simulink model "SimulinkAnalysisofCheetahTail"  (R2022a)
(part 8 of 21)

t4317 = ct{1188};
t4318 = ct{1189};
t4319 = ct{1190};
t4320 = ct{1191};
t4321 = ct{1192};
t4322 = ct{1193};
t4323 = ct{1194};
t4324 = ct{1195};
t4326 = ct{1196};
t4327 = ct{1197};
t4329 = ct{1198};
t433 = ct{1199};
t4330 = ct{1200};
t4331 = ct{1201};
t4332 = ct{1202};
t4333 = ct{1203};
t4334 = ct{1204};
t4337 = ct{1205};
t4339 = ct{1206};
t4340 = ct{1207};
t4341 = ct{1208};
t4342 = ct{1209};
t4343 = ct{1210};
t4344 = ct{1211};
t4345 = ct{1212};
t4346 = ct{1213};
t4348 = ct{1214};
t4349 = ct{1215};
t4350 = ct{1216};
t4352 = ct{1217};
t4354 = ct{1218};
t4355 = ct{1219};
t4356 = ct{1220};
t4357 = ct{1221};
t4358 = ct{1222};
t4359 = ct{1223};
t436 = ct{1224};
t4360 = ct{1225};
t4361 = ct{1226};
t4365 = ct{1227};
t4367 = ct{1228};
t4368 = ct{1229};
t4369 = ct{1230};
t4370 = ct{1231};
t4371 = ct{1232};
t4372 = ct{1233};
t4373 = ct{1234};
t4374 = ct{1235};
t4375 = ct{1236};
t4376 = ct{1237};
t4378 = ct{1238};
t4379 = ct{1239};
t4382 = ct{1240};
t4384 = ct{1241};
t4391 = ct{1242};
t4392 = ct{1243};
t4393 = ct{1244};
t4394 = ct{1245};
t4395 = ct{1246};
t4397 = ct{1247};
t4398 = ct{1248};
t4399 = ct{1249};
t44 = ct{1250};
t4400 = ct{1251};
t4401 = ct{1252};
t4402 = ct{1253};
t4403 = ct{1254};
t4404 = ct{1255};
t4406 = ct{1256};
t4407 = ct{1257};
t4408 = ct{1258};
t4409 = ct{1259};
t4412 = ct{1260};
t4414 = ct{1261};
t4415 = ct{1262};
t4416 = ct{1263};
t4418 = ct{1264};
t4420 = ct{1265};
t4421 = ct{1266};
t4422 = ct{1267};
t4424 = ct{1268};
t4425 = ct{1269};
t4427 = ct{1270};
t4428 = ct{1271};
t4429 = ct{1272};
t4431 = ct{1273};
t4432 = ct{1274};
t4434 = ct{1275};
t4435 = ct{1276};
t4437 = ct{1277};
t4438 = ct{1278};
t4439 = ct{1279};
t4440 = ct{1280};
t4442 = ct{1281};
t4443 = ct{1282};
t4444 = ct{1283};
t4447 = ct{1284};
t4448 = ct{1285};
t4449 = ct{1286};
t445 = ct{1287};
t4450 = ct{1288};
t4451 = ct{1289};
t4452 = ct{1290};
t4453 = ct{1291};
t4454 = ct{1292};
t4455 = ct{1293};
t4456 = ct{1294};
t4457 = ct{1295};
t4458 = ct{1296};
t4459 = ct{1297};
t4460 = ct{1298};
t4461 = ct{1299};
t4462 = ct{1300};
t4463 = ct{1301};
t4465 = ct{1302};
t4467 = ct{1303};
t4469 = ct{1304};
t4470 = ct{1305};
t4471 = ct{1306};
t4472 = ct{1307};
t4473 = ct{1308};
t4475 = ct{1309};
t4476 = ct{1310};
t4477 = ct{1311};
t4479 = ct{1312};
t4480 = ct{1313};
t4481 = ct{1314};
t4482 = ct{1315};
t4483 = ct{1316};
t4484 = ct{1317};
t4485 = ct{1318};
t4486 = ct{1319};
t4487 = ct{1320};
t4488 = ct{1321};
t4489 = ct{1322};
t4490 = ct{1323};
t4492 = ct{1324};
t4493 = ct{1325};
t4495 = ct{1326};
t4496 = ct{1327};
t4497 = ct{1328};
t4498 = ct{1329};
t4500 = ct{1330};
t4501 = ct{1331};
t4502 = ct{1332};
t4503 = ct{1333};
t4505 = ct{1334};
t4506 = ct{1335};
t4507 = ct{1336};
t451 = ct{1337};
t4510 = ct{1338};
t4511 = ct{1339};
t4512 = ct{1340};
t4514 = ct{1341};
t4515 = ct{1342};
t4517 = ct{1343};
t4518 = ct{1344};
t4519 = ct{1345};
t4521 = ct{1346};
t4522 = ct{1347};
t4523 = ct{1348};
t4525 = ct{1349};
t4526 = ct{1350};
t4528 = ct{1351};
t4529 = ct{1352};
t4531 = ct{1353};
t4532 = ct{1354};
t4533 = ct{1355};
t4535 = ct{1356};
t4536 = ct{1357};
t4537 = ct{1358};
t4538 = ct{1359};
t4540 = ct{1360};
t4541 = ct{1361};
t4542 = ct{1362};
t4543 = ct{1363};
t4544 = ct{1364};
t4545 = ct{1365};
t4546 = ct{1366};
t4547 = ct{1367};
t4549 = ct{1368};
t4550 = ct{1369};
t4551 = ct{1370};
t4552 = ct{1371};
t4553 = ct{1372};
t4554 = ct{1373};
t4555 = ct{1374};
t4556 = ct{1375};
t4557 = ct{1376};
t4558 = ct{1377};
t4559 = ct{1378};
t4560 = ct{1379};
t4561 = ct{1380};
t4562 = ct{1381};
t4565 = ct{1382};
t4566 = ct{1383};
t4567 = ct{1384};
t4568 = ct{1385};
t4570 = ct{1386};
t4571 = ct{1387};
t4573 = ct{1388};
t4574 = ct{1389};
t4575 = ct{1390};
t4576 = ct{1391};
t4577 = ct{1392};
t4578 = ct{1393};
t4579 = ct{1394};
t4580 = ct{1395};
t4581 = ct{1396};
t4582 = ct{1397};
t4583 = ct{1398};
t4584 = ct{1399};
t4585 = ct{1400};
t4586 = ct{1401};
t4588 = ct{1402};
t459 = ct{1403};
t4590 = ct{1404};
t4591 = ct{1405};
t4592 = ct{1406};
t4596 = ct{1407};
t4597 = ct{1408};
t4598 = ct{1409};
t4600 = ct{1410};
t4601 = ct{1411};
t4602 = ct{1412};
t4603 = ct{1413};
t4604 = ct{1414};
t4605 = ct{1415};
t4606 = ct{1416};
t4607 = ct{1417};
t4608 = ct{1418};
t4609 = ct{1419};
t4610 = ct{1420};
t4613 = ct{1421};
t4614 = ct{1422};
t4615 = ct{1423};
t4616 = ct{1424};
t4617 = ct{1425};
t4618 = ct{1426};
t4619 = ct{1427};
t4620 = ct{1428};
t4621 = ct{1429};
t4622 = ct{1430};
t4623 = ct{1431};
t4624 = ct{1432};
t4625 = ct{1433};
t4626 = ct{1434};
t4629 = ct{1435};
t4630 = ct{1436};
t4631 = ct{1437};
t4634 = ct{1438};
t4635 = ct{1439};
t4636 = ct{1440};
t4637 = ct{1441};
t4638 = ct{1442};
t4639 = ct{1443};
t4640 = ct{1444};
t4644 = ct{1445};
t4645 = ct{1446};
t4646 = ct{1447};
t4647 = ct{1448};
t4648 = ct{1449};
t4649 = ct{1450};
t465 = ct{1451};
t4650 = ct{1452};
t4651 = ct{1453};
t4652 = ct{1454};
t4655 = ct{1455};
t4656 = ct{1456};
t4657 = ct{1457};
t4658 = ct{1458};
t4659 = ct{1459};
t4660 = ct{1460};
t4661 = ct{1461};
t4662 = ct{1462};
t4663 = ct{1463};
t4664 = ct{1464};
t4665 = ct{1465};
t4666 = ct{1466};
t4667 = ct{1467};
t4668 = ct{1468};
t4669 = ct{1469};
t4672 = ct{1470};
t4673 = ct{1471};
t4674 = ct{1472};
t4675 = ct{1473};
t4678 = ct{1474};
t4679 = ct{1475};
t4680 = ct{1476};
t4681 = ct{1477};
t4682 = ct{1478};
t4684 = ct{1479};
t4685 = ct{1480};
t4686 = ct{1481};
t4689 = ct{1482};
t4690 = ct{1483};
t4691 = ct{1484};
t4693 = ct{1485};
t4694 = ct{1486};
t4695 = ct{1487};
t4696 = ct{1488};
t4697 = ct{1489};
t4698 = ct{1490};
t4700 = ct{1491};
t4701 = ct{1492};
t4702 = ct{1493};
t4704 = ct{1494};
t4705 = ct{1495};
t4706 = ct{1496};
t4707 = ct{1497};
t4708 = ct{1498};
t4709 = ct{1499};
t4710 = ct{1500};
t4711 = ct{1501};
t4712 = ct{1502};
t4713 = ct{1503};
t4722 = ct{1504};
t4723 = ct{1505};
t4724 = ct{1506};
t4727 = ct{1507};
t4729 = ct{1508};
t4732 = ct{1509};
t4733 = ct{1510};
t4735 = ct{1511};
t4736 = ct{1512};
t4737 = ct{1513};
t4738 = ct{1514};
t4742 = ct{1515};
t4750 = ct{1516};
t4751 = ct{1517};
t4752 = ct{1518};
t4753 = ct{1519};
t4755 = ct{1520};
t4756 = ct{1521};
t4758 = ct{1522};
t4759 = ct{1523};
t4761 = ct{1524};
t4764 = ct{1525};
t4765 = ct{1526};
t4769 = ct{1527};
t4770 = ct{1528};
t4771 = ct{1529};
t4772 = ct{1530};
t4773 = ct{1531};
t4775 = ct{1532};
t4776 = ct{1533};
t4780 = ct{1534};
t4783 = ct{1535};
t4784 = ct{1536};
t4785 = ct{1537};
t4786 = ct{1538};
t4787 = ct{1539};
t4788 = ct{1540};
t4789 = ct{1541};
t4790 = ct{1542};
t4791 = ct{1543};
t4793 = ct{1544};
t4796 = ct{1545};
t4797 = ct{1546};
t4799 = ct{1547};
t48 = ct{1548};
t4800 = ct{1549};
t4801 = ct{1550};
t4802 = ct{1551};
t4803 = ct{1552};
t4804 = ct{1553};
t4805 = ct{1554};
t4806 = ct{1555};
t4807 = ct{1556};
t4809 = ct{1557};
t4811 = ct{1558};
t4813 = ct{1559};
t4814 = ct{1560};
t4815 = ct{1561};
t4816 = ct{1562};
t4819 = ct{1563};
t4820 = ct{1564};
t4821 = ct{1565};
t4823 = ct{1566};
t4826 = ct{1567};
t4827 = ct{1568};
t4830 = ct{1569};
t4832 = ct{1570};
t4834 = ct{1571};
t4835 = ct{1572};
t4836 = ct{1573};
t4838 = ct{1574};
t4840 = ct{1575};
t4841 = ct{1576};
t4843 = ct{1577};
t4845 = ct{1578};
t4846 = ct{1579};
t4847 = ct{1580};
t4848 = ct{1581};
t4849 = ct{1582};
t485 = ct{1583};
t4850 = ct{1584};
t4851 = ct{1585};
t4852 = ct{1586};
t4853 = ct{1587};
t4857 = ct{1588};
t4858 = ct{1589};
t4861 = ct{1590};
t4862 = ct{1591};
t4863 = ct{1592};
t4864 = ct{1593};
t4865 = ct{1594};
t4867 = ct{1595};
t4868 = ct{1596};
t4870 = ct{1597};
t4873 = ct{1598};
t4874 = ct{1599};
t4877 = ct{1600};
t488 = ct{1601};
t4880 = ct{1602};
t4881 = ct{1603};
t4882 = ct{1604};
t4883 = ct{1605};
t4887 = ct{1606};
t4888 = ct{1607};
t4889 = ct{1608};
t4890 = ct{1609};
t4892 = ct{1610};
t4893 = ct{1611};
t4895 = ct{1612};
t4897 = ct{1613};
t4899 = ct{1614};
t49 = ct{1615};
t4900 = ct{1616};
t4901 = ct{1617};
t4904 = ct{1618};
t4906 = ct{1619};
t4907 = ct{1620};
t4908 = ct{1621};
t4909 = ct{1622};
t4911 = ct{1623};
t4912 = ct{1624};
t4913 = ct{1625};
t4914 = ct{1626};
t4916 = ct{1627};
t4917 = ct{1628};
t4922 = ct{1629};
t4923 = ct{1630};
t4924 = ct{1631};
t4925 = ct{1632};
t4926 = ct{1633};
t4927 = ct{1634};
t4928 = ct{1635};
t4929 = ct{1636};
t4931 = ct{1637};
t4932 = ct{1638};
t4933 = ct{1639};
t4934 = ct{1640};
t4936 = ct{1641};
t4937 = ct{1642};
t4938 = ct{1643};
t4939 = ct{1644};
t4940 = ct{1645};
t4941 = ct{1646};
t4942 = ct{1647};
t4943 = ct{1648};
t4944 = ct{1649};
t4945 = ct{1650};
t4946 = ct{1651};
t4947 = ct{1652};
t4949 = ct{1653};
t4950 = ct{1654};
t4951 = ct{1655};
t4952 = ct{1656};
t4953 = ct{1657};
t4954 = ct{1658};
t4955 = ct{1659};
t496 = ct{1660};
t4960 = ct{1661};
t4961 = ct{1662};
t4963 = ct{1663};
t4964 = ct{1664};
t4966 = ct{1665};
t4967 = ct{1666};
t4968 = ct{1667};
t4969 = ct{1668};
t4972 = ct{1669};
t4973 = ct{1670};
t4975 = ct{1671};
t4976 = ct{1672};
t4977 = ct{1673};
t4978 = ct{1674};
t4980 = ct{1675};
t4981 = ct{1676};
t4982 = ct{1677};
t4983 = ct{1678};
t4984 = ct{1679};
t4985 = ct{1680};
t4986 = ct{1681};
t4988 = ct{1682};
t4989 = ct{1683};
t4990 = ct{1684};
t4993 = ct{1685};
t4995 = ct{1686};
t4997 = ct{1687};
t4998 = ct{1688};
t5 = ct{1689};
t50 = ct{1690};
t5000 = ct{1691};
t5001 = ct{1692};
t5002 = ct{1693};
t5004 = ct{1694};
t5005 = ct{1695};
t5006 = ct{1696};
t5007 = ct{1697};
t5008 = ct{1698};
t5009 = ct{1699};
t501 = ct{1700};
t5010 = ct{1701};
t5012 = ct{1702};
t5013 = ct{1703};
t5014 = ct{1704};
t5016 = ct{1705};
t5017 = ct{1706};
t5018 = ct{1707};
t502 = ct{1708};
t5021 = ct{1709};
t5022 = ct{1710};
t5023 = ct{1711};
t5024 = ct{1712};
t5025 = ct{1713};
t5027 = ct{1714};
t5028 = ct{1715};
t5030 = ct{1716};
t5031 = ct{1717};
t5032 = ct{1718};
t5033 = ct{1719};
t5034 = ct{1720};
t5035 = ct{1721};
t5036 = ct{1722};
t5038 = ct{1723};
t5039 = ct{1724};
t504 = ct{1725};
t5040 = ct{1726};
t5041 = ct{1727};
t5042 = ct{1728};
t5045 = ct{1729};
t5046 = ct{1730};
t5047 = ct{1731};
t5048 = ct{1732};
t5049 = ct{1733};
t5050 = ct{1734};
t5051 = ct{1735};
t5052 = ct{1736};
t5053 = ct{1737};
t5054 = ct{1738};
t5055 = ct{1739};
t5057 = ct{1740};
t5058 = ct{1741};
t5059 = ct{1742};
t5061 = ct{1743};
t5062 = ct{1744};
t5063 = ct{1745};
t5064 = ct{1746};
t5066 = ct{1747};
t5067 = ct{1748};
t5068 = ct{1749};
t5069 = ct{1750};
t5071 = ct{1751};
t5072 = ct{1752};
t5074 = ct{1753};
t5075 = ct{1754};
t5076 = ct{1755};
t5077 = ct{1756};
t5078 = ct{1757};
t5079 = ct{1758};
t5080 = ct{1759};
t5082 = ct{1760};
t5083 = ct{1761};
t5084 = ct{1762};
t5085 = ct{1763};
t5087 = ct{1764};
t5088 = ct{1765};
t5089 = ct{1766};
t5090 = ct{1767};
t5092 = ct{1768};
t5093 = ct{1769};
t5094 = ct{1770};
t5095 = ct{1771};
t5098 = ct{1772};
t5099 = ct{1773};
t51 = ct{1774};
t5100 = ct{1775};
t5101 = ct{1776};
t5102 = ct{1777};
t5103 = ct{1778};
t5104 = ct{1779};
t5106 = ct{1780};
t5107 = ct{1781};
t5109 = ct{1782};
t5110 = ct{1783};
t5111 = ct{1784};
t5112 = ct{1785};
t5114 = ct{1786};
t5115 = ct{1787};
t5117 = ct{1788};
t5118 = ct{1789};
t5120 = ct{1790};
t5121 = ct{1791};
t5123 = ct{1792};
t5124 = ct{1793};
t5126 = ct{1794};
t5128 = ct{1795};
t5131 = ct{1796};
t5132 = ct{1797};
t5134 = ct{1798};
t5135 = ct{1799};
t5136 = ct{1800};
t5137 = ct{1801};
t5138 = ct{1802};
t5139 = ct{1803};
t5140 = ct{1804};
t5142 = ct{1805};
t5143 = ct{1806};
t5144 = ct{1807};
t5145 = ct{1808};
t5146 = ct{1809};
t5148 = ct{1810};
t5149 = ct{1811};
t5150 = ct{1812};
t5152 = ct{1813};
t5153 = ct{1814};
t5154 = ct{1815};
t5155 = ct{1816};
t5156 = ct{1817};
t5157 = ct{1818};
t5158 = ct{1819};
t5161 = ct{1820};
t5162 = ct{1821};
t5163 = ct{1822};
t5165 = ct{1823};
t5166 = ct{1824};
t5167 = ct{1825};
t5168 = ct{1826};
t5169 = ct{1827};
t5171 = ct{1828};
t5172 = ct{1829};
t5173 = ct{1830};
t5174 = ct{1831};
t5175 = ct{1832};
t5177 = ct{1833};
t5178 = ct{1834};
t5179 = ct{1835};
t5180 = ct{1836};
t5182 = ct{1837};
t5183 = ct{1838};
t5184 = ct{1839};
t5185 = ct{1840};
t5186 = ct{1841};
t5187 = ct{1842};
t5188 = ct{1843};
t519 = ct{1844};
t5190 = ct{1845};
t5191 = ct{1846};
t5193 = ct{1847};
t5194 = ct{1848};
t5196 = ct{1849};
t5197 = ct{1850};
t5198 = ct{1851};
t5199 = ct{1852};
t5202 = ct{1853};
t5203 = ct{1854};
t5204 = ct{1855};
t5205 = ct{1856};
t5206 = ct{1857};
t5207 = ct{1858};
t5208 = ct{1859};
t5211 = ct{1860};
t5212 = ct{1861};
t5214 = ct{1862};
t5216 = ct{1863};
t5217 = ct{1864};
t5218 = ct{1865};
t5220 = ct{1866};
t5221 = ct{1867};
t5223 = ct{1868};
t5224 = ct{1869};
t5225 = ct{1870};
t5226 = ct{1871};
t5227 = ct{1872};
t5228 = ct{1873};
t5229 = ct{1874};
t523 = ct{1875};
t5231 = ct{1876};
t5232 = ct{1877};
t5233 = ct{1878};
t5234 = ct{1879};
t5235 = ct{1880};
t5238 = ct{1881};
t5239 = ct{1882};
t524 = ct{1883};
t5240 = ct{1884};
t5241 = ct{1885};
t5243 = ct{1886};
t5244 = ct{1887};
t5245 = ct{1888};
t5247 = ct{1889};
t5248 = ct{1890};
t5249 = ct{1891};
t5250 = ct{1892};
t5251 = ct{1893};
t5252 = ct{1894};
t5253 = ct{1895};
t5254 = ct{1896};
t5256 = ct{1897};
t5259 = ct{1898};
t5260 = ct{1899};
t5262 = ct{1900};
t5263 = ct{1901};
t5264 = ct{1902};
t5265 = ct{1903};
t5266 = ct{1904};
t5268 = ct{1905};
t5269 = ct{1906};
t527 = ct{1907};
t5270 = ct{1908};
t5272 = ct{1909};
t5274 = ct{1910};
t5275 = ct{1911};
t5276 = ct{1912};
t5277 = ct{1913};
t5279 = ct{1914};
t5280 = ct{1915};
t5281 = ct{1916};
t5284 = ct{1917};
t5285 = ct{1918};
t5286 = ct{1919};
t5287 = ct{1920};
t5288 = ct{1921};
t5289 = ct{1922};
t5290 = ct{1923};
t5291 = ct{1924};
t5292 = ct{1925};
t5293 = ct{1926};
t5294 = ct{1927};
t5295 = ct{1928};
t5296 = ct{1929};
t5297 = ct{1930};
t5298 = ct{1931};
t5299 = ct{1932};
t530 = ct{1933};
t5300 = ct{1934};
t5301 = ct{1935};
t5302 = ct{1936};
t5304 = ct{1937};
t5305 = ct{1938};
t5306 = ct{1939};
t5307 = ct{1940};
t5308 = ct{1941};
t5309 = ct{1942};
t5310 = ct{1943};
t5311 = ct{1944};
t5312 = ct{1945};
t5313 = ct{1946};
t5314 = ct{1947};
t5316 = ct{1948};
t5317 = ct{1949};
t5318 = ct{1950};
t5319 = ct{1951};
t5321 = ct{1952};
t5322 = ct{1953};
t5324 = ct{1954};
t5325 = ct{1955};
t5326 = ct{1956};
t5327 = ct{1957};
t5328 = ct{1958};
t5329 = ct{1959};
t5330 = ct{1960};
t5332 = ct{1961};
t5333 = ct{1962};
t5335 = ct{1963};
t5336 = ct{1964};
t5337 = ct{1965};
t5338 = ct{1966};
t5339 = ct{1967};
t534 = ct{1968};
t5340 = ct{1969};
t5341 = ct{1970};
t5343 = ct{1971};
t5344 = ct{1972};
t5345 = ct{1973};
t5346 = ct{1974};
t5347 = ct{1975};
t5349 = ct{1976};
t5350 = ct{1977};
t5351 = ct{1978};
t5352 = ct{1979};
t5353 = ct{1980};
t5354 = ct{1981};
t5356 = ct{1982};
t5357 = ct{1983};
t5358 = ct{1984};
t5359 = ct{1985};
t5360 = ct{1986};
t5361 = ct{1987};
t5363 = ct{1988};
t5364 = ct{1989};
t5366 = ct{1990};
t5368 = ct{1991};
t5369 = ct{1992};
t537 = ct{1993};
t5370 = ct{1994};
t5371 = ct{1995};
t5372 = ct{1996};
t5374 = ct{1997};
t5376 = ct{1998};
t5377 = ct{1999};
t5378 = ct{2000};
t5379 = ct{2001};
t5380 = ct{2002};
t5381 = ct{2003};
t5382 = ct{2004};
t5383 = ct{2005};
t5384 = ct{2006};
t5385 = ct{2007};
t5386 = ct{2008};
t5388 = ct{2009};
t5389 = ct{2010};
t539 = ct{2011};
t5391 = ct{2012};
t5392 = ct{2013};
t5393 = ct{2014};
t5394 = ct{2015};
t5395 = ct{2016};
t5396 = ct{2017};
t5398 = ct{2018};
t5399 = ct{2019};
t54 = ct{2020};
t5400 = ct{2021};
t5402 = ct{2022};
t5403 = ct{2023};
t5404 = ct{2024};
t5405 = ct{2025};
t5406 = ct{2026};
t5407 = ct{2027};
t5408 = ct{2028};
t5409 = ct{2029};
t541 = ct{2030};
t5411 = ct{2031};
t5412 = ct{2032};
t5413 = ct{2033};
t5414 = ct{2034};
t5415 = ct{2035};
t5416 = ct{2036};
t5417 = ct{2037};
t5418 = ct{2038};
t5419 = ct{2039};
t542 = ct{2040};
t5420 = ct{2041};
t5421 = ct{2042};
t5422 = ct{2043};
t5423 = ct{2044};
t5425 = ct{2045};
t5426 = ct{2046};
t5427 = ct{2047};
t5428 = ct{2048};
t5430 = ct{2049};
t5431 = ct{2050};
t5434 = ct{2051};
t5435 = ct{2052};
t5436 = ct{2053};
t5438 = ct{2054};
t5439 = ct{2055};
t544 = ct{2056};
t5441 = ct{2057};
t5442 = ct{2058};
t5443 = ct{2059};
t5444 = ct{2060};
t5447 = ct{2061};
t5448 = ct{2062};
t5449 = ct{2063};
t5450 = ct{2064};
t5452 = ct{2065};
t5453 = ct{2066};
t5455 = ct{2067};
t5456 = ct{2068};
t5458 = ct{2069};
t5459 = ct{2070};
t546 = ct{2071};
t5460 = ct{2072};
t5461 = ct{2073};
t5462 = ct{2074};
t5463 = ct{2075};
t5464 = ct{2076};
t5465 = ct{2077};
t5467 = ct{2078};
t5468 = ct{2079};
t5470 = ct{2080};
t5471 = ct{2081};
t5474 = ct{2082};
t5475 = ct{2083};
t5476 = ct{2084};
t5478 = ct{2085};
t5480 = ct{2086};
t5481 = ct{2087};
t5483 = ct{2088};
t5484 = ct{2089};
t5486 = ct{2090};
t5487 = ct{2091};
t5488 = ct{2092};
t5489 = ct{2093};
t5490 = ct{2094};
t5492 = ct{2095};
t5493 = ct{2096};
t5494 = ct{2097};
t5495 = ct{2098};
t5496 = ct{2099};
t5497 = ct{2100};
t5498 = ct{2101};
t5499 = ct{2102};
t55 = ct{2103};
t550 = ct{2104};
t5500 = ct{2105};
t5502 = ct{2106};
t5508 = ct{2107};
t5509 = ct{2108};
t5510 = ct{2109};
t5511 = ct{2110};
t5513 = ct{2111};
t5514 = ct{2112};
t5515 = ct{2113};
t5516 = ct{2114};
t5519 = ct{2115};
t5520 = ct{2116};
t5521 = ct{2117};
t5523 = ct{2118};
t5524 = ct{2119};
t5527 = ct{2120};
t5528 = ct{2121};
t553 = ct{2122};
t5530 = ct{2123};
t5531 = ct{2124};
t5532 = ct{2125};
t5533 = ct{2126};
t5534 = ct{2127};
t5535 = ct{2128};
t5536 = ct{2129};
t5538 = ct{2130};
t5539 = ct{2131};
t5541 = ct{2132};
t5542 = ct{2133};
t5543 = ct{2134};
t5544 = ct{2135};
t5545 = ct{2136};
t5546 = ct{2137};
t5547 = ct{2138};
t5548 = ct{2139};
t5549 = ct{2140};
t5551 = ct{2141};
t5552 = ct{2142};
t5553 = ct{2143};
t5554 = ct{2144};
t5555 = ct{2145};
t5556 = ct{2146};
t5557 = ct{2147};
t5558 = ct{2148};
t5560 = ct{2149};
t5561 = ct{2150};
t5565 = ct{2151};
t5566 = ct{2152};
t5569 = ct{2153};
t557 = ct{2154};
t5570 = ct{2155};
t5571 = ct{2156};
t5573 = ct{2157};
t5574 = ct{2158};
t5575 = ct{2159};
t5576 = ct{2160};
t5577 = ct{2161};
t5578 = ct{2162};
t558 = ct{2163};
t5581 = ct{2164};
t5582 = ct{2165};
t5584 = ct{2166};
t5585 = ct{2167};
t5586 = ct{2168};
t5588 = ct{2169};
t5589 = ct{2170};
t5590 = ct{2171};
t5591 = ct{2172};
t5592 = ct{2173};
t5593 = ct{2174};
t5594 = ct{2175};
t5597 = ct{2176};
t5598 = ct{2177};
t5599 = ct{2178};
t56 = ct{2179};
t5600 = ct{2180};
t5601 = ct{2181};
t5602 = ct{2182};
t5603 = ct{2183};
t5604 = ct{2184};
t5606 = ct{2185};
t5607 = ct{2186};
t5609 = ct{2187};
t5611 = ct{2188};
t5613 = ct{2189};
t5615 = ct{2190};
t5616 = ct{2191};
t5617 = ct{2192};
t5618 = ct{2193};
t5619 = ct{2194};
t5620 = ct{2195};
t5621 = ct{2196};
t5622 = ct{2197};
t5623 = ct{2198};
t5624 = ct{2199};
t5625 = ct{2200};
t5627 = ct{2201};
t5628 = ct{2202};
t5629 = ct{2203};
t5630 = ct{2204};
t5631 = ct{2205};
t5632 = ct{2206};
t5633 = ct{2207};
t5634 = ct{2208};
t5635 = ct{2209};
t5636 = ct{2210};
t5637 = ct{2211};
t5638 = ct{2212};
t5640 = ct{2213};
t5641 = ct{2214};
t5642 = ct{2215};
t5643 = ct{2216};
t5644 = ct{2217};
t5648 = ct{2218};
t5649 = ct{2219};
t5653 = ct{2220};
t5656 = ct{2221};
t5657 = ct{2222};
t5658 = ct{2223};
t5659 = ct{2224};
t5660 = ct{2225};
t5661 = ct{2226};
t5663 = ct{2227};
t5664 = ct{2228};
t5665 = ct{2229};
t5667 = ct{2230};
t5668 = ct{2231};
t5669 = ct{2232};
t5670 = ct{2233};
t5672 = ct{2234};
t5674 = ct{2235};
t5675 = ct{2236};
t5677 = ct{2237};
t5678 = ct{2238};
t5679 = ct{2239};
t5681 = ct{2240};
t5682 = ct{2241};
t5683 = ct{2242};
t5684 = ct{2243};
t5685 = ct{2244};
t5687 = ct{2245};
t5688 = ct{2246};
t5689 = ct{2247};
t5690 = ct{2248};
t5691 = ct{2249};
t5692 = ct{2250};
t5694 = ct{2251};
t5695 = ct{2252};
t5696 = ct{2253};
t5697 = ct{2254};
t5698 = ct{2255};
t5699 = ct{2256};
t5700 = ct{2257};
t5701 = ct{2258};
t5704 = ct{2259};
t5705 = ct{2260};
t5706 = ct{2261};
t5707 = ct{2262};
t5709 = ct{2263};
t5711 = ct{2264};
t5712 = ct{2265};
t5713 = ct{2266};
t5714 = ct{2267};
t5715 = ct{2268};
t5717 = ct{2269};
t5718 = ct{2270};
t5719 = ct{2271};
t5720 = ct{2272};
t5723 = ct{2273};
t5724 = ct{2274};
t5725 = ct{2275};
t5726 = ct{2276};
t5727 = ct{2277};
t5728 = ct{2278};
t5729 = ct{2279};
t573 = ct{2280};
t5730 = ct{2281};
t5731 = ct{2282};
t5732 = ct{2283};
t5733 = ct{2284};
t5734 = ct{2285};
t5735 = ct{2286};
t5737 = ct{2287};
t5738 = ct{2288};
t5739 = ct{2289};
t574 = ct{2290};
t5742 = ct{2291};
t5743 = ct{2292};
t5745 = ct{2293};
t5746 = ct{2294};
t5748 = ct{2295};
t5749 = ct{2296};
t575 = ct{2297};
t5750 = ct{2298};
t5753 = ct{2299};
t5754 = ct{2300};
t5755 = ct{2301};
t5756 = ct{2302};
t5758 = ct{2303};
t5759 = ct{2304};
t5760 = ct{2305};
t5762 = ct{2306};
t5763 = ct{2307};
t5765 = ct{2308};
t5766 = ct{2309};
t5767 = ct{2310};
t5768 = ct{2311};
t5769 = ct{2312};
t5770 = ct{2313};
t5771 = ct{2314};
t5772 = ct{2315};
t5774 = ct{2316};
t5775 = ct{2317};
t5776 = ct{2318};
t5778 = ct{2319};
t5779 = ct{2320};
t5780 = ct{2321};
t5781 = ct{2322};
t5782 = ct{2323};
t5783 = ct{2324};
t5785 = ct{2325};
t5786 = ct{2326};
t5788 = ct{2327};
t5789 = ct{2328};
t5791 = ct{2329};
t5792 = ct{2330};
t5793 = ct{2331};
t5795 = ct{2332};
t5797 = ct{2333};
t5798 = ct{2334};
t5799 = ct{2335};
t5800 = ct{2336};
t5801 = ct{2337};
t5802 = ct{2338};
t5803 = ct{2339};
t5805 = ct{2340};
t5807 = ct{2341};
t5808 = ct{2342};
t5809 = ct{2343};
t5811 = ct{2344};
t5813 = ct{2345};
t5814 = ct{2346};
t5815 = ct{2347};
t5820 = ct{2348};
t5821 = ct{2349};
t5823 = ct{2350};
t5824 = ct{2351};
t5826 = ct{2352};
t5827 = ct{2353};
t5828 = ct{2354};
t5829 = ct{2355};
t5831 = ct{2356};
t5832 = ct{2357};
t5833 = ct{2358};
t5834 = ct{2359};
t5835 = ct{2360};
t5836 = ct{2361};
t5837 = ct{2362};
t5838 = ct{2363};
t5839 = ct{2364};
t5840 = ct{2365};
t5841 = ct{2366};
t5843 = ct{2367};
t5845 = ct{2368};
t5846 = ct{2369};
t5847 = ct{2370};
t5850 = ct{2371};
t5852 = ct{2372};
t5853 = ct{2373};
t5855 = ct{2374};
t5856 = ct{2375};
t5857 = ct{2376};
t5858 = ct{2377};
t5862 = ct{2378};
t5863 = ct{2379};
t5865 = ct{2380};
t5867 = ct{2381};
t5868 = ct{2382};
t5869 = ct{2383};
t587 = ct{2384};
t5870 = ct{2385};
t5871 = ct{2386};
t5872 = ct{2387};
t5873 = ct{2388};
t5874 = ct{2389};
t5875 = ct{2390};
t5880 = ct{2391};
t5881 = ct{2392};
t5883 = ct{2393};
t5885 = ct{2394};
t5887 = ct{2395};
t5889 = ct{2396};
t5890 = ct{2397};
t5891 = ct{2398};
t5894 = ct{2399};
t5895 = ct{2400};
t5898 = ct{2401};
t59 = ct{2402};
t5901 = ct{2403};
t5902 = ct{2404};
t5904 = ct{2405};
t5905 = ct{2406};
t5908 = ct{2407};
t5909 = ct{2408};
t5910 = ct{2409};
t5911 = ct{2410};
t5912 = ct{2411};
t5913 = ct{2412};
t5914 = ct{2413};
t5915 = ct{2414};
t5916 = ct{2415};
t5917 = ct{2416};
t5919 = ct{2417};
t5920 = ct{2418};
t5921 = ct{2419};
t5924 = ct{2420};
t5925 = ct{2421};
t5926 = ct{2422};
t5928 = ct{2423};
t5930 = ct{2424};
t5932 = ct{2425};
t5933 = ct{2426};
t5935 = ct{2427};
t5936 = ct{2428};
t5937 = ct{2429};
t5938 = ct{2430};
t5939 = ct{2431};
t5941 = ct{2432};
t5945 = ct{2433};
t5946 = ct{2434};
t5947 = ct{2435};
t5948 = ct{2436};
t5949 = ct{2437};
t595 = ct{2438};
t5951 = ct{2439};
t5953 = ct{2440};
t5955 = ct{2441};
t5956 = ct{2442};
t5958 = ct{2443};
t5959 = ct{2444};
t5960 = ct{2445};
t5962 = ct{2446};
t5963 = ct{2447};
t5964 = ct{2448};
t5965 = ct{2449};
t5968 = ct{2450};
t5969 = ct{2451};
t5970 = ct{2452};
t5971 = ct{2453};
t5972 = ct{2454};
t5973 = ct{2455};
t5974 = ct{2456};
t5975 = ct{2457};
t5976 = ct{2458};
t5977 = ct{2459};
t5978 = ct{2460};
t5980 = ct{2461};
t5981 = ct{2462};
t5982 = ct{2463};
t5983 = ct{2464};
t5984 = ct{2465};
t5985 = ct{2466};
t5986 = ct{2467};
t5987 = ct{2468};
t5988 = ct{2469};
t5989 = ct{2470};
t5990 = ct{2471};
t5991 = ct{2472};
t5992 = ct{2473};
t5993 = ct{2474};
t5994 = ct{2475};
t5995 = ct{2476};
t5996 = ct{2477};
t5998 = ct{2478};
t6000 = ct{2479};
t6002 = ct{2480};
t6004 = ct{2481};
t6006 = ct{2482};
t6008 = ct{2483};
t6010 = ct{2484};
t6011 = ct{2485};
t6013 = ct{2486};
t6014 = ct{2487};
t6016 = ct{2488};
t6018 = ct{2489};
t6021 = ct{2490};
t6022 = ct{2491};
t6023 = ct{2492};
t6024 = ct{2493};
t6027 = ct{2494};
t6028 = ct{2495};
t6029 = ct{2496};
t603 = ct{2497};
t6030 = ct{2498};
t6031 = ct{2499};
t6032 = ct{2500};
t6036 = ct{2501};
t6037 = ct{2502};
t6039 = ct{2503};
t6042 = ct{2504};
t6043 = ct{2505};
t6045 = ct{2506};
t6049 = ct{2507};
t6051 = ct{2508};
t6052 = ct{2509};
t6054 = ct{2510};
t6057 = ct{2511};
t6058 = ct{2512};
t6059 = ct{2513};
t6060 = ct{2514};
t6062 = ct{2515};
t6064 = ct{2516};
t6066 = ct{2517};
t6069 = ct{2518};
t6071 = ct{2519};
t6073 = ct{2520};
t6074 = ct{2521};
t6075 = ct{2522};
t6079 = ct{2523};
t6086 = ct{2524};
t6088 = ct{2525};
t6089 = ct{2526};
t6090 = ct{2527};
t6091 = ct{2528};
t6092 = ct{2529};
t6095 = ct{2530};
t6099 = ct{2531};
t61 = ct{2532};
t6101 = ct{2533};
t6103 = ct{2534};
t6104 = ct{2535};
t6105 = ct{2536};
t6106 = ct{2537};
t6110 = ct{2538};
t6113 = ct{2539};
t6114 = ct{2540};
t6116 = ct{2541};
t6117 = ct{2542};
t6118 = ct{2543};
t6124 = ct{2544};
t6125 = ct{2545};
t6127 = ct{2546};
t6128 = ct{2547};
t6129 = ct{2548};
t6137 = ct{2549};
t6138 = ct{2550};
t614 = ct{2551};
t6140 = ct{2552};
t6143 = ct{2553};
t6144 = ct{2554};
t6150 = ct{2555};
t6158 = ct{2556};
t6160 = ct{2557};
t6161 = ct{2558};
t6164 = ct{2559};
t6166 = ct{2560};
t6171 = ct{2561};
t6174 = ct{2562};
t6176 = ct{2563};
t6181 = ct{2564};
t6182 = ct{2565};
t6183 = ct{2566};
t6184 = ct{2567};
t6188 = ct{2568};
t6189 = ct{2569};
t6190 = ct{2570};
t6191 = ct{2571};
t6195 = ct{2572};
t6196 = ct{2573};
t6197 = ct{2574};
t6199 = ct{2575};
t6201 = ct{2576};
t6202 = ct{2577};
t6203 = ct{2578};
t6204 = ct{2579};
t6205 = ct{2580};
t6206 = ct{2581};
t6207 = ct{2582};
t6208 = ct{2583};
t6210 = ct{2584};
t6211 = ct{2585};
t6212 = ct{2586};
t6216 = ct{2587};
t6217 = ct{2588};
t6218 = ct{2589};
t6219 = ct{2590};
t6220 = ct{2591};
t6221 = ct{2592};
t6222 = ct{2593};
t6223 = ct{2594};
t6224 = ct{2595};
t6225 = ct{2596};
t6228 = ct{2597};
t6229 = ct{2598};
t6230 = ct{2599};
t6231 = ct{2600};
t6233 = ct{2601};
t6234 = ct{2602};
t6235 = ct{2603};
t6236 = ct{2604};
t6238 = ct{2605};
t6239 = ct{2606};
t6240 = ct{2607};
t6241 = ct{2608};
t6243 = ct{2609};
t6245 = ct{2610};
t6248 = ct{2611};
t6249 = ct{2612};
t6250 = ct{2613};
t6251 = ct{2614};
t6252 = ct{2615};
t6253 = ct{2616};
t6255 = ct{2617};
t6257 = ct{2618};
t6258 = ct{2619};
t6259 = ct{2620};
t6260 = ct{2621};
t6261 = ct{2622};
t6264 = ct{2623};
t6265 = ct{2624};
t6269 = ct{2625};
t6271 = ct{2626};
t6272 = ct{2627};
t6273 = ct{2628};
t6274 = ct{2629};
t6276 = ct{2630};
t6277 = ct{2631};
t6278 = ct{2632};
t6279 = ct{2633};
t628 = ct{2634};
t6280 = ct{2635};
t6281 = ct{2636};
t6282 = ct{2637};
t6283 = ct{2638};
t6284 = ct{2639};
t6285 = ct{2640};
t6286 = ct{2641};
t6289 = ct{2642};
t629 = ct{2643};
t6290 = ct{2644};
t6293 = ct{2645};
t6294 = ct{2646};
t6295 = ct{2647};
t6296 = ct{2648};
t6298 = ct{2649};
t6299 = ct{2650};
t6302 = ct{2651};
t6303 = ct{2652};
t6304 = ct{2653};
t6305 = ct{2654};
t6307 = ct{2655};
t6309 = ct{2656};
t6310 = ct{2657};
t6311 = ct{2658};
t6314 = ct{2659};
t6315 = ct{2660};
t6316 = ct{2661};
t6317 = ct{2662};
t6319 = ct{2663};
t6322 = ct{2664};
t6323 = ct{2665};
t6324 = ct{2666};
t6325 = ct{2667};
t6328 = ct{2668};
t6330 = ct{2669};
t6332 = ct{2670};
t6333 = ct{2671};
t6334 = ct{2672};
t6335 = ct{2673};
t6336 = ct{2674};
t6337 = ct{2675};
t6339 = ct{2676};
t634 = ct{2677};
t6340 = ct{2678};
t6341 = ct{2679};
t6343 = ct{2680};
t6344 = ct{2681};
t6345 = ct{2682};
t6346 = ct{2683};
t6347 = ct{2684};
t6348 = ct{2685};
t6349 = ct{2686};
t6350 = ct{2687};
t6351 = ct{2688};
t6353 = ct{2689};
t6354 = ct{2690};
t6355 = ct{2691};
t6356 = ct{2692};
t6358 = ct{2693};
t6360 = ct{2694};
t6361 = ct{2695};
t6362 = ct{2696};
t6364 = ct{2697};
t6365 = ct{2698};
t6366 = ct{2699};
t6367 = ct{2700};
t6368 = ct{2701};
t6369 = ct{2702};
t6370 = ct{2703};
t6371 = ct{2704};
t6372 = ct{2705};
t6373 = ct{2706};
t6375 = ct{2707};
t6378 = ct{2708};
t6379 = ct{2709};
t6380 = ct{2710};
t6381 = ct{2711};
t6382 = ct{2712};
t6383 = ct{2713};
t6385 = ct{2714};
t6386 = ct{2715};
t6387 = ct{2716};
t6388 = ct{2717};
t6389 = ct{2718};
t6392 = ct{2719};
t6393 = ct{2720};
t6394 = ct{2721};
t6395 = ct{2722};
t6396 = ct{2723};
t6398 = ct{2724};
t6399 = ct{2725};
t6400 = ct{2726};
t6401 = ct{2727};
t6402 = ct{2728};
t6403 = ct{2729};
t6404 = ct{2730};
t6405 = ct{2731};
t6406 = ct{2732};
t6407 = ct{2733};
t6408 = ct{2734};
t6409 = ct{2735};
t641 = ct{2736};
t6410 = ct{2737};
t6411 = ct{2738};
t6412 = ct{2739};
t6413 = ct{2740};
t6414 = ct{2741};
t6416 = ct{2742};
t6418 = ct{2743};
t6420 = ct{2744};
t6421 = ct{2745};
t6422 = ct{2746};
t6423 = ct{2747};
t6425 = ct{2748};
t6426 = ct{2749};
t6427 = ct{2750};
t6428 = ct{2751};
t6430 = ct{2752};
t6432 = ct{2753};
t6433 = ct{2754};
t6434 = ct{2755};
t6435 = ct{2756};
t6436 = ct{2757};
t6437 = ct{2758};
t6438 = ct{2759};
t6440 = ct{2760};
t6441 = ct{2761};
t6442 = ct{2762};
t6444 = ct{2763};
t6445 = ct{2764};
t6446 = ct{2765};
t6447 = ct{2766};
t6448 = ct{2767};
t6449 = ct{2768};
t6450 = ct{2769};
t6451 = ct{2770};
t6452 = ct{2771};
t6454 = ct{2772};
t6455 = ct{2773};
t6456 = ct{2774};
t6457 = ct{2775};
t6458 = ct{2776};
t6460 = ct{2777};
t6461 = ct{2778};
t6463 = ct{2779};
t6464 = ct{2780};
t6469 = ct{2781};
t6470 = ct{2782};
t6471 = ct{2783};
t6473 = ct{2784};
t6474 = ct{2785};
t6478 = ct{2786};
t6479 = ct{2787};
t6481 = ct{2788};
t6482 = ct{2789};
t6483 = ct{2790};
t6484 = ct{2791};
t6485 = ct{2792};
t6486 = ct{2793};
t6487 = ct{2794};
t6488 = ct{2795};
t6491 = ct{2796};
t6495 = ct{2797};
t6497 = ct{2798};
t6498 = ct{2799};
t6499 = ct{2800};
t65 = ct{2801};
t6500 = ct{2802};
t6501 = ct{2803};
t6503 = ct{2804};
t6504 = ct{2805};
t6505 = ct{2806};
t6506 = ct{2807};
t6507 = ct{2808};
t6508 = ct{2809};
t6509 = ct{2810};
t651 = ct{2811};
t6511 = ct{2812};
t6512 = ct{2813};
t6513 = ct{2814};
t6520 = ct{2815};
t6523 = ct{2816};
t6525 = ct{2817};
t6526 = ct{2818};
t6527 = ct{2819};
t6529 = ct{2820};
t6532 = ct{2821};
t6533 = ct{2822};
t6536 = ct{2823};
t6540 = ct{2824};
t6541 = ct{2825};
t6542 = ct{2826};
t6543 = ct{2827};
t6547 = ct{2828};
t6549 = ct{2829};
t655 = ct{2830};
t6550 = ct{2831};
t6551 = ct{2832};
t6552 = ct{2833};
t6561 = ct{2834};
t6562 = ct{2835};
t6563 = ct{2836};
t6565 = ct{2837};
t6567 = ct{2838};
t6569 = ct{2839};
t657 = ct{2840};
t6571 = ct{2841};
t6572 = ct{2842};
t6577 = ct{2843};
t6578 = ct{2844};
t6580 = ct{2845};
t6581 = ct{2846};
t6583 = ct{2847};
t6584 = ct{2848};
t6588 = ct{2849};
t6590 = ct{2850};
t6591 = ct{2851};
t6592 = ct{2852};
t6593 = ct{2853};
t6598 = ct{2854};
t6602 = ct{2855};
t6603 = ct{2856};
t6604 = ct{2857};
t6605 = ct{2858};
t6607 = ct{2859};
t6608 = ct{2860};
t6609 = ct{2861};
t6610 = ct{2862};
t6611 = ct{2863};
t6612 = ct{2864};
t6613 = ct{2865};
t6614 = ct{2866};
t6615 = ct{2867};
t6616 = ct{2868};
t6617 = ct{2869};
t6618 = ct{2870};
t6619 = ct{2871};
t6620 = ct{2872};
t6631 = ct{2873};
t6632 = ct{2874};
t6634 = ct{2875};
t6635 = ct{2876};
t6636 = ct{2877};
t6637 = ct{2878};
t6638 = ct{2879};
t664 = ct{2880};
t6640 = ct{2881};
t6641 = ct{2882};
t6645 = ct{2883};
t6646 = ct{2884};
t6647 = ct{2885};
t665 = ct{2886};
t6653 = ct{2887};
t6654 = ct{2888};
t6658 = ct{2889};
t6659 = ct{2890};
t666 = ct{2891};
t6661 = ct{2892};
t6664 = ct{2893};
t6666 = ct{2894};
t6668 = ct{2895};
t6669 = ct{2896};
t667 = ct{2897};
t6673 = ct{2898};
t6675 = ct{2899};
t6676 = ct{2900};
t6677 = ct{2901};
t6679 = ct{2902};
t668 = ct{2903};
t6681 = ct{2904};
t6682 = ct{2905};
t6683 = ct{2906};
t6684 = ct{2907};
t6685 = ct{2908};
t6689 = ct{2909};
t669 = ct{2910};
t6690 = ct{2911};
t6691 = ct{2912};
t6693 = ct{2913};
t6694 = ct{2914};
t6699 = ct{2915};
t6700 = ct{2916};
t6701 = ct{2917};
t6702 = ct{2918};
t6703 = ct{2919};
t6704 = ct{2920};
t6706 = ct{2921};
t6709 = ct{2922};
t6710 = ct{2923};
t6713 = ct{2924};
t6714 = ct{2925};
t6715 = ct{2926};
t6716 = ct{2927};
t6718 = ct{2928};
t6720 = ct{2929};
t6721 = ct{2930};
t6722 = ct{2931};
t6723 = ct{2932};
t6724 = ct{2933};
t6725 = ct{2934};
t6727 = ct{2935};
t6728 = ct{2936};
t6729 = ct{2937};
t6730 = ct{2938};
t6731 = ct{2939};
t6732 = ct{2940};
t6733 = ct{2941};
t6734 = ct{2942};
t6736 = ct{2943};
t6737 = ct{2944};
t6738 = ct{2945};
t6740 = ct{2946};
t6741 = ct{2947};
t6742 = ct{2948};
t6743 = ct{2949};
t6744 = ct{2950};
t6745 = ct{2951};
t6746 = ct{2952};
t6747 = ct{2953};
t6748 = ct{2954};
t675 = ct{2955};
t6750 = ct{2956};
t6751 = ct{2957};
t6754 = ct{2958};
t6755 = ct{2959};
t6756 = ct{2960};
t6758 = ct{2961};
t6759 = ct{2962};
t6760 = ct{2963};
t6761 = ct{2964};
t6762 = ct{2965};
t6763 = ct{2966};
t6764 = ct{2967};
t6765 = ct{2968};
t6766 = ct{2969};
t6768 = ct{2970};
t6769 = ct{2971};
t6770 = ct{2972};
t6772 = ct{2973};
t6773 = ct{2974};
t6774 = ct{2975};
t6775 = ct{2976};
t6776 = ct{2977};
t6778 = ct{2978};
t6779 = ct{2979};
t6780 = ct{2980};
t6781 = ct{2981};
t6792 = ct{2982};
t6797 = ct{2983};
t6798 = ct{2984};
t68 = ct{2985};
t693 = ct{2986};
t7 = ct{2987};
t71 = ct{2988};
t721 = ct{2989};
t724 = ct{2990};
t73 = ct{2991};
t731 = ct{2992};
t732 = ct{2993};
t736 = ct{2994};
t741 = ct{2995};
t753 = ct{2996};
t754 = ct{2997};
t755 = ct{2998};
t757 = ct{2999};
t765 = ct{3000};
t769 = ct{3001};
t772 = ct{3002};
t774 = ct{3003};
t776 = ct{3004};
t778 = ct{3005};
t795 = ct{3006};
t797 = ct{3007};
t799 = ct{3008};
t8 = ct{3009};
t802 = ct{3010};
t803 = ct{3011};
t806 = ct{3012};
t817 = ct{3013};
t818 = ct{3014};
t820 = ct{3015};
t828 = ct{3016};
t831 = ct{3017};
t838 = ct{3018};
t843 = ct{3019};
t852 = ct{3020};
t853 = ct{3021};
t855 = ct{3022};
t865 = ct{3023};
t867 = ct{3024};
t868 = ct{3025};
t870 = ct{3026};
t871 = ct{3027};
t872 = ct{3028};
t876 = ct{3029};
t886 = ct{3030};
t888 = ct{3031};
t9 = ct{3032};
t901 = ct{3033};
t902 = ct{3034};
t903 = ct{3035};
t904 = ct{3036};
t907 = ct{3037};
t909 = ct{3038};
t914 = ct{3039};
t925 = ct{3040};
t926 = ct{3041};
t947 = ct{3042};
t949 = ct{3043};
t952 = ct{3044};
t964 = ct{3045};
t972 = ct{3046};
t977 = ct{3047};
t983 = ct{3048};
t991 = ct{3049};
t992 = ct{3050};
t993 = ct{3051};
t994 = ct{3052};
t995 = ct{3053};
t4894 = -t4887;
t4905 = -t4899;
t4918 = -t4916;
t4956 = dphi2.*t4951;
t4957 = dphi2.*t4952;
t4958 = dy.*t4952;
t4959 = dz.*t4951;
t5056 = -t5045;
t5070 = t162+t413+t501+t1071+t1612+t2646+t3262+t3912;
t5091 = -t5079;
t5105 = -t5100;
t5116 = -t5106;
t5122 = -t5110;
t5125 = -t5115;
t5127 = -t5117;
t5130 = -t5124;
t5141 = -t5134;
t5192 = dphi2.*t5183;
t5195 = dx.*t5187;
t5209 = ITail.*t3938.*t4814;
t5242 = -t5231;
t5255 = dy.*t5252;
t5257 = dz.*t5248;
t5267 = -t5259;
t5273 = -t5264;
t5278 = -t5270;
t5303 = -t5295;
t5315 = -t5307;
t5342 = -t5333;
t5362 = -t5357;
t5365 = t1072+t1952+t2107+t2426+t3992+t4039;
t5375 = dz.*t5366;
t5387 = -t5377;
t5410 = -t5402;
t5479 = -t5471;
t5485 = ITail.*t4408.*t4814;
t5503 = -t5496;
t5504 = -t5497;
t5505 = ITail.*t4447.*t4814;
t5506 = ITail.*t3938.*t5013;
t5507 = -t5500;
t5517 = -t5510;
t5522 = -t5515;
t5559 = ITail.*t4476.*t4814;
t5568 = -t5558;
t5579 = ITail.*t3938.*t5089;
t5587 = -t5577;
t5595 = -t5586;
t5608 = t3471+t4523+t4535;
t5614 = -t5609;
t5645 = -t5635;
t5646 = -t5637;
t5651 = -t5641;
t5654 = -t5643;
t5666 = -t5656;
t5671 = ITail.*t3938.*t5175;
t5673 = -t5665;
t5676 = -t5669;
t5708 = t3938.*t5216;
t5744 = ITail.*t4392.*t5013;
t5747 = -t5743;
t5764 = -t5758;
t5773 = -t5769;
t5777 = ITail.*t4447.*t5013;
t5787 = ITail.*t4392.*t5089;
t5810 = ITail.*t4408.*t5089;
t5812 = -t5803;
t5816 = t3939+t4579+t4600;
t5819 = -t5811;
t5822 = ITail.*t4476.*t5013;
t5825 = -t5821;
t5830 = -t5828;
t5844 = -t5839;
t5849 = ITail.*t4392.*t5175;
t5851 = ITail.*t4476.*t5089;
t5854 = t3967.*t5442;
t5861 = -t5856;
t5864 = ITail.*t4408.*t5175;
t5876 = ITail.*t4447.*t5175;
t5877 = t4173.*t5394;
t5879 = -t5873;
t5886 = t4408.*t5216;
t5892 = t4447.*t5216;
t5896 = t4255.*t5394;
t5899 = t4162.*t5442;
t5900 = t4164.*t5442;
t5918 = t4237.*t5442;
t5922 = t4476.*t5216;
t5927 = t4311.*t5394;
t5929 = -t5920;
t5931 = -t5924;
t5942 = -t5937;
t5950 = t59+t410+t504+t2410+t3827+t4000+t4126+t4359;
t5952 = t162+t413+t501+t2376+t3802+t3960+t4147+t4369;
t5954 = -t5951;
t5957 = -t5955;
t5961 = t4382.*t5394;
t5979 = -t5978;
t5997 = t4240+t4693+t4705;
t5999 = t4454.*t5442;
t6007 = -t6002;
t6012 = -t5442.*(-t1018+t1426+t1431-t1446+t3.*t496.*(t105-t465));
t6020 = dx.*t6016;
t6025 = t3938.*t5799;
t6033 = t4592.*t5394;
t6034 = -t6032;
t6040 = t4575.*t5442;
t6041 = t4618.*t5394;
t6044 = t4581.*t5442;
t6046 = -t6043;
t6048 = -t5442.*(t1019-t1651+t1702+t3.*t818.*(t105-t465)+t3.*t872.*(t103-t544));
t6050 = t4645.*t5394;
t6053 = t3938.*t5853;
t6061 = -t6059;
t6063 = t4638.*t5442;
t6065 = -t5442.*(t1751+t2308+t964.*(t105-t465)+t1430.*(t103-t544));
t6068 = -t6064;
t6070 = -t5394.*(t995+t1064-t1506+t1598-t1763-t1774);
t6072 = -t5394.*(t820+t1121-t1435+t1997+t2000+t11.*t420.*(t214-t541));
t6076 = t4672.*t5442;
t6077 = t4686.*t5442;
t6080 = t4695.*t5442;
t6082 = -t5394.*(t1064+t1137-t1694+t1698-t1763-t1774);
t6084 = -t5442.*(t1260-t1328-t1427-t1441+t1706+t9.*t870.*(t105-t465));
t6085 = t5394.*(t1064+t1137-t1694+t1698-t1763-t1774);
t6087 = -t5394.*(t867+t1059-t1646-t1705+t1938-t2002);
t6093 = t4738.*t5394;
t6094 = -t6088;
t6096 = t4392.*t5799;
t6097 = -t5442.*(t753+t991-t1771-t1957+t1181.*(t105-t465)+t11.*t381.*(t534-t546));
t6100 = -t6095;
t6102 = t992+t1280+t1303+t2336+t2996+t3027+t5187;
t6107 = -dth1.*(t4873-t5187);
t6108 = t4408.*t5799;
t6109 = -t6103;
t6112 = dth1.*(t4873-t5187);
t6115 = t4770.*t5394;
t6119 = -t5434.*(t2436-t2536+t1510.*(t197-t537)+t1505.*(t214-t541));
t6126 = -t5394.*(t1060+t1138-t1883+t1932+t2088+t1179.*(t103-t544));
t6130 = t4392.*t5853;
t6131 = t4476.*t5799;
t6132 = t4785.*t5434;
t6133 = -t5394.*(t1250-t1261+t1761-t2083-t2111+t1037.*(t103-t544));
t6134 = t4408.*t5853;
t6136 = t5394.*(t1250-t1261+t1761-t2083-t2111+t1037.*(t103-t544));
t6139 = -t5394.*(t1053+t1332+t2368+t817.*(t214-t541)+t977.*(t103-t544)+t1512.*(t105-t465));
t6142 = t5394.*(t1053+t1332+t2368+t817.*(t214-t541)+t977.*(t103-t544)+t1512.*(t105-t465));
t6145 = t4447.*t5853;
t6147 = t4821.*t5434;
t6149 = t4823.*t5434;
t6152 = t4830.*t5434;
t6153 = -t5434.*(-t1129+t1139-t2082+t2110+t2123+t8.*t872.*(t534-t546));
t6154 = t4834.*t5434;
t6155 = t4849.*t5434;
t6156 = t1075+t1840+t1843+t2427+t3920+t3921+t4986;
t6157 = t1078+t1481+t1628+t2397+t3222+t3379+t5252;
t6162 = -t6160;
t6163 = t4897.*t5434;
t6167 = t4922.*t5434;
t6168 = t4923.*t5434;
t6169 = t1135+t2013+t2016+t2526+t4018+t4020+t4968;
t6177 = t4972.*t5434;
t6179 = -t5434.*(t1176-t1366+t2434+t2435-t2899+t1430.*(t539+t641));
t6180 = t5022.*t5434;
t6185 = -t5434.*(t1365-t1443+t2829-t2831-t2833+t1505.*(t534-t546));
t6186 = t5434.*(t1365-t1443+t2829-t2831-t2833+t1505.*(t534-t546));
t6194 = -t6188;
t6209 = t4162.*t6110;
t6213 = -t6206;
t6214 = -t6210;
t6215 = t3961.*t6137;
t6232 = t4277.*t6110;
t6242 = t4313.*t6110;
t6244 = t4173.*t6137;
t6246 = -t6245;
t6247 = -t6137.*(-t1262+t1701+t9.*t868.*(t105-t465));
t6254 = -t6137.*(-t947+t1240.*(t105-t465)+t903.*(t534-t546));
t6262 = -t6260;
t6266 = -t6110.*(-t1331+t2317+t1510.*(t103-t544));
t6270 = t6110.*(-t1331+t2317+t1510.*(t103-t544));
t6288 = t4392.*t6124;
t6297 = t4408.*t6124;
t6301 = -t6298;
t6306 = t4447.*t6124;
t6318 = t4476.*t6124;
t6321 = -t6319;
t6326 = -t6324;
t6327 = -t6325;
t6331 = -t6328;
t6338 = -t6336;
t6342 = -t6340;
t6357 = -t6355;
t6374 = t3906+t3930+t4393+t4402+t4544+t4550;
t6390 = -t6387;
t6415 = -t6412;
t6417 = -t6414;
t6431 = -t6428;
t6453 = -t6452;
t6462 = -t6461;
t6465 = -t6464;
t6472 = t3862+t3907+t4580+t4582+t4588+t4591;
t6475 = dth1.*t6473;
t6476 = dx.*t6474;
t6490 = -t6488;
t6494 = dth1.*(t655+t904+t914+t1525+t1857+t1860-t2589-t3170-t3177-t6016);
t6514 = dth1.*t6511;
t6515 = dz.*t6513;
t6517 = t1415+t1529+t1722+t1779+t3091+t3171+t3954+t3973+t4092+t4109+t4378+t4398;
t6518 = t1458+t1486+t1720+t1778+t3107+t3149+t3949+t3972+t4095+t4104+t4376+t4397;
t6528 = -t6527;
t6530 = -t6529;
t6535 = t3938.*t6456;
t6537 = t3961.*t6458;
t6544 = -t6540;
t6545 = -t6541;
t6546 = -t6543;
t6548 = -t6547;
t6553 = -t6458.*(-t1262+t1701+t9.*t868.*(t105-t465));
t6558 = -t6458.*(-t947+t1240.*(t105-t465)+t903.*(t534-t546));
t6559 = t4277.*t6457;
t6564 = t4313.*t6457;
t6568 = -t6458.*(t1332+t2368+t1512.*(t105-t465));
t6570 = -t6457.*(-t1331+t2317+t1510.*(t103-t544));
t6573 = t6457.*(-t1331+t2317+t1510.*(t103-t544));
t6574 = t4408.*t6456;
t6576 = t4447.*t6456;
t6579 = -t6578;
t6582 = t4476.*t6456;
t6594 = dphi1.*t6590;
t6595 = dphi1.*t6592;
t6596 = dy.*t6591;
t6597 = dz.*t6593;
t6606 = -t6605;
t6633 = dz.*t6631;
t6639 = t3938.*t6608;
t6648 = t4173.*t6604;
t6650 = -t6604.*(-t1262+t1701+t9.*t868.*(t105-t465));
t6651 = t4162.*t6607;
t6655 = dphi1.*t6654;
t6657 = -t6604.*(-t947+t1240.*(t105-t465)+t903.*(t534-t546));
t6662 = -t6659;
t6663 = -t6661;
t6665 = t4277.*t6607;
t6667 = -t6664;
t6671 = -t6668;
t6674 = t4313.*t6607;
t6678 = -t6675;
t6680 = -t6676;
t6687 = -t6684;
t6688 = -t6685;
t6692 = -t6604.*(t1332+t2368+t1512.*(t105-t465));
t6695 = -t6690;
t6696 = -t6691;
t6697 = t4392.*t6608;
t6698 = -t6693;
t6705 = t4447.*t6608;
t6707 = -t6704;
t6708 = -t6706;
t6717 = t4476.*t6608;
t6719 = -t6718;
t6735 = -t6732;
t6749 = -t6746;
t6752 = -t6750;
t6753 = -t6751;
t6771 = -t6769;
t6777 = -t6774;
et27 = t2920+t2927+t3489-t3494+t3722-t3784+t964.*(t105-t465).*3.36554e-3+t977.*(t105-t465).*3.36554e-3+t1430.*(t103-t544).*3.36554e-3+t1512.*(t103-t544).*3.36554e-3;
et28 = t1510.*(t197-t537).*3.372816795e-3+t1505.*(t214-t541).*3.372816795e-3;
et29 = t4170+t4204+t4601+t4622+t4988+t4990+t5007+t5024+t5256+t5358+t5490-t5545-t5592+t5664-t5768-t6029-t6183+t6282+t6340+t6341+t6395+t6550-t6581+t6684+t6693-t6728+t4849.*(t2449.*3.36554e-3+t3490+t3544+t3545-t4001-t4034)+t4408.*(et27+et28)+t4737.*(t2436-t2536+t1510.*(t197-t537)+t1505.*(t214-t541));
et30 = t4408.*(t3716-t3777+t1510.*(t197-t537).*9.52624335e-4+t1505.*(t214-t541).*9.52624335e-4);
et31 = t4162.*(t2202+t2564+t3719+t817.*(t214-t541).*8.56645e-6+t977.*(t103-t544).*8.56645e-6+t1512.*(t105-t465).*8.56645e-6)+t4645.*(-t2621+t3659+t1510.*(t103-t544).*8.56645e-6);
et32 = t5023.*(-t1331+t2317+t1510.*(t103-t544))+t4518.*(t1053+t1332+t2368+t817.*(t214-t541)+t977.*(t103-t544)+t1512.*(t105-t465))+ITail.*t4675.*(-t1331+t2317+t1510.*(t103-t544))+ITail.*t4645.*(-t1412+t2419+(t1510.*(t103-t544))./2.0)+ITail.*t4215.*(t1053+t1332+t2368+t817.*(t214-t541)+t977.*(t103-t544)+t1512.*(t105-t465))+ITail.*t4162.*(t1141+t1386+t2501+(t817.*(t214-t541))./2.0+(t977.*(t103-t544))./2.0+(t1512.*(t105-t465))./2.0)+ITail.*t4452.*(t2436-t2536+t1510.*(t197-t537)+t1505.*(t214-t541));
et33 = ITail.*t4408.*(t2582-t2684+(t1510.*(t197-t537))./2.0+(t1505.*(t214-t541))./2.0);
t6853 = -dth2.*(et29+et30+et31+et32+et33);
et34 = -t1391-t1393+t2778-t2836+t4460+t4465+t4799+t4801+t5100+t5110+t5496-t5631+t5641-t5649+t5760+t5786-t5894-t5909+t5911-t5974+t6095+t6221+t6231+t6369+t6578-t6610+t6773+t4518.*(t867+t1059-t1646-t1705+t1938-t2002)+t4638.*(t1970-t1971+t2487+t3161-t3236-t3794-t3817+t1240.*(t105-t465).*3.372786875e-3+t903.*(t534-t546).*3.372786875e-3);
et35 = t4500.*(t753+t991-t1771-t1957+t1181.*(t105-t465)+t11.*t381.*(t534-t546))+t4162.*(t1692+t1899+t1910+t2152+t2155-t2401-t2936-t2962-t3031-t3147+t3307-t3387+t3582+t3583-t3837+t1430.*(t539+t641).*3.36554e-3+t1181.*(t105-t465).*3.36554e-3+t11.*t381.*(t534-t546).*3.36554e-3);
et36 = t4638.*(-t1974+t1240.*(t105-t465).*9.53094055e-4+t903.*(t534-t546).*9.53094055e-4);
et37 = t4173.*(t1786+t1810+t1964+t2047+t2152-t2401-t2797-t2860-t3076+t3167-t3232-t3278+t3582+t3583-t3837+t1430.*(t539+t641).*3.36554e-3+t1181.*(t105-t465).*3.372786875e-3+t11.*t381.*(t534-t546).*3.372786875e-3);
et38 = t4173.*(t1784+t2057-t3080-t3287+t1181.*(t105-t465).*9.53094055e-4+t11.*t381.*(t534-t546).*9.53094055e-4);
et39 = t4618.*(-t1865+t2158+t2487+t3302-t3390-t3794-t3817+t1240.*(t105-t465).*3.36554e-3+t903.*(t534-t546).*3.36554e-3);
et40 = t4830.*(-t1865+t1970+t2708+t3161-t3236-t3845-t3870+t1240.*(t105-t465).*3.36554e-3+t903.*(t534-t546).*3.36554e-3)+t4989.*(-t947+t1240.*(t105-t465)+t903.*(t534-t546))+t6486.*(-t947+t1240.*(t105-t465)+t903.*(t534-t546))+ITail.*t4667.*(-t947+t1240.*(t105-t465)+t903.*(t534-t546));
et41 = ITail.*t4638.*(-t1017+(t1240.*(t105-t465))./2.0+(t903.*(t534-t546))./2.0)+ITail.*t4215.*(t867+t1059-t1646-t1705+t1938-t2002)+ITail.*t4162.*(t949+t1142-t1730-t1792+t2049-t2139)+ITail.*t4214.*(t753+t991-t1771-t1957+t1181.*(t105-t465)+t11.*t381.*(t534-t546))+ITail.*t4173.*(t865+t1086-t1855-t2076+(t1181.*(t105-t465))./2.0+(t11.*t381.*(t534-t546))./2.0);
t6870 = -dphi1.*(et34+et35+et36+et37+et38+et39+et40+et41);
et42 = -t1939+t2390+t2843-t2877+t3263+t3931+t4054+t4273+t4301-t4324+t4945+t4964+t5300-t5354-t5382+t5627+t5665+t5705-t5738+t5891+t6049-t6286+t6325+t6381-t6445-t6640+t6668-t6734+t4753.*(-t1129+t1139-t2082+t2110+t2123+t8.*t872.*(t534-t546))+t6106.*(-t1129+t1139-t2082+t2110+t2123+t8.*t872.*(t534-t546))+t4313.*(t2208+t2312-t3315+t3347+t3475+t1179.*(t103-t544).*8.56645e-6);
et43 = t4447.*(t2215-t2237+t3424+t3427-t3439+t8.*t872.*(t534-t546).*9.52624335e-4)+t4704.*(t1060+t1138-t1883+t1932+t2088+t1179.*(t103-t544))+t6105.*(t1060+t1138-t1883+t1932+t2088+t1179.*(t103-t544))+t4936.*(-t1262+t1701+t9.*t868.*(t105-t465));
et44 = t4447.*(t1645+t1965+t2072+t2220-t2242-t2409-t2483-t2504-t3093+t3155+t3261+t3432+t3437-t3442+t1179.*(t103-t544).*3.36554e-3+t3.*t575.*(t105-t465).*3.36554e-3+t8.*t872.*(t534-t546).*3.372816795e-3);
et45 = t4454.*(-t2388+t3008+t9.*t868.*(t105-t465).*9.53094055e-4);
et46 = t4313.*(t1645+t2037-t2064+t2156+t2227-t2409-t2483-t2504-t3244+t3270-t3276+t3299+t3312+t3413+t1179.*(t103-t544).*3.367829185e-3+t3.*t575.*(t105-t465).*3.36554e-3+t8.*t872.*(t534-t546).*3.36554e-3)+t6616.*(-t1331+t2317+t1510.*(t103-t544));
et47 = (-t1331+t2317+t1510.*(t103-t544)).*(-t2218+t2342+t3054+t3096+t3121+t3131)+Mt.*(t433-t828+T_cg_H.*(t197-t537)).*(-t130+t436+t523-t657+t769)+ITail.*t4459.*(-t1129+t1139-t2082+t2110+t2123+t8.*t872.*(t534-t546))+ITail.*t4447.*(-t1189+t1195-t2210+t2241+t2248+(t8.*t872.*(t534-t546))./2.0)+ITail.*t4350.*(t1060+t1138-t1883+t1932+t2088+t1179.*(t103-t544))+ITail.*t4313.*(t1143+t1194-t1959+t2038+t2175+(t1179.*(t103-t544))./2.0)+ITail.*t4490.*(-t1262+t1701+t9.*t868.*(t105-t465))+ITail.*t4454.*(-t1355+t1789+(t9.*t868.*(t105-t465))./2.0)+B_cg_H.*Mb.*t11.*t641.*t2563;
t6872 = -dphi1.*(et42+et43+et44+et45+et46+et47);
et48 = t2024+t2390+t3263+t3828-t3856-t3964+t4054+t4301-t4324+t4424-t4431-t5150+t5235+t5260-t5284-t5322+t5558+t5603-t5623+t5628-t5658-t5681+t5856-t5889+t5924-t5956+t6030-t6045-t6367+t6378+t6405+t6428+t6679+t6706+t6718+t6732+t6760+t4695.*(t1970-t1971+t2487+t3161-t3236-t3794-t3817+t1240.*(t105-t465).*3.372786875e-3+t903.*(t534-t546).*3.372786875e-3);
et49 = t4277.*(t1832.*3.36554e-3+t1866.*3.36554e-3+t1983-t2150-t2322+t2339+t2430-t2472+t2479+t2495+t2785+t2803+t2981-t3252+t3311+t3482+t3485+t496.*(t214-t541).*3.367829185e-3)+(-t1262+t1701+t9.*t868.*(t105-t465)).*(-t1806+t2096+t2605+t2717+t3289+t3438);
et50 = t4695.*(-t1974+t1240.*(t105-t465).*9.53094055e-4+t903.*(t534-t546).*9.53094055e-4)+t4686.*(-t2388+t3008+t9.*t868.*(t105-t465).*9.53094055e-4);
et51 = t4823.*(-t1865+t1970+t2708+t3161-t3236-t3845-t3870+t1240.*(t105-t465).*3.36554e-3+t903.*(t534-t546).*3.36554e-3)+(-t947+t1240.*(t105-t465)+t903.*(t534-t546)).*(t2135-t2468+t2699+t2738+t2950+t3105)+ITail.*t4722.*(-t947+t1240.*(t105-t465)+t903.*(t534-t546))+ITail.*t4695.*(-t1017+(t1240.*(t105-t465))./2.0+(t903.*(t534-t546))./2.0);
et52 = ITail.*t4686.*(-t1355+t1789+(t9.*t868.*(t105-t465))./2.0)+B_cg_H.*Mb.*t11.*t641.*t2563;
t6882 = -dth2.*(et48+et49+et50+et51+et52);
et53 = t2024+t2390+t3263+t3828-t3856-t3964+t4054+t4301-t4324+t4424-t4431-t5150+t5235+t5260-t5284-t5322+t5558+t5603-t5623+t5628-t5658-t5681+t5856-t5889+t5924-t5956+t6030-t6045-t6367+t6378+t6405+t6428+t6679+t6706+t6718+t6732+t6760+t4695.*(t1970-t1971+t2487+t3161-t3236-t3794-t3817+t1240.*(t105-t465).*3.372786875e-3+t903.*(t534-t546).*3.372786875e-3);
et54 = t4277.*(t1832.*3.36554e-3+t1866.*3.36554e-3+t1983-t2150-t2322+t2339+t2430-t2472+t2479+t2495+t2785+t2803+t2981-t3252+t3311+t3482+t3485+t496.*(t214-t541).*3.367829185e-3)+(-t1262+t1701+t9.*t868.*(t105-t465)).*(-t1806+t2096+t2605+t2717+t3289+t3438);
et55 = t4695.*(-t1974+t1240.*(t105-t465).*9.53094055e-4+t903.*(t534-t546).*9.53094055e-4)+t4686.*(-t2388+t3008+t9.*t868.*(t105-t465).*9.53094055e-4);
et56 = t4823.*(-t1865+t1970+t2708+t3161-t3236-t3845-t3870+t1240.*(t105-t465).*3.36554e-3+t903.*(t534-t546).*3.36554e-3)+(-t947+t1240.*(t105-t465)+t903.*(t534-t546)).*(t2135-t2468+t2699+t2738+t2950+t3105)+ITail.*t4722.*(-t947+t1240.*(t105-t465)+t903.*(t534-t546))+ITail.*t4695.*(-t1017+(t1240.*(t105-t465))./2.0+(t903.*(t534-t546))./2.0);
et57 = ITail.*t4686.*(-t1355+t1789+(t9.*t868.*(t105-t465))./2.0)+B_cg_H.*Mb.*t11.*t641.*t2563;
t6883 = dth2.*(et53+et54+et55+et56+et57);
et58 = -t1703+t2015+t3449-t3787+t3916+t3923+t3947-t4371-t4401+t4469+t4493+t5371+t5372+t5404+t5405+t5748+t5749+t5781+t5808+t5986+t5988+t5989+t6103-t6433-t6448-t6645+t6646+t6776+t6779+t6090.*(t867+t1059-t1646-t1705+t1938-t2002)+t4787.*(-t1129+t1139-t2082+t2110+t2123+t8.*t872.*(t534-t546));
et59 = t4454.*(t1970-t1971+t2487+t3161-t3236-t3794-t3817+t1240.*(t105-t465).*3.372786875e-3+t903.*(t534-t546).*3.372786875e-3)+t4551.*(t753+t991-t1771-t1957+t1181.*(t105-t465)+t11.*t381.*(t534-t546))+t6089.*(t753+t991-t1771-t1957+t1181.*(t105-t465)+t11.*t381.*(t534-t546));
et60 = t4476.*(t2215-t2237+t3424+t3427-t3439+t8.*t872.*(t534-t546).*9.52624335e-4)+t6091.*(t1176-t1366+t2434+t2435-t2899+t1430.*(t539+t641));
et61 = t4476.*(t1645+t1965+t2072+t2220-t2242-t2409-t2483-t2504-t3093+t3155+t3261+t3432+t3437-t3442+t1179.*(t103-t544).*3.36554e-3+t3.*t575.*(t105-t465).*3.36554e-3+t8.*t872.*(t534-t546).*3.372816795e-3);
et62 = t4454.*(-t1974+t1240.*(t105-t465).*9.53094055e-4+t903.*(t534-t546).*9.53094055e-4);
et63 = t3961.*(t1786+t1810+t1964+t2047+t2152-t2401-t2797-t2860-t3076+t3167-t3232-t3278+t3582+t3583-t3837+t1430.*(t539+t641).*3.36554e-3+t1181.*(t105-t465).*3.372786875e-3+t11.*t381.*(t534-t546).*3.372786875e-3);
et64 = t3961.*(t1784+t2057-t3080-t3287+t1181.*(t105-t465).*9.53094055e-4+t11.*t381.*(t534-t546).*9.53094055e-4)+t4936.*(-t947+t1240.*(t105-t465)+t903.*(t534-t546))+ITail.*t4490.*(-t947+t1240.*(t105-t465)+t903.*(t534-t546))+ITail.*t4454.*(-t1017+(t1240.*(t105-t465))./2.0+(t903.*(t534-t546))./2.0);
et65 = ITail.*t4522.*(-t1129+t1139-t2082+t2110+t2123+t8.*t872.*(t534-t546))+ITail.*t4476.*(-t1189+t1195-t2210+t2241+t2248+(t8.*t872.*(t534-t546))./2.0)+ITail.*t4071.*(t753+t991-t1771-t1957+t1181.*(t105-t465)+t11.*t381.*(t534-t546))+ITail.*t3961.*(t865+t1086-t1855-t2076+(t1181.*(t105-t465))./2.0+(t11.*t381.*(t534-t546))./2.0)+B_cg_H.*Mb.*t11.*t641.*t3206;
t6887 = -dphi1.*(et58+et59+et60+et61+et62+et63+et64+et65);
et66 = t1149-t1344+t1348+t1455+t1896-t1898-t2188+t2196+t2978+t3709-t4169+t4184+t4197+t4307-t4319+t4349+t4545-t4553+t4655-t4662+t5053+t5083-t5198-t5223+t5420-t5565-t5707-t5732+t5791-t5880-t5935-t5941-t5960-t6116+t6347+t6400+t6701-t6703+t6746-t6764+t4681.*(t1064+t1137-t1694+t1698-t1763-t1774)+t4704.*(t867+t1059-t1646-t1705+t1938-t2002)+t6105.*(t867+t1059-t1646-t1705+t1938-t2002)+t6104.*(t753+t991-t1771-t1957+t1181.*(t105-t465)+t11.*t381.*(t534-t546));
et67 = t4313.*(t1692+t1899+t1910+t2152+t2155-t2401-t2936-t2962-t3031-t3147+t3307-t3387+t3582+t3583-t3837+t1430.*(t539+t641).*3.36554e-3+t1181.*(t105-t465).*3.36554e-3+t11.*t381.*(t534-t546).*3.36554e-3);
et68 = t4476.*(-t2503+t2754+t3433-t3460+t3506+t4.*t871.*(t534-t546).*9.52624335e-4)+t4753.*(t1176-t1366+t2434+t2435-t2899+t1430.*(t539+t641))+t6106.*(t1176-t1366+t2434+t2435-t2899+t1430.*(t539+t641));
et69 = t4447.*(t1692+t1786+t1910+t1964+t2305-t2600-t2797-t2860-t2936-t3147+t3167-t3232+t3720+t3721-t3903+t1430.*(t539+t641).*3.372816795e-3+t1181.*(t105-t465).*3.36554e-3+t11.*t381.*(t534-t546).*3.36554e-3);
et70 = t4897.*(-t1865+t1970+t2708+t3161-t3236-t3845-t3870+t1240.*(t105-t465).*3.36554e-3+t903.*(t534-t546).*3.36554e-3)+ITail.*t4310.*(t1064+t1137-t1694+t1698-t1763-t1774)+ITail.*t4350.*(t867+t1059-t1646-t1705+t1938-t2002)+ITail.*t4277.*(t1147+t1193-t1785+t1787-t1853-t1858)+ITail.*t4313.*(t949+t1142-t1730-t1792+t2049-t2139)+ITail.*t4459.*(t1176-t1366+t2434+t2435-t2899+t1430.*(t539+t641));
et71 = ITail.*t4447.*(t1255-t1465+t2578+t2579-t2997+(t1430.*(t539+t641))./2.0);
t6891 = -dphi1.*(et66+et67+et68+et69+et70+et71);
et72 = t1149-t1344+t1348+t1455+t1896-t1898-t2188+t2196+t2978+t3709-t4169+t4184+t4197+t4307-t4319+t4349+t4545-t4553+t4655-t4662+t5053+t5083-t5198-t5223+t5420-t5565-t5707-t5732+t5791-t5880-t5935-t5941-t5960-t6116+t6347+t6400+t6701-t6703+t6746-t6764+t4681.*(t1064+t1137-t1694+t1698-t1763-t1774)+t4704.*(t867+t1059-t1646-t1705+t1938-t2002)+t6105.*(t867+t1059-t1646-t1705+t1938-t2002)+t6104.*(t753+t991-t1771-t1957+t1181.*(t105-t465)+t11.*t381.*(t534-t546));
et73 = t4313.*(t1692+t1899+t1910+t2152+t2155-t2401-t2936-t2962-t3031-t3147+t3307-t3387+t3582+t3583-t3837+t1430.*(t539+t641).*3.36554e-3+t1181.*(t105-t465).*3.36554e-3+t11.*t381.*(t534-t546).*3.36554e-3);
et74 = t4476.*(-t2503+t2754+t3433-t3460+t3506+t4.*t871.*(t534-t546).*9.52624335e-4)+t4753.*(t1176-t1366+t2434+t2435-t2899+t1430.*(t539+t641))+t6106.*(t1176-t1366+t2434+t2435-t2899+t1430.*(t539+t641));
et75 = t4447.*(t1692+t1786+t1910+t1964+t2305-t2600-t2797-t2860-t2936-t3147+t3167-t3232+t3720+t3721-t3903+t1430.*(t539+t641).*3.372816795e-3+t1181.*(t105-t465).*3.36554e-3+t11.*t381.*(t534-t546).*3.36554e-3);
et76 = t4897.*(-t1865+t1970+t2708+t3161-t3236-t3845-t3870+t1240.*(t105-t465).*3.36554e-3+t903.*(t534-t546).*3.36554e-3)+ITail.*t4310.*(t1064+t1137-t1694+t1698-t1763-t1774)+ITail.*t4350.*(t867+t1059-t1646-t1705+t1938-t2002)+ITail.*t4277.*(t1147+t1193-t1785+t1787-t1853-t1858)+ITail.*t4313.*(t949+t1142-t1730-t1792+t2049-t2139)+ITail.*t4459.*(t1176-t1366+t2434+t2435-t2899+t1430.*(t539+t641));
et77 = ITail.*t4447.*(t1255-t1465+t2578+t2579-t2997+(t1430.*(t539+t641))./2.0);
t6892 = dphi1.*(et72+et73+et74+et75+et76+et77);
t4875 = dphi2.*t4868;
t4876 = dx.*t4868;
t4962 = -t4956;
t5261 = -t5255;
t5373 = dy.*t5365;
t5491 = -t5485;
t5512 = -t5506;
t5626 = t3548+t4533+t4543;
t5680 = -t5671;
t5784 = -t5777;
t5882 = -t5876;
t5884 = -t5877;
t5888 = -t5886;
t5893 = t4087+t4637+t4650;
t5903 = -t5900;
t5934 = -t5927;
t5966 = -t5961;
t6035 = -t6033;
t6047 = -t6044;
t6055 = -t6053;
t6078 = -t6077;
t6081 = -t6080;
t6146 = -t6145;
t6151 = -t6149;
t6159 = dth1.*t6156;
t6170 = dphi1.*t6169;
t6175 = dphi1.*(-t888+t1657+t1725-t1764+t3397+t3467-t5365);
t6178 = -t6177;
t6237 = -t6232;
t6291 = -t6288;
t6300 = -t6297;
t6477 = -t6475;
t6496 = -t6494;
t6521 = dy.*t6517;
t6522 = dth1.*t6518;
t6560 = -t6559;
t6575 = -t6574;
t6600 = -t6596;
t6649 = -t6648;
t6652 = -t6651;
t6660 = -t6655;
t6670 = -t6665;
t6782 = t3486+t4086+t4211+t4322+t4333+t4636+t4648+t4680+t4697;
t6783 = t3575+t4064+t4211+t4337+t4345+t4615+t4631+t4680+t4697;
t6784 = t3486+t4064+t4241+t4322+t4333+t4615+t4631+t4694+t4706;
t6786 = t4863+t4889+t5727+t5825;
t6787 = t4755+t4893+t5192+t6112;
t6793 = t3915+t4368+t4690+t4957+t6514+t6594;
t6795 = t4089+t4482+t4492+t4983+t6545+t6662;
et78 = -t1513-t1521+t2636+t2728+t2737-t3855-t3858+t4360+t4373+t4379+t4800+t4802+t5063+t5067-t5146-t5188+t5497+t5506-t5544-t5554+t5828-t5854+t5961+t6002+t6032-t6118+t6177+t6250+t6324-t6471+t3967.*(-t2389+t3634+t1512.*(t105-t465).*9.53094055e-4)+(t1332+t2368+t1512.*(t105-t465)).*(t1667-t2347+t2438+t2447+t3012+t3022+t3458+t3543+t3587+t3594+t3600+t3621)+t4549.*(t1332+t2368+t1512.*(t105-t465))+t5780.*(-t1331+t2317+t1510.*(t103-t544))+Mt.*t3780.*(t451-t831+T_cg_H.*(t214-t541));
et79 = ITail.*t4072.*(t1332+t2368+t1512.*(t105-t465))+ITail.*t3967.*(t1386+t2501+(t1512.*(t105-t465))./2.0)+Mb.*t15.*t1512.*(t214-t541);
t6803 = -dphi2.*(et78+et79);
et80 = -t1513-t1521+t2636+t2728+t2737-t3855-t3858+t4360+t4373+t4379+t4800+t4802+t5063+t5067-t5146-t5188+t5497+t5506-t5544-t5554+t5828-t5854+t5961+t6002+t6032-t6118+t6177+t6250+t6324-t6471+t3967.*(-t2389+t3634+t1512.*(t105-t465).*9.53094055e-4)+(t1332+t2368+t1512.*(t105-t465)).*(t1667-t2347+t2438+t2447+t3012+t3022+t3458+t3543+t3587+t3594+t3600+t3621)+t4549.*(t1332+t2368+t1512.*(t105-t465))+t5780.*(-t1331+t2317+t1510.*(t103-t544))+Mt.*t3780.*(t451-t831+T_cg_H.*(t214-t541));
et81 = ITail.*t4072.*(t1332+t2368+t1512.*(t105-t465))+ITail.*t3967.*(t1386+t2501+(t1512.*(t105-t465))./2.0)+Mb.*t15.*t1512.*(t214-t541);
t6804 = dphi2.*(et80+et81);
t6810 = t2733+t2734+t4205+t4206+t4370+t4375+t4614+t4619+t4963+t4984+t5177+t5185+t5229+t5233+t5240+t5342+t5356+t5387+t5553+t5595+t5606+t5685+t5730+t5969+t6050+t6065+t6119+t6164+t6201+t6238+t6274+t6276+t6549+t6580;
et82 = t2920+t2927+t3489-t3494+t3722-t3784+t964.*(t105-t465).*3.36554e-3+t977.*(t105-t465).*3.36554e-3+t1430.*(t103-t544).*3.36554e-3+t1512.*(t103-t544).*3.36554e-3;
et83 = t1510.*(t197-t537).*3.372816795e-3+t1505.*(t214-t541).*3.372816795e-3;
et84 = -t2733+t4186+t4187-t4375+t4604+t4608-t5229-t5240+t5333+t5377+t5586-t5606-t5730+t5964-t6050-t6164+t6197+t6236-t6274-t6580+t5442.*(t1751+t2308+t964.*(t105-t465)+t1430.*(t103-t544))+t4392.*(t2591-t3773+t1430.*(t197-t537).*1.90524867e-3)+t3938.*(et82+et83)+t4820.*(t2449.*3.372786875e-3+t3544+t3545+t3598-t3934-t3966);
et85 = t4555.*(t2436-t2536+t1510.*(t197-t537)+t1505.*(t214-t541))+t5434.*(t2436-t2536+t1510.*(t197-t537)+t1505.*(t214-t541))+t3938.*(t3716-t3777+t1510.*(t197-t537).*9.52624335e-4+t1505.*(t214-t541).*9.52624335e-4)+t4634.*(t1396-t2573+t1430.*(t197-t537).*2.0)+Mt.*t3774.*(t433-t828+T_cg_H.*(t197-t537))+ITail.*t4392.*(t1368-t2524+t1430.*(t197-t537));
et86 = ITail.*t4409.*(t1396-t2573+t1430.*(t197-t537).*2.0)+ITail.*t4077.*(t2436-t2536+t1510.*(t197-t537)+t1505.*(t214-t541))+ITail.*t3938.*(t2582-t2684+(t1510.*(t197-t537))./2.0+(t1505.*(t214-t541))./2.0)+Mb.*t15.*t1510.*(t197-t537);
t6811 = -dth2.*(et84+et85+et86);
t6815 = t2733+t2734+t4186+t4187+t4370+t4375+t4604+t4608+t4700+t4702+t4708+t4710+t4838+t4840+t4843+t4845+t4857+t4862+t4940+t4941+t5035+t5040+t5186+t5191+t5598+t5725+t5744+t5795+t5814+t5883+t6079+t6101+t6161+t6189+t6194+t6349+t6482+t6483+t6512;
et87 = t1246-t1302+t2197-t2268+t2348+t3256-t3330+t4243-t4263+t4278-t5224-t5254-t5602-t5890-t5999-t6215+t6266+t6293+t6297-t6404-t6669+t4408.*(t2587-t3868+t1505.*(t534-t546).*1.90524867e-3)+t4555.*(-t1129+t1139-t2082+t2110+t2123+t8.*t872.*(t534-t546))+t5434.*(-t1129+t1139-t2082+t2110+t2123+t8.*t872.*(t534-t546));
et88 = t4454.*(-t2389+t3634+t1512.*(t105-t465).*9.53094055e-4)+t3938.*(t2215-t2237+t3424+t3427-t3439+t8.*t872.*(t534-t546).*9.52624335e-4)+t5394.*(t1060+t1138-t1883+t1932+t2088+t1179.*(t103-t544));
et89 = t3938.*(t1645+t1965+t2072+t2220-t2242-t2409-t2483-t2504-t3093+t3155+t3261+t3432+t3437-t3442+t1179.*(t103-t544).*3.36554e-3+t3.*t575.*(t105-t465).*3.36554e-3+t8.*t872.*(t534-t546).*3.372816795e-3)+t4936.*(t1332+t2368+t1512.*(t105-t465))+t4737.*(t1395-t2868+t1505.*(t534-t546).*2.0);
et90 = Mt.*t2914.*(t433-t828+T_cg_H.*(t197-t537))+ITail.*t4408.*(t1365-t2831+t1505.*(t534-t546))+ITail.*t4452.*(t1395-t2868+t1505.*(t534-t546).*2.0)+ITail.*t4077.*(-t1129+t1139-t2082+t2110+t2123+t8.*t872.*(t534-t546))+ITail.*t3938.*(-t1189+t1195-t2210+t2241+t2248+(t8.*t872.*(t534-t546))./2.0)+ITail.*t4490.*(t1332+t2368+t1512.*(t105-t465))+ITail.*t4454.*(t1386+t2501+(t1512.*(t105-t465))./2.0)+Mb.*t15.*t1178.*(t197-t537);
t6820 = -dphi1.*(et87+et88+et89+et90);
t6821 = t1518+t1597+t2068+t2153+t2329+t2334+t3847+t3909+t4222+t4250+t4303+t4305+t5027+t5047+t5055+t5069+t5251+t5276+t5318+t5330+t5423+t5436+t5449+t5622+t5687+t5697+t5904+t5938+t6012+t6136+t6154+t6216+t6271+t6285+t6301+t6408+t6639+t6692;
t6823 = t3980+t4024+t4201+t4219+t4562+t4566+t4651+t4656+t4742+t4750+t4751+t4759+t4811+t4813+t4815+t4819+t4911+t4914+t4977+t4981+t4998+t5005+t5111+t5125+t5690+t5745+t5762+t5787+t5820+t5912+t6096+t6128+t6150+t6207+t6213+t6371+t6498+t6499+t6528;
t6826 = t1307+t1639+t2065+t2069+t2637+t2861+t3304+t3928+t4155+t4179+t4361+t4400+t4978+t5009+t5178+t5194+t5273+t5303+t5327+t5338+t5379+t5391+t5546+t5646+t5699+t5785+t5921+t5947+t6048+t6142+t6155+t6203+t6258+t6269+t6284+t6415+t6666+t6724;
et91 = t1242+t1596+t1977+t1979-t2637+t2798+t3248+t3908+t4141+t4160-t4361+t4394-t5178-t5194+t5264+t5295-t5327-t5338-t5546+t5637-t5699-t5785+t5916-t5947+t6139-t6155+t6199+t6265-t6284+t6412-t6666+t4408.*(t2591-t3773+t1430.*(t197-t537).*1.90524867e-3)+t6614.*(t1332+t2368+t1512.*(t105-t465))+t5442.*(t1019-t1651+t1702+t3.*t818.*(t105-t465)+t3.*t872.*(t103-t544))+t4737.*(t1396-t2573+t1430.*(t197-t537).*2.0)+t6099.*(-t1331+t2317+t1510.*(t103-t544));
et92 = ITail.*t4408.*(t1368-t2524+t1430.*(t197-t537))+ITail.*t4452.*(t1396-t2573+t1430.*(t197-t537).*2.0);
t6827 = -dth2.*(et91+et92);
t6828 = t4140+t4154+t4238+t4239+t4625+t4635+t4660+t4666+t4764+t4769+t4771+t4773+t4780+t4788+t4791+t4797+t4929+t4937+t4943+t4955+t5030+t5052+t5062+t5091+t5724+t5726+t5831+t5846+t5849+t5965+t6130+t6140+t6143+t6225+t6229+t6393+t6507+t6508+t6544;
et93 = t1309+t1929+t2282-t2348+t3325+t3957+t3985+t4010+t4257+t4268+t4502+t4503-t5274+t5280-t5294+t5308-t5644+t5648-t5917+t5926+t6077-t6147+t6219-t6304-t6311-t6658+t4476.*(t2591-t3773+t1430.*(t197-t537).*1.90524867e-3);
et94 = t4820.*(t1970-t1971+t2487+t3161-t3236-t3794-t3817+t1240.*(t105-t465).*3.372786875e-3+t903.*(t534-t546).*3.372786875e-3);
et95 = t4820.*(-t1974+t1240.*(t105-t465).*9.53094055e-4+t903.*(t534-t546).*9.53094055e-4)+t6611.*(t1332+t2368+t1512.*(t105-t465))+t5394.*(t820+t1121-t1435+t1997+t2000+t11.*t420.*(t214-t541))+t4787.*(t1396-t2573+t1430.*(t197-t537).*2.0)+t5548.*(-t947+t1240.*(t105-t465)+t903.*(t534-t546))+t6129.*(-t947+t1240.*(t105-t465)+t903.*(t534-t546));
et96 = ITail.*t4476.*(t1368-t2524+t1430.*(t197-t537))+ITail.*t4522.*(t1396-t2573+t1430.*(t197-t537).*2.0)+ITail.*t4867.*(-t947+t1240.*(t105-t465)+t903.*(t534-t546))+ITail.*t4820.*(-t1017+(t1240.*(t105-t465))./2.0+(t903.*(t534-t546))./2.0);
t6831 = -dth2.*(et93+et94+et95+et96);
et97 = t1597+t2329+t2334-t2790+t3672+t3909-t4218+t4303+t4305+t4428+t5288+t5289+t5306+t5324+t5667+t5670+t5919+t5936+t6080-t6093+t6149-t6234-t6296-t6426-t6740+t4447.*(t2591-t3773+t1430.*(t197-t537).*1.90524867e-3)+t5548.*(-t1262+t1701+t9.*t868.*(t105-t465))+t6129.*(-t1262+t1701+t9.*t868.*(t105-t465))+t4820.*(-t2388+t3008+t9.*t868.*(t105-t465).*9.53094055e-4);
et98 = t3938.*(t1832.*3.36554e-3+t1866.*3.372816795e-3-t1962+t1983+t2287-t2322-t2472+t2479+t2512+t2571+t2722+t2803+t3122+t3326+t3344-t3357+t3423+t496.*(t214-t541).*3.36554e-3)+t4753.*(t1396-t2573+t1430.*(t197-t537).*2.0)+t6106.*(t1396-t2573+t1430.*(t197-t537).*2.0)+Mt.*t3937.*(t451-t831+T_cg_H.*(t214-t541));
et99 = ITail.*t4447.*(t1368-t2524+t1430.*(t197-t537))+ITail.*t4459.*(t1396-t2573+t1430.*(t197-t537).*2.0)+ITail.*t4867.*(-t1262+t1701+t9.*t868.*(t105-t465))+ITail.*t4820.*(-t1355+t1789+(t9.*t868.*(t105-t465))./2.0)+B_cg_H.*Mb.*t2563.*(t214-t541);
t6833 = -dth2.*(et97+et98+et99);
et100 = t1597+t2329+t2334-t2790+t3672+t3909-t4218+t4303+t4305+t4428+t5288+t5289+t5306+t5324+t5667+t5670+t5919+t5936+t6080-t6093+t6149-t6234-t6296-t6426-t6740+t4447.*(t2591-t3773+t1430.*(t197-t537).*1.90524867e-3)+t5548.*(-t1262+t1701+t9.*t868.*(t105-t465))+t6129.*(-t1262+t1701+t9.*t868.*(t105-t465))+t4820.*(-t2388+t3008+t9.*t868.*(t105-t465).*9.53094055e-4);
et101 = t3938.*(t1832.*3.36554e-3+t1866.*3.372816795e-3-t1962+t1983+t2287-t2322-t2472+t2479+t2512+t2571+t2722+t2803+t3122+t3326+t3344-t3357+t3423+t496.*(t214-t541).*3.36554e-3)+t4753.*(t1396-t2573+t1430.*(t197-t537).*2.0)+t6106.*(t1396-t2573+t1430.*(t197-t537).*2.0)+Mt.*t3937.*(t451-t831+T_cg_H.*(t214-t541));
et102 = ITail.*t4447.*(t1368-t2524+t1430.*(t197-t537))+ITail.*t4459.*(t1396-t2573+t1430.*(t197-t537).*2.0)+ITail.*t4867.*(-t1262+t1701+t9.*t868.*(t105-t465))+ITail.*t4820.*(-t1355+t1789+(t9.*t868.*(t105-t465))./2.0)+B_cg_H.*Mb.*t2563.*(t214-t541);
t6834 = dth2.*(et100+et101+et102);
t6837 = t2289+t2352+t3481+t3487+t3974+t4037+t4121+t4153+t4455+t4456+t4525+t4537+t5104+t5142+t5268+t5292+t5381+t5410+t5421+t5435+t5508+t5513+t5633+t5737+t5771+t5913+t5977+t5985+t6070+t6076+t6167+t6233+t6257+t6316+t6321+t6437+t6681+t6738;
t6838 = -dth1.*(t2206+t2293+t3526+t3530+t4005+t4009+t4143+t4171+t4449+t4451+t4529+t4532+t5099+t5136+t5370+t5402-t5421-t5435+t5502+t5509+t5733-t5771+t5975-t5985-t6076-t6167-t6233+t6255+t6314+t6319+t6434-t6681+t5394.*(t995+t1064-t1506+t1598-t1763-t1774)+t4672.*(-t2389+t3634+t1512.*(t105-t465).*9.53094055e-4)+t5304.*(t1332+t2368+t1512.*(t105-t465))+t6620.*(t1332+t2368+t1512.*(t105-t465))+ITail.*t4712.*(t1332+t2368+t1512.*(t105-t465))+ITail.*t4672.*(t1386+t2501+(t1512.*(t105-t465))./2.0));
t6839 = t3094+t3110+t3739+t3749+t4012+t4026+t4332+t4334+t4457+t4458+t4567+t4571+t5050+t5094+t5316+t5335+t5344+t5361+t5425+t5439+t5461+t5465+t5688+t5709+t5772+t5949+t5958+t5984+t6084+t6115+t6168+t6243+t6248+t6302+t6307+t6418+t6733+t6765;
t6847 = t1302+t1929+t2268+t2269+t3330+t3957+t3985+t4010+t4262+t4263+t4502+t4503+t4723+t4724+t4732+t4733+t4904+t4905+t4906+t4907+t4966+t4967+t4975+t4976+t5241+t5242+t5244+t5245+t5797+t5822+t5845+t5864+t5993+t6013+t6113+t6134+t6195+t6208+t6212+t6278+t6469+t6481+t6495+t6497+t6500+t6532+t6536+t6548;
t6852 = t4183+t4220+t4607+t4630+t4993+t4997+t5010+t5031+t5238+t5249+t5263+t5345+t5363+t5384+t5443+t5456+t5494+t5545+t5592+t5616+t5629+t5672+t5750+t5768+t5776+t5867+t5983+t6029+t6183+t6283+t6303+t6342+t6343+t6396+t6552+t6581+t6584+t6687+t6698+t6728;
t6856 = t3952+t4006+t4085+t4091+t4477+t4511+t4526+t4541+t4901+t4912+t4982+t4985+t5090+t5218+t5234+t5311+t5346+t5353+t5483+t5492+t5535+t5570+t5575+t5578+t5587+t5618+t5739+t5759+t5863+t5942+t5973+t6024+t6166+t6272+t6294+t6335+t6339+t6425+t6563+t6603+t6606+t6638+t6641+t6673;
t6859 = t3975+t3981+t4085+t4091+t4495+t4501+t4526+t4541+t5101+t5109+t5114+t5130+t5139+t5141+t5143+t5180+t5352+t5406+t5488+t5499+t5511+t5522+t5523+t5543+t5620+t5676+t5735+t5835+t5837+t5879+t5905+t6014+t6196+t6205+t6281+t6370+t6372+t6413+t6565+t6567+t6602+t6678+t6680+t6721;
t6861 = t3671+t3678+t4107+t4129+t4421+t4425+t4559+t4560+t5078+t5088+t5121+t5156+t5162+t5169+t5226+t5267+t5364+t5453+t5468+t5480+t5487+t5517+t5555+t5561+t5588+t5700+t5747+t5801+t5843+t5881+t5929+t6018+t6204+t6241+t6290+t6350+t6353+t6403+t6562+t6571+t6588+t6714+t6715+t6741;
t6863 = t2569+t2667+t2819+t2839+t3030+t4003+t4033+t4427+t4443+t4758+t4765+t5004+t5012+t5116+t5127+t5144+t5193+t5277+t5315+t5380+t5398+t5495+t5505+t5507+t5516+t5531+t5653+t5654+t5692+t5827+t5838+t5862+t5892+t5954+t6058+t6211+t6253+t6330+t6333+t6338+t6407+t6553+t6564+t6576+t6752+t6753+t6766;
et103 = t2465+t2567-t2819-t3030+t3998-t4003-t4427+t4429-t4758+t4761+t5106+t5117+t5137+t5184+t5266+t5307+t5393-t5495+t5500-t5505+t5521+t5643-t5653-t5692-t5827-t5838+t5857-t5892+t5951-t6058-t6211-t6333+t6336-t6407-t6564-t6576+t6750+t6751-t6766+t4770.*(t2449.*3.36554e-3+t3490+t3648+t3649-t3934-t3966)+t4923.*(t2449.*3.36554e-3+t3490+t3544+t3545-t4001-t4034);
et104 = t4949.*(-t1262+t1701+t9.*t868.*(t105-t465))+t6458.*(-t1262+t1701+t9.*t868.*(t105-t465))+t4575.*(-t2388+t3008+t9.*t868.*(t105-t465).*9.53094055e-4)+ITail.*t4617.*(-t1262+t1701+t9.*t868.*(t105-t465))+ITail.*t4575.*(-t1355+t1789+(t9.*t868.*(t105-t465))./2.0)+t2.*t10.*(t1223-t1252);
t6864 = -dth1.*(et103+et104);
et105 = t2465+t2567-t2819-t3030+t3998-t4003-t4427+t4429-t4758+t4761+t5106+t5117+t5137+t5184+t5266+t5307+t5393-t5495+t5500-t5505+t5521+t5643-t5653-t5692-t5827-t5838+t5857-t5892+t5951-t6058-t6211-t6333+t6336-t6407-t6564-t6576+t6750+t6751-t6766+t4770.*(t2449.*3.36554e-3+t3490+t3648+t3649-t3934-t3966)+t4923.*(t2449.*3.36554e-3+t3490+t3544+t3545-t4001-t4034);
et106 = t4949.*(-t1262+t1701+t9.*t868.*(t105-t465))+t6458.*(-t1262+t1701+t9.*t868.*(t105-t465))+t4575.*(-t2388+t3008+t9.*t868.*(t105-t465).*9.53094055e-4)+ITail.*t4617.*(-t1262+t1701+t9.*t868.*(t105-t465))+ITail.*t4575.*(-t1355+t1789+(t9.*t868.*(t105-t465))./2.0)+t2.*t10.*(t1223-t1252);
t6865 = dth1.*(et105+et106);
t6869 = t1391+t1393+t2834+t2836+t4463+t4473+t4804+t4806+t5102+t5105+t5107+t5122+t5173+t5204+t5214+t5239+t5419+t5463+t5475+t5503+t5613+t5631+t5649+t5651+t5766+t5792+t5874+t5894+t5909+t5914+t5974+t6100+t6224+t6235+t6361+t6365+t6373+t6447+t6577+t6579+t6610+t6762+t6763+t6775;
t6871 = t1939+t2471+t2877+t2917+t3321+t3333+t3959+t4068+t4269+t4280+t4312+t4324+t4909+t4913+t4950+t4969+t5227+t5310+t5354+t5382+t5416+t5441+t5498+t5594+t5619+t5634+t5673+t5713+t5738+t5775+t5872+t5898+t5982+t5998+t6036+t6052+t6286+t6327+t6382+t6416+t6436+t6445+t6640+t6653+t6671+t6677+t6731+t6734;
t6873 = t2192+t2276+t2338+t2345+t2842+t2844+t2879+t2912+t2913+t2977+t3109+t4008+t4038+t4316+t4320+t4327+t4331+t4659+t4663+t4673+t4674+t5001+t5039+t5064+t5075+t5138+t5145+t5190+t5220+t5253+t5447+t5458+t5532+t5574+t5593+t5604+t5614+t5645+t5683+t5763+t5819+t5871+t5902+t5953+t6042+t6182+t6222+t6315+t6344+t6348+t6435+t6572+t6583+t6609+t6695+t6696+t6727;
t6875 = t1050+t1624+t1665+t2023+t2516+t3841+t3889+t3951+t3976+t3995+t4470+t4506+t5033+t5059+t5061+t5066+t5309+t5339+t5411+t5412+t5438+t5444+t5528+t5573+t5661+t5694+t5704+t5706+t5774+t5779+t5841+t5908+t5968+t6000+t6021+t6057+t6354+t6358+t6366+t6417+t6444+t6450+t6663+t6700+t6707+t6723+t6725+t6747;
t6876 = dth2.*(t1050+t1624+t2023+t2516+t3841+t3889+t3951+t3976+t3995+t4470+t4506+t5033+t5059+t5061+t5066+t5309+t5339+t5411+t5412+t5438+t5444+t5528+t5573+t5661+t5694+t5704+t5706+t5774+t5779+t5841+t5908+t5968+t6000+t6021+t6057+t6354+t6358+t6366+t6417+t6444+t6450+t6663+t6700+t6707+t6723+t6725+t6747-Mb.*t11.*t15.*t542.*(t197-t537));
t6879 = t1304+t1747+t1809+t2963+t3331+t3609+t3792+t3996+t4041+t4253+t4406+t4453+t5021+t5032+t5051+t5076+t5396+t5399+t5426+t5427+t5462+t5484+t5549+t5589+t5615+t5638+t5674+t5756+t5788+t5813+t5852+t5885+t5995+t6010+t6028+t6039+t6337+t6360+t6390+t6420+t6432+t6441+t6689+t6694+t6716+t6737+t6744+t6748;
t6881 = t2117+t2471+t3321+t3333+t3851+t3856+t3964+t4068+t4312+t4324+t4431+t4438+t5126+t5150+t5179+t5205+t5243+t5269+t5284+t5322+t5493+t5547+t5568+t5611+t5623+t5636+t5658+t5681+t5840+t5861+t5869+t5889+t5931+t5956+t6031+t6045+t6367+t6379+t6385+t6406+t6431+t6446+t6683+t6708+t6719+t6722+t6735+t6761;
t6884 = t2818+t2889+t3403+t3415+t3750+t3793+t4216+t4236+t4354+t4356+t4432+t4450+t4931+t4932+t5072+t5098+t5275+t5448+t5450+t5455+t5470+t5478+t5539+t5600+t5624+t5695+t5714+t5802+t5805+t5809+t5875+t5930+t6004+t6008+t6037+t6069+t6305+t6368+t6398+t6427+t6438+t6451+t6650+t6674+t6705+t6736+t6768+t6771;
t6886 = t1703+t2108+t3504+t3787+t3834+t3933+t3953+t3977+t4371+t4401+t4486+t4507+t4925+t4933+t5103+t5131+t5265+t5383+t5385+t5413+t5414+t5476+t5530+t5632+t5668+t5753+t5754+t5789+t5815+t5832+t5895+t5990+t5991+t5992+t6051+t6109+t6309+t6380+t6383+t6433+t6448+t6463+t6645+t6647+t6699+t6756+t6778+t6780;
t6888 = t1453+t1460+t1664+t1693+t2285+t2341+t3647+t3724+t4047+t4059+t4330+t4340+t4348+t4355+t4496+t4497+t4665+t4678+t5112+t5140+t5206+t5221+t5232+t5250+t5332+t5359+t5486+t5582+t5621+t5711+t5720+t5731+t5746+t5767+t5834+t5887+t5915+t5945+t5972+t5976+t6075+t6086+t6364+t6375+t6394+t6421+t6454+t6460+t6713+t6729+t6755+t6758+t6759+t6777;
t6889 = dth1.*(-t1378-t1384+t1664+t1693+t2285+t2341+t3647+t3724+t4047+t4059+t4330+t4340+t4348+t4355+t4496+t4497+t4665+t4678+t5112+t5140+t5206+t5221+t5232+t5250+t5332+t5359+t5486+t5582+t5621+t5711+t5720+t5731+t5746+t5767+t5834+t5887+t5915+t5945+t5972+t5976+t6075+t6086+t6364+t6375+t6394+t6421+t6454+t6460+t6713+t6729+t6755+t6758+t6759+t6777);
t6890 = t1186+t1344+t1373+t1526+t1898+t1942+t2188+t2281+t3050+t3769+t4169+t4200+t4210+t4317+t4319+t4358+t4552+t4553+t4661+t4662+t5058+t5092+t5198+t5223+t5247+t5272+t5305+t5329+t5431+t5565+t5640+t5701+t5707+t5732+t5800+t5807+t5826+t5880+t5935+t5941+t5960+t5994+t6074+t6116+t6351+t6386+t6392+t6401+t6455+t6470+t6702+t6703+t6749+t6764+t6770+t6781;
t6172 = -t6170;
t6524 = -t6522;
t6789 = t4880+t5341+t6162+t6175;
t6790 = t3882+t3883+t4547+t4875+t5728+t6477;
t6791 = t4182+t4190+t4434+t4894+t6011+t6496;
t6796 = t4097+t4475+t4574+t4973+t6542+t6660;
t6799 = t4291+t4302+t4727+t4729+t4832+t4841+t4846+t4853+t5016+t5018+t5123+t5148+t5155+t5161+t5403+t5520+t5552+t5798+t5884+t5899+t6046+t6061+t6114+t6158+t6181;
t6802 = t1513+t1521+t2735+t2746+t2794+t2805+t3855+t3858+t4365+t4372+t4384+t4391+t4803+t4805+t4807+t4809+t5074+t5077+t5080+t5082+t5146+t5188+t5504+t5512+t5544+t5554+t5830+t5854+t5966+t6007+t6034+t6092+t6118+t6178+t6251+t6326+t6471+t6506;
t6805 = t1777+t2796+t2811+t3180+t3950+t4019+t4099+t4339+t4412+t4414+t4558+t4570+t4847+t4848+t4864+t4865+t5152+t5153+t5165+t5166+t5174+t5212+t5560+t5579+t5584+t5591+t5858+t5903+t5934+t6025+t6062+t6073+t6127+t6180+t6259+t6334+t6490+t6520;
t6807 = t1593+t2316+t2972+t3040+t3902+t4116+t4133+t4165+t4440+t4448+t4610+t4613+t4888+t4890+t4892+t4895+t5197+t5199+t5202+t5203+t5225+t5262+t5625+t5630+t5663+t5680+t5896+t5910+t5918+t6055+t6068+t6071+t6144+t6186+t6277+t6346+t6503+t6533;
t6812 = t3993+t4007+t4201+t4219+t4561+t4568+t4651+t4656+t5002+t5028+t5154+t5171+t5209+t5211+t5281+t5326+t5360+t5409+t5527+t5571+t5590+t5677+t5708+t5957+t6035+t6040+t6132+t6171+t6214+t6246+t6273+t6289+t6535+t6568;
t6816 = dphi2.*t6815;
t6817 = t4119+t4139+t4238+t4239+t4616+t4624+t4660+t4666+t5014+t5049+t5217+t5228+t5290+t5297+t5298+t5301+t5337+t5422+t5536+t5599+t5682+t5719+t5770+t5946+t6041+t6063+t6152+t6176+t6209+t6244+t6264+t6291+t6561+t6598;
t6819 = t1302+t1309+t2268+t2269+t2282+t2286+t3325+t3330+t4257+t4262+t4263+t4268+t5008+t5017+t5038+t5085+t5224+t5254+t5302+t5319+t5378+t5452+t5459+t5602+t5657+t5684+t5890+t5932+t5999+t6126+t6153+t6215+t6270+t6299+t6300+t6404+t6634+t6669;
t6822 = dth1.*t6821;
t6824 = dphi2.*t6823;
t6829 = dphi2.*t6828;
t6830 = t1246+t1993+t2197+t2348+t3256+t3926+t3956+t3986+t4243+t4278+t4488+t4489+t5048+t5093+t5274+t5285+t5294+t5321+t5395+t5418+t5460+t5464+t5644+t5659+t5742+t5917+t5933+t5981+t6072+t6078+t6147+t6223+t6249+t6304+t6311+t6440+t6658+t6720;
t6832 = t1640+t2391+t2406+t2790+t3680+t3744+t3929+t4218+t4314+t4315+t4420+t4442+t5000+t5034+t5296+t5299+t5314+t5328+t5350+t5389+t5407+t5415+t5675+t5678+t5723+t5928+t5939+t5970+t6081+t6093+t6151+t6234+t6240+t6280+t6296+t6426+t6682+t6740;
t6835 = t2293+t2887+t3526+t3530+t3832+t3859+t4171+t4234+t4449+t4451+t4467+t4472+t5084+t5118+t5172+t5207+t5312+t5343+t5368+t5388+t5481+t5489+t5542+t5691+t5734+t5870+t5948+t5971+t6047+t6085+t6163+t6242+t6247+t6306+t6310+t6411+t6667+t6730;
t6840 = dth1.*t6839;
t6841 = t2113+t2458+t3962+t4048+t4065+t4117+t4120+t4156+t4538+t4546+t4620+t4621+t5128+t5163+t5347+t5349+t5374+t5376+t5524+t5533+t5557+t5569+t5715+t5717+t5855+t5962+t5963+t6023+t6087+t6097+t6179+t6237+t6254+t6318+t6322+t6430+t6754+t6772;
t6844 = t1444+t2061+t2161+t2790+t3680+t3744+t3823+t4218+t4228+t4232+t4420+t4442+t4707+t4709+t4711+t4713+t4917+t4918+t4926+t4927+t4938+t4942+t4944+t4946+t5278+t5279+t5286+t5287+t5764+t5783+t5784+t5810+t5979+t5987+t6094+t6108+t6184+t6190+t6228+t6262+t6462+t6465+t6478+t6484+t6501+t6523+t6526+t6530;
t6848 = dphi2.*t6847;
t6849 = t2206+t2887+t3832+t3859+t4005+t4009+t4143+t4234+t4467+t4472+t4529+t4532+t4772+t4776+t4784+t4789+t4826+t4827+t4835+t4836+t5036+t5042+t5046+t5054+t5157+t5158+t5167+t5168+t5836+t5851+t5865+t5882+t6006+t6022+t6131+t6146+t6218+t6220+t6230+t6261+t6479+t6491+t6504+t6505+t6509+t6525+t6546+t6551;
t6854 = t3671+t3678+t4108+t4127+t4421+t4425+t4557+t4565+t4924+t4934+t4939+t4947+t5135+t5182+t5196+t5291+t5336+t5369+t5430+t5479+t5491+t5534+t5538+t5581+t5585+t5601+t5718+t5755+t5812+t5888+t5980+t6027+t6174+t6279+t6295+t6323+t6331+t6402+t6537+t6573+t6575+t6649+t6652+t6697;
t6857 = dphi1.*t6856;
t6860 = dth2.*t6859;
t6862 = dth2.*t6861;
t6866 = t1196+t1397+t1433+t2106+t2189+t2338+t2345+t4316+t4321+t4327+t4329+t4659+t4663+t4664+t4679+t5041+t5057+t5068+t5087+t5095+t5120+t5132+t5149+t5340+t5386+t5417+t5467+t5541+t5551+t5559+t5617+t5666+t5698+t5833+t5844+t5850+t5868+t5922+t6060+t6191+t6202+t6332+t6345+t6356+t6423+t6558+t6560+t6582+t6709+t6710+t6742;
t6874 = dphi1.*t6873;
t6877 = t1939+t2117+t2877+t2917+t3851+t3856+t3959+t3964+t4269+t4280+t4431+t4438+t4953+t4954+t5025+t5056+t5293+t5317+t5325+t5400+t5408+t5428+t5576+t5642+t5679+t5689+t5696+t5712+t5765+t5773+t5901+t5925+t5959+t5996+t6054+t6066+t6317+t6357+t6362+t6442+t6449+t6453+t6657+t6670+t6688+t6717+t6743+t6745;
t6880 = dth2.*t6879;
t6885 = dth1.*t6884;
t6788 = t4852+t5362+t6159+t6172;
t6794 = t3880+t4367+t4682+t4962+t6524+t6595;
t6800 = dphi2.*t6799;
t6806 = dphi2.*t6805;
t6808 = dphi2.*t6807;
t6813 = dth1.*t6812;
t6818 = dphi1.*t6817;
t6825 = -t6824;
t6836 = dphi1.*t6835;
t6842 = dphi1.*t6841;
t6845 = dphi2.*t6844;
t6850 = dphi2.*t6849;
t6855 = dth1.*t6854;
t6858 = -t6857;
t6867 = dth1.*t6866;
t6878 = dth1.*t6877;
t6894 = t6804+t6820+t6822+t6827;
t6801 = -t6800;
t6809 = -t6808;
t6814 = -t6813;
t6843 = -t6842;
t6846 = -t6845;
t6851 = -t6850;
t6868 = -t6867;
t6895 = t5195+t5257+t5261+t6806+t6834+t6836+t6840;
t6897 = t4554+t4684+t4685+t6816+t6853+t6855+t6858;
C = ft_14({B_cg_H,ITail,Mb,Mm,Mt,T_cg_H,dphi1,dphi2,dpsi1,dth1,dth2,dx,dy,dz,t10,t1005,t1007,t1008,t1009,t1013,t1016,t1017,t1018,t1019,t1023,t1029,t103,t1037,t1047,t105,t1053,t1059,t1060,t1064,t1079,t1084,t1086,t1088,t1097,t1099,t11,t1102,t1108,t1113,t1121,t1129,t1137,t1138,t1139,t1141,t1142,t1143,t1147,t1149,t1153,t1157,t1159,t1167,t1169,t1170,t1173,t1176,t1178,t1179,t1181,t1185,t1189,t1193,t1194,t1195,t120,t1203,t1205,t1206,t1215,t1221,t1223,t1224,t1225,t1228,t1229,t1230,t1234,t1240,t1242,t1245,t1247,t1250,t1252,t1253,t1255,t1260,t1261,t1262,t1264,t1265,t1268,t1283,t1291,t130,t1301,t1304,t1305,t1309,t1322,t1328,t1331,t1332,t1334,t1337,t1338,t134,t1343,t1345,t1352,t1354,t1355,t1360,t1362,t1365,t1366,t1368,t1370,t1371,t1374,t1381,t1382,t1384,t1386,t1388,t1389,t1394,t1395,t1396,t1412,t1413,t1421,t1426,t1427,t1430,t1431,t1435,t144,t1441,t1443,t1446,t1456,t1465,t1466,t1470,t1487,t1495,t15,t1505,t1506,t1510,t1512,t1521,t1528,t1531,t1535,t1540,t1544,t1552,t1558,t1568,t1575,t1578,t1581,t1586,t1593,t1598,t1609,t161,t1618,t1619,t1620,t1624,t1635,t1645,t1646,t1651,t1652,t1654,t1660,t1661,t1664,t1667,t1672,t1676,t1681,t1685,t1692,t1693,t1694,t1698,t1701,t1702,t1703,t1705,t1706,t1718,t1727,t1730,t1734,t1735,t1742,t1746,t1751,t1759,t1761,t1763,t1771,t1774,t1784,t1785,t1786,t1787,t1789,t1790,t1792,t1799,t1802,t1806,t1810,t1813,t1832,t1846,t1851,t1853,t1855,t1858,t1865,t1866,t1867,t1882,t1883,t1898,t1899,t1907,t1910,t1915,t1917,t1918,t1928,t1929,t1932,t1938,t1939,t1942,t195,t1956,t1957,t1959,t1962,t1964,t1965,t197,t1970,t1971,t1974,t1976,t1977,t1979,t1981,t1983,t1997,t2,t2000,t2002,t2007,t2008,t2015,t2020,t2032,t2037,t2038,t2047,t2049,t2057,t2058,t2059,t2062,t2064,t2067,t2072,t2075,t2076,t2082,t2083,t2086,t2087,t2088,t2096,t2104,t2110,t2111,t2123,t2131,t2134,t2135,t2137,t2139,t214,t2141,t2147,t2148,t2150,t2152,t2155,t2156,t2158,t2174,t2175,t2190,t2191,t2202,t2203,t2206,t2208,t2210,t2212,t2215,t2218,t2220,t2222,t2225,t2227,t2237,t2240,t2241,t2242,t2243,t2247,t2248,t2254,t2259,t2271,t2274,t2282,t2287,t2293,t2305,t2308,t2312,t2317,t2319,t2322,t2325,t2339,t2342,t2347,t2348,t2360,t2361,t2364,t2368,t2387,t2388,t2389,t2390,t24,t2401,t2404,t2409,t2412,t2413,t2419,t2420,t2430,t2434,t2435,t2436,t2438,t2447,t2449,t2463,t2468,t2472,t2479,t2483,t2487,t2489,t2495,t2496,t25,t2501,t2503,t2504,t2512,t2514,t2518,t2524,t2527,t2528,t2536,t2547,t2563,t2564,t2568,t2571,t2573,t2574,t2576,t2578,t2579,t2582,t2587,t259,t2590,t2591,t2597,t26,t260,t2600,t2605,t2613,t2616,t2617,t2621,t2627,t2632,t2638,t2657,t2660,t2663,t2665,t2669,t2679,t2684,t2688,t2692,t2696,t2699,t27,t2700,t2706,t2708,t2712,t2715,t2717,t2718,t2722,t2723,t2730,t2737,t2738,t2743,t2754,t2759,t276,t2763,t277,t2785,t2787,t2791,t2796,t2797,t2799,t2803,t2811,t2816,t2821,t2823,t2824,t2825,t2829,t283,t2831,t2833,t284,t2843,t2845,t2847,t2849,t285,t286,t2860,t2868,t287,t2871,t2875,t2876,t2877,t2878,t288,t2883,t2889,t289,t2899,t290,t291,t2914,t2915,t2918,t292,t2920,t2921,t2927,t293,t2930,t2936,t2937,t294,t2942,t2944,t2945,t2950,t2952,t2956,t2962,t2965,t2970,t2972,t2978,t2981,t2994,t2997,t3,t3008,t3009,t3012,t3022,t3031,t3034,t304,t3054,t3062,t3064,t3070,t3076,t3080,t3082,t3084,t3086,t3087,t3093,t3096,t3105,t3113,t3121,t3122,t3131,t3138,t3139,t3147,t3155,t3160,t3161,t3167,t3169,t3178,t3186,t3192,t3199,t3206,t3207,t3232,t3235,t3236,t3244,t3247,t3248,t3252,t3261,t3263,t3265,t3266,t3270,t3276,t3278,t3286,t3287,t3289,t3299,t3302,t3307,t3311,t3312,t3315,t3325,t3326,t3329,t3331,t3341,t3344,t3347,t3357,t3378,t3387,t3390,t3391,t3392,t3403,t3407,t3412,t3413,t3414,t3415,t3419,t3423,t3424,t3427,t3431,t3432,t3433,t3437,t3438,t3439,t3442,t3445,t3448,t3449,t3458,t3460,t3471,t3475,t3482,t3483,t3485,t3489,t3490,t3494,t3499,t3501,t3506,t3510,t3512,t3516,t3521,t3522,t3523,t3524,t3526,t3528,t3529,t3530,t3531,t3534,t3541,t3543,t3544,t3545,t3548,t3550,t3552,t3553,t3556,t3557,t3563,t3576,t3578,t3582,t3583,t3584,t3587,t3594,t3597,t3598,t3600,t3602,t3614,t3617,t3621,t3627,t3632,t3634,t3638,t3644,t3648,t3649,t3652,t3657,t3659,t3661,t3667,t3679,t3682,t3684,t3697,t3698,t3701,t3704,t3716,t3719,t3720,t3721,t3722,t3735,t3738,t3739,t3745,t3746,t3749,t3756,t376,t3764,t377,t3770,t3771,t3772,t3773,t3774,t3777,t3780,t3784,t3787,t3791,t3794,t381,t3811,t3814,t3815,t3817,t382,t383,t3834,t3836,t3837,t3841,t3845,t3848,t3858,t3862,t3868,t3870,t3879,t390,t3902,t3903,t3906,t3907,t3916,t3923,t3930,t3931,t3932,t3934,t3936,t3937,t3938,t394,t3940,t3944,t3947,t3948,t3955,t3957,t3961,t3962,t3965,t3966,t3967,t3969,t3971,t3982,t3983,t3985,t4,t4001,t4005,t4009,t4010,t4014,t4023,t4025,t4027,t4028,t4034,t4036,t4042,t4047,t4048,t4051,t4052,t4054,t4056,t4058,t4059,t4061,t4065,t4070,t4071,t4072,t4073,t4074,t4077,t4078,t4081,t4083,t4084,t4087,t4090,t4096,t4098,t4100,t4105,t411,t4111,t4112,t4115,t412,t4132,t4135,t4137,t4138,t414,t4141,t4143,t4144,t4145,t415,t4152,t4160,t4162,t4164,t4169,t4171,t4173,t4184,t4189,t4196,t4197,t420,t4208,t421,t4212,t4213,t4214,t4215,t4217,t4223,t4224,t4225,t4227,t4231,t4233,t4236,t4237,t4245,t4247,t425,t4255,t4256,t4257,t4258,t4268,t4271,t4272,t4273,t4274,t4276,t4277,t4281,t4282,t4286,t4296,t430,t4300,t4301,t4309,t431,t4310,t4311,t4313,t4318,t4323,t4324,t4326,t433,t4341,t4342,t4343,t4344,t4346,t4350,t4352,t4354,t4355,t4356,t4357,t436,t4371,t4374,t4379,t4382,t4392,t4393,t4395,t4399,t44,t4401,t4403,t4404,t4407,t4408,t4409,t4412,t4414,t4415,t4416,t4418,t4422,t4435,t4437,t4439,t4440,t4444,t4447,t4449,t445,t4451,t4452,t4454,t4457,t4458,t4459,t4461,t4462,t4469,t4471,t4476,t4479,t4480,t4481,t4483,t4484,t4485,t4487,t4490,t4493,t4498,t4500,t4502,t4503,t4505,t451,t4510,t4512,t4514,t4515,t4517,t4518,t4519,t4521,t4522,t4528,t4529,t4531,t4532,t4536,t4538,t4540,t4542,t4545,t4546,t4549,t4550,t4551,t4553,t4555,t4556,t4573,t4575,t4576,t4577,t4578,t4581,t4583,t4584,t4585,t4586,t4588,t459,t4590,t4591,t4592,t4596,t4597,t4598,t4602,t4603,t4605,t4606,t4609,t4617,t4618,t4623,t4626,t4629,t4634,t4638,t4639,t4640,t4644,t4645,t4646,t4647,t4649,t465,t4652,t4657,t4658,t4667,t4668,t4669,t4672,t4675,t4681,t4686,t4689,t4691,t4695,t4696,t4698,t4701,t4704,t4712,t4722,t4735,t4736,t4737,t4738,t4752,t4753,t4756,t4770,t4775,t4783,t4785,t4786,t4787,t4790,t4793,t4796,t48,t4814,t4816,t4820,t4821,t4823,t4830,t4834,t4849,t485,t4850,t4851,t4858,t4861,t4867,t4870,t4874,t4876,t4877,t488,t4881,t4882,t4883,t4897,t49,t4900,t4908,t4922,t4923,t4928,t4936,t4945,t4949,t4958,t4959,t496,t4960,t4961,t4964,t4972,t4980,t4989,t4995,t5,t50,t5006,t5013,t502,t5022,t5023,t5070,t5071,t5089,t5099,t51,t5136,t5175,t519,t5208,t5216,t523,t524,t527,t5274,t5280,t5294,t530,t5300,t5304,t5308,t5313,t534,t5351,t5354,t537,t5370,t5371,t5372,t5373,t5375,t5382,t539,t5392,t5394,t54,t5402,t5404,t5405,t541,t542,t5421,t5434,t5435,t544,t5442,t546,t5474,t55,t550,t5502,t5509,t5514,t5519,t553,t5548,t5556,t5566,t557,t558,t5597,t56,t5607,t5627,t5644,t5648,t5660,t5665,t5705,t5727,t5729,t573,t5733,t5738,t574,t5748,t5749,t575,t5771,t5778,t5781,t5782,t5793,t5799,t5808,t5816,t5821,t5823,t5824,t5829,t5847,t5853,t587,t5891,t5917,t5926,t595,t5950,t5952,t5975,t5985,t5986,t5988,t5989,t5997,t6020,t603,t6049,t6076,t6077,t6089,t6090,t6091,t61,t6103,t6104,t6105,t6106,t6117,t6124,t6125,t6129,t6137,t6138,t614,t6147,t6167,t6217,t6219,t6233,t6239,t6252,t6255,t628,t6286,t629,t6304,t6311,t6314,t6319,t6325,t634,t6374,t6381,t6388,t6389,t6399,t6409,t641,t6410,t6422,t6433,t6434,t6445,t6448,t6456,t6457,t6458,t6472,t6476,t6485,t6486,t6487,t65,t651,t6515,t6521,t6569,t657,t6597,t6600,t6604,t6607,t6608,t6611,t6612,t6613,t6614,t6615,t6616,t6617,t6618,t6619,t6620,t6632,t6633,t6635,t6636,t6637,t664,t6640,t6645,t6646,t665,t6658,t666,t6668,t667,t668,t6681,t669,t6734,t675,t6776,t6779,t6782,t6783,t6784,t6787,t6788,t6789,t6790,t6791,t6792,t6793,t6794,t6795,t6796,t6797,t6798,t68,t6801,t6808,t6809,t6811,t6814,t6818,t6825,t6829,t6831,t6838,t6842,t6843,t6845,t6846,t6848,t6851,t6860,t6862,t6865,t6868,t6870,t6872,t6874,t6876,t6878,t6880,t6883,t6885,t6887,t6889,t6892,t6894,t6895,t6897,t693,t7,t71,t721,t724,t73,t731,t732,t736,t741,t753,t754,t755,t757,t765,t769,t772,t774,t776,t778,t795,t797,t799,t8,t802,t803,t806,t817,t818,t820,t828,t831,t838,t843,t852,t853,t855,t865,t867,t868,t870,t871,t872,t876,t886,t9,t901,t902,t903,t907,t909,t925,t926,t947,t949,t952,t964,t972,t977,t983,t991,t993,t994,t995});
end
function C = ft_14(ct)
B_cg_H = ct{1};
ITail = ct{2};
Mb = ct{3};
Mm = ct{4};
Mt = ct{5};
T_cg_H = ct{6};
dphi1 = ct{7};
dphi2 = ct{8};
dpsi1 = ct{9};
dth1 = ct{10};
dth2 = ct{11};
dx = ct{12};
dy = ct{13};
dz = ct{14};
t10 = ct{15};
t1005 = ct{16};
t1007 = ct{17};
t1008 = ct{18};
t1009 = ct{19};
t1013 = ct{20};
t1016 = ct{21};
t1017 = ct{22};
t1018 = ct{23};
t1019 = ct{24};
t1023 = ct{25};
t1029 = ct{26};
t103 = ct{27};
t1037 = ct{28};
t1047 = ct{29};
t105 = ct{30};
t1053 = ct{31};
t1059 = ct{32};
t1060 = ct{33};
t1064 = ct{34};
t1079 = ct{35};
t1084 = ct{36};
t1086 = ct{37};
t1088 = ct{38};
t1097 = ct{39};
t1099 = ct{40};
t11 = ct{41};
t1102 = ct{42};
t1108 = ct{43};
t1113 = ct{44};
t1121 = ct{45};
t1129 = ct{46};
t1137 = ct{47};
t1138 = ct{48};
t1139 = ct{49};
t1141 = ct{50};
t1142 = ct{51};
t1143 = ct{52};
t1147 = ct{53};
t1149 = ct{54};
t1153 = ct{55};
t1157 = ct{56};
t1159 = ct{57};
t1167 = ct{58};
t1169 = ct{59};
t1170 = ct{60};
t1173 = ct{61};
t1176 = ct{62};
t1178 = ct{63};
t1179 = ct{64};
t1181 = ct{65};
t1185 = ct{66};
t1189 = ct{67};
t1193 = ct{68};
t1194 = ct{69};
t1195 = ct{70};
t120 = ct{71};
t1203 = ct{72};
t1205 = ct{73};
t1206 = ct{74};
t1215 = ct{75};
t1221 = ct{76};
t1223 = ct{77};
t1224 = ct{78};
t1225 = ct{79};
t1228 = ct{80};
t1229 = ct{81};
t1230 = ct{82};
t1234 = ct{83};
t1240 = ct{84};
t1242 = ct{85};
t1245 = ct{86};
t1247 = ct{87};
t1250 = ct{88};
t1252 = ct{89};
t1253 = ct{90};
t1255 = ct{91};
t1260 = ct{92};
t1261 = ct{93};
t1262 = ct{94};
t1264 = ct{95};
t1265 = ct{96};
t1268 = ct{97};
t1283 = ct{98};
t1291 = ct{99};
t130 = ct{100};
t1301 = ct{101};
t1304 = ct{102};
t1305 = ct{103};
t1309 = ct{104};
t1322 = ct{105};
t1328 = ct{106};
t1331 = ct{107};
t1332 = ct{108};
t1334 = ct{109};
t1337 = ct{110};
t1338 = ct{111};
t134 = ct{112};
t1343 = ct{113};
t1345 = ct{114};
t1352 = ct{115};
t1354 = ct{116};
t1355 = ct{117};
t1360 = ct{118};
t1362 = ct{119};
t1365 = ct{120};
t1366 = ct{121};
t1368 = ct{122};
t1370 = ct{123};
t1371 = ct{124};
t1374 = ct{125};
t1381 = ct{126};
t1382 = ct{127};
t1384 = ct{128};
t1386 = ct{129};
t1388 = ct{130};
t1389 = ct{131};
t1394 = ct{132};
t1395 = ct{133};
t1396 = ct{134};
t1412 = ct{135};
t1413 = ct{136};
t1421 = ct{137};
t1426 = ct{138};
t1427 = ct{139};
t1430 = ct{140};
t1431 = ct{141};
t1435 = ct{142};
t144 = ct{143};
t1441 = ct{144};
t1443 = ct{145};
t1446 = ct{146};
t1456 = ct{147};
t1465 = ct{148};
t1466 = ct{149};
t1470 = ct{150};
t1487 = ct{151};
t1495 = ct{152};
t15 = ct{153};
t1505 = ct{154};
t1506 = ct{155};
t1510 = ct{156};
t1512 = ct{157};
t1521 = ct{158};
t1528 = ct{159};
t1531 = ct{160};
t1535 = ct{161};
t1540 = ct{162};
t1544 = ct{163};
t1552 = ct{164};
t1558 = ct{165};
t1568 = ct{166};
t1575 = ct{167};
t1578 = ct{168};
t1581 = ct{169};
t1586 = ct{170};
t1593 = ct{171};
t1598 = ct{172};
t1609 = ct{173};
t161 = ct{174};
t1618 = ct{175};
t1619 = ct{176};
t1620 = ct{177};
t1624 = ct{178};
t1635 = ct{179};
t1645 = ct{180};
t1646 = ct{181};
t1651 = ct{182};
t1652 = ct{183};
t1654 = ct{184};
t1660 = ct{185};
t1661 = ct{186};
t1664 = ct{187};
t1667 = ct{188};
t1672 = ct{189};
t1676 = ct{190};
t1681 = ct{191};
t1685 = ct{192};
t1692 = ct{193};
t1693 = ct{194};
t1694 = ct{195};
t1698 = ct{196};
t1701 = ct{197};
t1702 = ct{198};
t1703 = ct{199};
t1705 = ct{200};
t1706 = ct{201};
t1718 = ct{202};
t1727 = ct{203};
t1730 = ct{204};
t1734 = ct{205};
t1735 = ct{206};
t1742 = ct{207};
t1746 = ct{208};
t1751 = ct{209};
t1759 = ct{210};
t1761 = ct{211};
t1763 = ct{212};
t1771 = ct{213};
t1774 = ct{214};
t1784 = ct{215};
t1785 = ct{216};
t1786 = ct{217};
t1787 = ct{218};
t1789 = ct{219};
t1790 = ct{220};
t1792 = ct{221};
t1799 = ct{222};
t1802 = ct{223};
t1806 = ct{224};
t1810 = ct{225};
t1813 = ct{226};
t1832 = ct{227};
t1846 = ct{228};
t1851 = ct{229};
t1853 = ct{230};
t1855 = ct{231};
t1858 = ct{232};
t1865 = ct{233};
t1866 = ct{234};
t1867 = ct{235};
t1882 = ct{236};
t1883 = ct{237};
t1898 = ct{238};
t1899 = ct{239};
t1907 = ct{240};
t1910 = ct{241};
t1915 = ct{242};
t1917 = ct{243};
t1918 = ct{244};
t1928 = ct{245};
t1929 = ct{246};
t1932 = ct{247};
t1938 = ct{248};
t1939 = ct{249};
t1942 = ct{250};
t195 = ct{251};
t1956 = ct{252};
t1957 = ct{253};
t1959 = ct{254};
t1962 = ct{255};
t1964 = ct{256};
t1965 = ct{257};
t197 = ct{258};
t1970 = ct{259};
t1971 = ct{260};
t1974 = ct{261};
t1976 = ct{262};
t1977 = ct{263};
t1979 = ct{264};
t1981 = ct{265};
t1983 = ct{266};
t1997 = ct{267};
t2 = ct{268};
t2000 = ct{269};
t2002 = ct{270};
t2007 = ct{271};
t2008 = ct{272};
t2015 = ct{273};
t2020 = ct{274};
t2032 = ct{275};
t2037 = ct{276};
t2038 = ct{277};
t2047 = ct{278};
t2049 = ct{279};
t2057 = ct{280};
t2058 = ct{281};
t2059 = ct{282};
t2062 = ct{283};
t2064 = ct{284};
t2067 = ct{285};
t2072 = ct{286};
t2075 = ct{287};
t2076 = ct{288};
t2082 = ct{289};
t2083 = ct{290};
t2086 = ct{291};
t2087 = ct{292};
t2088 = ct{293};
t2096 = ct{294};
t2104 = ct{295};
t2110 = ct{296};
t2111 = ct{297};
t2123 = ct{298};
t2131 = ct{299};
t2134 = ct{300};
t2135 = ct{301};
t2137 = ct{302};
t2139 = ct{303};
t214 = ct{304};
t2141 = ct{305};
t2147 = ct{306};
t2148 = ct{307};
t2150 = ct{308};
t2152 = ct{309};
t2155 = ct{310};
t2156 = ct{311};
t2158 = ct{312};
t2174 = ct{313};
t2175 = ct{314};
t2190 = ct{315};
t2191 = ct{316};
t2202 = ct{317};
t2203 = ct{318};
t2206 = ct{319};
t2208 = ct{320};
t2210 = ct{321};
t2212 = ct{322};
t2215 = ct{323};
t2218 = ct{324};
t2220 = ct{325};
t2222 = ct{326};
t2225 = ct{327};
t2227 = ct{328};
t2237 = ct{329};
t2240 = ct{330};
t2241 = ct{331};
t2242 = ct{332};
t2243 = ct{333};
t2247 = ct{334};
t2248 = ct{335};
t2254 = ct{336};
t2259 = ct{337};
t2271 = ct{338};
t2274 = ct{339};
t2282 = ct{340};
t2287 = ct{341};
t2293 = ct{342};
t2305 = ct{343};
t2308 = ct{344};
t2312 = ct{345};
t2317 = ct{346};
t2319 = ct{347};
t2322 = ct{348};
t2325 = ct{349};
t2339 = ct{350};
t2342 = ct{351};
t2347 = ct{352};
t2348 = ct{353};
t2360 = ct{354};
t2361 = ct{355};
t2364 = ct{356};
t2368 = ct{357};
t2387 = ct{358};
t2388 = ct{359};
t2389 = ct{360};
t2390 = ct{361};
t24 = ct{362};
t2401 = ct{363};
t2404 = ct{364};
t2409 = ct{365};
t2412 = ct{366};
t2413 = ct{367};
t2419 = ct{368};
t2420 = ct{369};
t2430 = ct{370};
t2434 = ct{371};
t2435 = ct{372};
t2436 = ct{373};
t2438 = ct{374};
t2447 = ct{375};
t2449 = ct{376};
t2463 = ct{377};
t2468 = ct{378};
t2472 = ct{379};
t2479 = ct{380};
t2483 = ct{381};
t2487 = ct{382};
t2489 = ct{383};
t2495 = ct{384};
t2496 = ct{385};
t25 = ct{386};
t2501 = ct{387};
t2503 = ct{388};
t2504 = ct{389};
t2512 = ct{390};
t2514 = ct{391};
t2518 = ct{392};
t2524 = ct{393};
t2527 = ct{394};
t2528 = ct{395};
t2536 = ct{396};
t2547 = ct{397};
t2563 = ct{398};
t2564 = ct{399};
t2568 = ct{400};
t2571 = ct{401};
t2573 = ct{402};
t2574 = ct{403};
t2576 = ct{404};
t2578 = ct{405};
t2579 = ct{406};
t2582 = ct{407};
t2587 = ct{408};
t259 = ct{409};
t2590 = ct{410};
t2591 = ct{411};
t2597 = ct{412};
t26 = ct{413};
t260 = ct{414};
t2600 = ct{415};
t2605 = ct{416};
t2613 = ct{417};
t2616 = ct{418};
t2617 = ct{419};
t2621 = ct{420};
t2627 = ct{421};
t2632 = ct{422};
t2638 = ct{423};
t2657 = ct{424};
t2660 = ct{425};
t2663 = ct{426};
t2665 = ct{427};
t2669 = ct{428};
t2679 = ct{429};
t2684 = ct{430};
t2688 = ct{431};
t2692 = ct{432};
t2696 = ct{433};
t2699 = ct{434};
t27 = ct{435};
t2700 = ct{436};
t2706 = ct{437};
t2708 = ct{438};
t2712 = ct{439};
t2715 = ct{440};
t2717 = ct{441};
t2718 = ct{442};
t2722 = ct{443};
t2723 = ct{444};
t2730 = ct{445};
t2737 = ct{446};
t2738 = ct{447};
t2743 = ct{448};
t2754 = ct{449};
t2759 = ct{450};
t276 = ct{451};
t2763 = ct{452};
t277 = ct{453};
t2785 = ct{454};
t2787 = ct{455};
t2791 = ct{456};
t2796 = ct{457};
t2797 = ct{458};
t2799 = ct{459};
t2803 = ct{460};
t2811 = ct{461};
t2816 = ct{462};
t2821 = ct{463};
t2823 = ct{464};
t2824 = ct{465};
t2825 = ct{466};
t2829 = ct{467};
t283 = ct{468};
t2831 = ct{469};
t2833 = ct{470};
t284 = ct{471};
t2843 = ct{472};
t2845 = ct{473};
t2847 = ct{474};
t2849 = ct{475};
t285 = ct{476};
t286 = ct{477};
t2860 = ct{478};
t2868 = ct{479};
t287 = ct{480};
t2871 = ct{481};
t2875 = ct{482};
t2876 = ct{483};
t2877 = ct{484};
t2878 = ct{485};
t288 = ct{486};
t2883 = ct{487};
t2889 = ct{488};
t289 = ct{489};
t2899 = ct{490};
t290 = ct{491};
t291 = ct{492};
t2914 = ct{493};
t2915 = ct{494};
t2918 = ct{495};
t292 = ct{496};
t2920 = ct{497};
t2921 = ct{498};
t2927 = ct{499};
t293 = ct{500};
t2930 = ct{501};
t2936 = ct{502};
t2937 = ct{503};
t294 = ct{504};
t2942 = ct{505};
t2944 = ct{506};
t2945 = ct{507};
t2950 = ct{508};
t2952 = ct{509};
t2956 = ct{510};
t2962 = ct{511};
t2965 = ct{512};
t2970 = ct{513};
t2972 = ct{514};
t2978 = ct{515};
t2981 = ct{516};
t2994 = ct{517};
t2997 = ct{518};
t3 = ct{519};
t3008 = ct{520};
t3009 = ct{521};
t3012 = ct{522};
t3022 = ct{523};
t3031 = ct{524};
t3034 = ct{525};
t304 = ct{526};
t3054 = ct{527};
t3062 = ct{528};
t3064 = ct{529};
t3070 = ct{530};
t3076 = ct{531};
t3080 = ct{532};
t3082 = ct{533};
t3084 = ct{534};
t3086 = ct{535};
t3087 = ct{536};
t3093 = ct{537};
t3096 = ct{538};
t3105 = ct{539};
t3113 = ct{540};
t3121 = ct{541};
t3122 = ct{542};
t3131 = ct{543};
t3138 = ct{544};
t3139 = ct{545};
t3147 = ct{546};
t3155 = ct{547};
t3160 = ct{548};
t3161 = ct{549};
t3167 = ct{550};
t3169 = ct{551};
t3178 = ct{552};
t3186 = ct{553};
t3192 = ct{554};
t3199 = ct{555};
t3206 = ct{556};
t3207 = ct{557};
t3232 = ct{558};
t3235 = ct{559};
t3236 = ct{560};
t3244 = ct{561};
t3247 = ct{562};
t3248 = ct{563};
t3252 = ct{564};
t3261 = ct{565};
t3263 = ct{566};
t3265 = ct{567};
t3266 = ct{568};
t3270 = ct{569};
t3276 = ct{570};
t3278 = ct{571};
t3286 = ct{572};
t3287 = ct{573};
t3289 = ct{574};
t3299 = ct{575};
t3302 = ct{576};
t3307 = ct{577};
t3311 = ct{578};
t3312 = ct{579};
t3315 = ct{580};
t3325 = ct{581};
t3326 = ct{582};
t3329 = ct{583};
t3331 = ct{584};
t3341 = ct{585};
t3344 = ct{586};
t3347 = ct{587};
t3357 = ct{588};
t3378 = ct{589};
t3387 = ct{590};
t3390 = ct{591};
t3391 = ct{592};
t3392 = ct{593};
t3403 = ct{594};
t3407 = ct{595};
t3412 = ct{596};
t3413 = ct{597};
t3414 = ct{598};
t3415 = ct{599};
t3419 = ct{600};
t3423 = ct{601};
t3424 = ct{602};
t3427 = ct{603};
t3431 = ct{604};
t3432 = ct{605};
t3433 = ct{606};
t3437 = ct{607};
t3438 = ct{608};
t3439 = ct{609};
t3442 = ct{610};
t3445 = ct{611};
t3448 = ct{612};
t3449 = ct{613};
t3458 = ct{614};
t3460 = ct{615};
t3471 = ct{616};
t3475 = ct{617};
t3482 = ct{618};
t3483 = ct{619};
t3485 = ct{620};
t3489 = ct{621};
t3490 = ct{622};
t3494 = ct{623};
t3499 = ct{624};
t3501 = ct{625};
t3506 = ct{626};
t3510 = ct{627};
t3512 = ct{628};
t3516 = ct{629};
t3521 = ct{630};
t3522 = ct{631};
t3523 = ct{632};
t3524 = ct{633};
t3526 = ct{634};
t3528 = ct{635};
t3529 = ct{636};
t3530 = ct{637};
t3531 = ct{638};
t3534 = ct{639};
t3541 = ct{640};
t3543 = ct{641};
t3544 = ct{642};
t3545 = ct{643};
t3548 = ct{644};
t3550 = ct{645};
t3552 = ct{646};
t3553 = ct{647};
t3556 = ct{648};
t3557 = ct{649};
t3563 = ct{650};
t3576 = ct{651};
t3578 = ct{652};
t3582 = ct{653};
t3583 = ct{654};
t3584 = ct{655};
t3587 = ct{656};
t3594 = ct{657};
t3597 = ct{658};
t3598 = ct{659};
t3600 = ct{660};
t3602 = ct{661};
t3614 = ct{662};
t3617 = ct{663};
t3621 = ct{664};
t3627 = ct{665};
t3632 = ct{666};
t3634 = ct{667};
t3638 = ct{668};
t3644 = ct{669};
t3648 = ct{670};
t3649 = ct{671};
t3652 = ct{672};
t3657 = ct{673};
t3659 = ct{674};
t3661 = ct{675};
t3667 = ct{676};
t3679 = ct{677};
t3682 = ct{678};
t3684 = ct{679};
t3697 = ct{680};
t3698 = ct{681};
t3701 = ct{682};
t3704 = ct{683};
t3716 = ct{684};
t3719 = ct{685};
t3720 = ct{686};
t3721 = ct{687};
t3722 = ct{688};
t3735 = ct{689};
t3738 = ct{690};
t3739 = ct{691};
t3745 = ct{692};
t3746 = ct{693};
t3749 = ct{694};
t3756 = ct{695};
t376 = ct{696};
t3764 = ct{697};
t377 = ct{698};
t3770 = ct{699};
t3771 = ct{700};
t3772 = ct{701};
t3773 = ct{702};
t3774 = ct{703};
t3777 = ct{704};
t3780 = ct{705};
t3784 = ct{706};
t3787 = ct{707};
t3791 = ct{708};
t3794 = ct{709};
t381 = ct{710};
t3811 = ct{711};
t3814 = ct{712};
t3815 = ct{713};
t3817 = ct{714};
t382 = ct{715};
t383 = ct{716};
t3834 = ct{717};
t3836 = ct{718};
t3837 = ct{719};
t3841 = ct{720};
t3845 = ct{721};
t3848 = ct{722};
t3858 = ct{723};
t3862 = ct{724};
t3868 = ct{725};
t3870 = ct{726};
t3879 = ct{727};
t390 = ct{728};
t3902 = ct{729};
t3903 = ct{730};
t3906 = ct{731};
t3907 = ct{732};
t3916 = ct{733};
t3923 = ct{734};
t3930 = ct{735};
t3931 = ct{736};
t3932 = ct{737};
t3934 = ct{738};
t3936 = ct{739};
t3937 = ct{740};
t3938 = ct{741};
t394 = ct{742};
t3940 = ct{743};
t3944 = ct{744};
t3947 = ct{745};
t3948 = ct{746};
t3955 = ct{747};
t3957 = ct{748};
t3961 = ct{749};
t3962 = ct{750};
t3965 = ct{751};
t3966 = ct{752};
t3967 = ct{753};
t3969 = ct{754};
t3971 = ct{755};
t3982 = ct{756};
t3983 = ct{757};
t3985 = ct{758};
t4 = ct{759};
t4001 = ct{760};
t4005 = ct{761};
t4009 = ct{762};
t4010 = ct{763};
t4014 = ct{764};
t4023 = ct{765};
t4025 = ct{766};
t4027 = ct{767};
t4028 = ct{768};
t4034 = ct{769};
t4036 = ct{770};
t4042 = ct{771};
t4047 = ct{772};
t4048 = ct{773};
t4051 = ct{774};
t4052 = ct{775};
t4054 = ct{776};
t4056 = ct{777};
t4058 = ct{778};
t4059 = ct{779};
t4061 = ct{780};
t4065 = ct{781};
t4070 = ct{782};
t4071 = ct{783};
t4072 = ct{784};
t4073 = ct{785};
t4074 = ct{786};
t4077 = ct{787};
t4078 = ct{788};
t4081 = ct{789};
t4083 = ct{790};
t4084 = ct{791};
t4087 = ct{792};
t4090 = ct{793};
t4096 = ct{794};
t4098 = ct{795};
t4100 = ct{796};
t4105 = ct{797};
t411 = ct{798};
t4111 = ct{799};
t4112 = ct{800};
t4115 = ct{801};
t412 = ct{802};
t4132 = ct{803};
t4135 = ct{804};
t4137 = ct{805};
t4138 = ct{806};
t414 = ct{807};
t4141 = ct{808};
t4143 = ct{809};
t4144 = ct{810};
t4145 = ct{811};
t415 = ct{812};
t4152 = ct{813};
t4160 = ct{814};
t4162 = ct{815};
t4164 = ct{816};
t4169 = ct{817};
t4171 = ct{818};
t4173 = ct{819};
t4184 = ct{820};
t4189 = ct{821};
t4196 = ct{822};
t4197 = ct{823};
t420 = ct{824};
t4208 = ct{825};
t421 = ct{826};
t4212 = ct{827};
t4213 = ct{828};
t4214 = ct{829};
t4215 = ct{830};
t4217 = ct{831};
t4223 = ct{832};
t4224 = ct{833};
t4225 = ct{834};
t4227 = ct{835};
t4231 = ct{836};
t4233 = ct{837};
t4236 = ct{838};
t4237 = ct{839};
t4245 = ct{840};
t4247 = ct{841};
t425 = ct{842};
t4255 = ct{843};
t4256 = ct{844};
t4257 = ct{845};
t4258 = ct{846};
t4268 = ct{847};
t4271 = ct{848};
t4272 = ct{849};
t4273 = ct{850};
t4274 = ct{851};
t4276 = ct{852};
t4277 = ct{853};
t4281 = ct{854};
t4282 = ct{855};
t4286 = ct{856};
t4296 = ct{857};
t430 = ct{858};
t4300 = ct{859};
t4301 = ct{860};
t4309 = ct{861};
t431 = ct{862};
t4310 = ct{863};
t4311 = ct{864};
t4313 = ct{865};
t4318 = ct{866};
t4323 = ct{867};
t4324 = ct{868};
t4326 = ct{869};
t433 = ct{870};
t4341 = ct{871};
t4342 = ct{872};
t4343 = ct{873};
t4344 = ct{874};
t4346 = ct{875};
t4350 = ct{876};
t4352 = ct{877};
t4354 = ct{878};
t4355 = ct{879};
t4356 = ct{880};
t4357 = ct{881};
t436 = ct{882};
t4371 = ct{883};
t4374 = ct{884};
t4379 = ct{885};
t4382 = ct{886};
t4392 = ct{887};
t4393 = ct{888};
t4395 = ct{889};
t4399 = ct{890};
t44 = ct{891};
t4401 = ct{892};
t4403 = ct{893};
t4404 = ct{894};
t4407 = ct{895};
t4408 = ct{896};
t4409 = ct{897};
t4412 = ct{898};
t4414 = ct{899};
t4415 = ct{900};
t4416 = ct{901};
t4418 = ct{902};
t4422 = ct{903};
t4435 = ct{904};
t4437 = ct{905};
t4439 = ct{906};
t4440 = ct{907};
t4444 = ct{908};
t4447 = ct{909};
t4449 = ct{910};
t445 = ct{911};
t4451 = ct{912};
t4452 = ct{913};
t4454 = ct{914};
t4457 = ct{915};
t4458 = ct{916};
t4459 = ct{917};
t4461 = ct{918};
t4462 = ct{919};
t4469 = ct{920};
t4471 = ct{921};
t4476 = ct{922};
t4479 = ct{923};
t4480 = ct{924};
t4481 = ct{925};
t4483 = ct{926};
t4484 = ct{927};
t4485 = ct{928};
t4487 = ct{929};
t4490 = ct{930};
t4493 = ct{931};
t4498 = ct{932};
t4500 = ct{933};
t4502 = ct{934};
t4503 = ct{935};
t4505 = ct{936};
t451 = ct{937};
t4510 = ct{938};
t4512 = ct{939};
t4514 = ct{940};
t4515 = ct{941};
t4517 = ct{942};
t4518 = ct{943};
t4519 = ct{944};
t4521 = ct{945};
t4522 = ct{946};
t4528 = ct{947};
t4529 = ct{948};
t4531 = ct{949};
t4532 = ct{950};
t4536 = ct{951};
t4538 = ct{952};
t4540 = ct{953};
t4542 = ct{954};
t4545 = ct{955};
t4546 = ct{956};
t4549 = ct{957};
t4550 = ct{958};
t4551 = ct{959};
t4553 = ct{960};
t4555 = ct{961};
t4556 = ct{962};
t4573 = ct{963};
t4575 = ct{964};
t4576 = ct{965};
t4577 = ct{966};
t4578 = ct{967};
t4581 = ct{968};
t4583 = ct{969};
t4584 = ct{970};
t4585 = ct{971};
t4586 = ct{972};
t4588 = ct{973};
t459 = ct{974};
t4590 = ct{975};
t4591 = ct{976};
t4592 = ct{977};
t4596 = ct{978};
t4597 = ct{979};
t4598 = ct{980};
t4602 = ct{981};
t4603 = ct{982};
t4605 = ct{983};
t4606 = ct{984};
t4609 = ct{985};
t4617 = ct{986};
t4618 = ct{987};
t4623 = ct{988};
t4626 = ct{989};
t4629 = ct{990};
t4634 = ct{991};
t4638 = ct{992};
t4639 = ct{993};
t4640 = ct{994};
t4644 = ct{995};
t4645 = ct{996};
t4646 = ct{997};
t4647 = ct{998};
t4649 = ct{999};
t465 = ct{1000};
t4652 = ct{1001};
t4657 = ct{1002};
t4658 = ct{1003};
t4667 = ct{1004};
t4668 = ct{1005};
t4669 = ct{1006};
t4672 = ct{1007};
t4675 = ct{1008};
t4681 = ct{1009};
t4686 = ct{1010};
t4689 = ct{1011};
t4691 = ct{1012};
t4695 = ct{1013};
t4696 = ct{1014};
t4698 = ct{1015};
t4701 = ct{1016};
t4704 = ct{1017};
t4712 = ct{1018};
t4722 = ct{1019};
t4735 = ct{1020};
t4736 = ct{1021};
t4737 = ct{1022};
t4738 = ct{1023};
t4752 = ct{1024};
t4753 = ct{1025};
t4756 = ct{1026};
t4770 = ct{1027};
t4775 = ct{1028};
t4783 = ct{1029};
t4785 = ct{1030};
t4786 = ct{1031};
t4787 = ct{1032};
t4790 = ct{1033};
t4793 = ct{1034};
t4796 = ct{1035};
t48 = ct{1036};
t4814 = ct{1037};
t4816 = ct{1038};
t4820 = ct{1039};
t4821 = ct{1040};
t4823 = ct{1041};
t4830 = ct{1042};
t4834 = ct{1043};
t4849 = ct{1044};
t485 = ct{1045};
t4850 = ct{1046};
t4851 = ct{1047};
t4858 = ct{1048};
t4861 = ct{1049};
t4867 = ct{1050};
t4870 = ct{1051};
t4874 = ct{1052};
t4876 = ct{1053};
t4877 = ct{1054};
t488 = ct{1055};
t4881 = ct{1056};
t4882 = ct{1057};
t4883 = ct{1058};
t4897 = ct{1059};
t49 = ct{1060};
t4900 = ct{1061};
t4908 = ct{1062};
t4922 = ct{1063};
t4923 = ct{1064};
t4928 = ct{1065};
t4936 = ct{1066};
t4945 = ct{1067};
t4949 = ct{1068};
t4958 = ct{1069};
t4959 = ct{1070};
t496 = ct{1071};
t4960 = ct{1072};
t4961 = ct{1073};
t4964 = ct{1074};
t4972 = ct{1075};
t4980 = ct{1076};
t4989 = ct{1077};
t4995 = ct{1078};
t5 = ct{1079};
t50 = ct{1080};
t5006 = ct{1081};
t5013 = ct{1082};
t502 = ct{1083};
t5022 = ct{1084};
t5023 = ct{1085};
t5070 = ct{1086};
t5071 = ct{1087};
t5089 = ct{1088};
t5099 = ct{1089};
t51 = ct{1090};
t5136 = ct{1091};
t5175 = ct{1092};
t519 = ct{1093};
t5208 = ct{1094};
t5216 = ct{1095};
t523 = ct{1096};
t524 = ct{1097};
t527 = ct{1098};
t5274 = ct{1099};
t5280 = ct{1100};
t5294 = ct{1101};
t530 = ct{1102};
t5300 = ct{1103};
t5304 = ct{1104};
t5308 = ct{1105};
t5313 = ct{1106};
t534 = ct{1107};
t5351 = ct{1108};
t5354 = ct{1109};
t537 = ct{1110};
t5370 = ct{1111};
t5371 = ct{1112};
t5372 = ct{1113};
t5373 = ct{1114};
t5375 = ct{1115};
t5382 = ct{1116};
t539 = ct{1117};
t5392 = ct{1118};
t5394 = ct{1119};
t54 = ct{1120};
t5402 = ct{1121};
t5404 = ct{1122};
t5405 = ct{1123};
t541 = ct{1124};
t542 = ct{1125};
t5421 = ct{1126};
t5434 = ct{1127};
t5435 = ct{1128};
t544 = ct{1129};
t5442 = ct{1130};
t546 = ct{1131};
t5474 = ct{1132};
t55 = ct{1133};
t550 = ct{1134};
t5502 = ct{1135};
t5509 = ct{1136};
t5514 = ct{1137};
t5519 = ct{1138};
t553 = ct{1139};
t5548 = ct{1140};
t5556 = ct{1141};
t5566 = ct{1142};
t557 = ct{1143};
t558 = ct{1144};
t5597 = ct{1145};
t56 = ct{1146};
t5607 = ct{1147};
t5627 = ct{1148};
t5644 = ct{1149};
t5648 = ct{1150};
t5660 = ct{1151};
t5665 = ct{1152};
t5705 = ct{1153};
t5727 = ct{1154};
t5729 = ct{1155};
t573 = ct{1156};
t5733 = ct{1157};
t5738 = ct{1158};
t574 = ct{1159};
t5748 = ct{1160};
t5749 = ct{1161};
t575 = ct{1162};
t5771 = ct{1163};
t5778 = ct{1164};
t5781 = ct{1165};
t5782 = ct{1166};
t5793 = ct{1167};
t5799 = ct{1168};
t5808 = ct{1169};
t5816 = ct{1170};
t5821 = ct{1171};
t5823 = ct{1172};
t5824 = ct{1173};
t5829 = ct{1174};
t5847 = ct{1175};
t5853 = ct{1176};
t587 = ct{1177};
t5891 = ct{1178};
t5917 = ct{1179};
t5926 = ct{1180};
t595 = ct{1181};
t5950 = ct{1182};
t5952 = ct{1183};
t5975 = ct{1184};
t5985 = ct{1185};
t5986 = ct{1186};
t5988 = ct{1187};
t5989 = ct{1188};
t5997 = ct{1189};
t6020 = ct{1190};
t603 = ct{1191};
t6049 = ct{1192};
t6076 = ct{1193};
t6077 = ct{1194};
t6089 = ct{1195};
t6090 = ct{1196};
t6091 = ct{1197};
t61 = ct{1198};
t6103 = ct{1199};
t6104 = ct{1200};
t6105 = ct{1201};
t6106 = ct{1202};
t6117 = ct{1203};
t6124 = ct{1204};
t6125 = ct{1205};
t6129 = ct{1206};
t6137 = ct{1207};
t6138 = ct{1208};
t614 = ct{1209};
t6147 = ct{1210};
t6167 = ct{1211};
t6217 = ct{1212};
t6219 = ct{1213};
t6233 = ct{1214};
t6239 = ct{1215};
t6252 = ct{1216};
t6255 = ct{1217};
t628 = ct{1218};
t6286 = ct{1219};
t629 = ct{1220};
t6304 = ct{1221};
t6311 = ct{1222};
t6314 = ct{1223};
t6319 = ct{1224};
t6325 = ct{1225};
t634 = ct{1226};
t6374 = ct{1227};
t6381 = ct{1228};
t6388 = ct{1229};
t6389 = ct{1230};
t6399 = ct{1231};
t6409 = ct{1232};
t641 = ct{1233};
t6410 = ct{1234};
t6422 = ct{1235};
t6433 = ct{1236};
t6434 = ct{1237};
t6445 = ct{1238};
t6448 = ct{1239};
t6456 = ct{1240};
t6457 = ct{1241};
t6458 = ct{1242};
t6472 = ct{1243};
t6476 = ct{1244};
t6485 = ct{1245};
t6486 = ct{1246};
t6487 = ct{1247};
t65 = ct{1248};
t651 = ct{1249};
t6515 = ct{1250};
t6521 = ct{1251};
t6569 = ct{1252};
t657 = ct{1253};
t6597 = ct{1254};
t6600 = ct{1255};
t6604 = ct{1256};
t6607 = ct{1257};
t6608 = ct{1258};
t6611 = ct{1259};
t6612 = ct{1260};
t6613 = ct{1261};
t6614 = ct{1262};
t6615 = ct{1263};
t6616 = ct{1264};
t6617 = ct{1265};
t6618 = ct{1266};
t6619 = ct{1267};
t6620 = ct{1268};
t6632 = ct{1269};
t6633 = ct{1270};
t6635 = ct{1271};
t6636 = ct{1272};
t6637 = ct{1273};
t664 = ct{1274};
t6640 = ct{1275};
t6645 = ct{1276};
t6646 = ct{1277};
t665 = ct{1278};
t6658 = ct{1279};
t666 = ct{1280};
t6668 = ct{1281};
t667 = ct{1282};
t668 = ct{1283};
t6681 = ct{1284};
t669 = ct{1285};
t6734 = ct{1286};
t675 = ct{1287};
t6776 = ct{1288};
t6779 = ct{1289};
t6782 = ct{1290};
t6783 = ct{1291};
t6784 = ct{1292};
t6787 = ct{1293};
t6788 = ct{1294};
t6789 = ct{1295};
t6790 = ct{1296};
t6791 = ct{1297};
t6792 = ct{1298};
t6793 = ct{1299};
t6794 = ct{1300};
t6795 = ct{1301};
t6796 = ct{1302};
t6797 = ct{1303};
t6798 = ct{1304};
t68 = ct{1305};
t6801 = ct{1306};
t6808 = ct{1307};
t6809 = ct{1308};
t6811 = ct{1309};
t6814 = ct{1310};
t6818 = ct{1311};
t6825 = ct{1312};
t6829 = ct{1313};
t6831 = ct{1314};
t6838 = ct{1315};
t6842 = ct{1316};
t6843 = ct{1317};
t6845 = ct{1318};
t6846 = ct{1319};
t6848 = ct{1320};
t6851 = ct{1321};
t6860 = ct{1322};
t6862 = ct{1323};
t6865 = ct{1324};
t6868 = ct{1325};
t6870 = ct{1326};
t6872 = ct{1327};
t6874 = ct{1328};
t6876 = ct{1329};
t6878 = ct{1330};
t6880 = ct{1331};
t6883 = ct{1332};
t6885 = ct{1333};
t6887 = ct{1334};
t6889 = ct{1335};
t6892 = ct{1336};
t6894 = ct{1337};
t6895 = ct{1338};
t6897 = ct{1339};
t693 = ct{1340};
t7 = ct{1341};
t71 = ct{1342};
t721 = ct{1343};
t724 = ct{1344};
t73 = ct{1345};
t731 = ct{1346};
t732 = ct{1347};
t736 = ct{1348};
t741 = ct{1349};
t753 = ct{1350};
t754 = ct{1351};
t755 = ct{1352};
t757 = ct{1353};
t765 = ct{1354};
t769 = ct{1355};
t772 = ct{1356};
t774 = ct{1357};
t776 = ct{1358};
t778 = ct{1359};
t795 = ct{1360};
t797 = ct{1361};
t799 = ct{1362};
t8 = ct{1363};
t802 = ct{1364};
t803 = ct{1365};
t806 = ct{1366};
t817 = ct{1367};
t818 = ct{1368};
t820 = ct{1369};
t828 = ct{1370};
t831 = ct{1371};
t838 = ct{1372};
t843 = ct{1373};
t852 = ct{1374};
t853 = ct{1375};
t855 = ct{1376};
t865 = ct{1377};
t867 = ct{1378};
t868 = ct{1379};
t870 = ct{1380};
t871 = ct{1381};
t872 = ct{1382};
t876 = ct{1383};
t886 = ct{1384};
t9 = ct{1385};
t901 = ct{1386};
t902 = ct{1387};
t903 = ct{1388};
t907 = ct{1389};
t909 = ct{1390};
t925 = ct{1391};
t926 = ct{1392};
t947 = ct{1393};
t949 = ct{1394};
t952 = ct{1395};
t964 = ct{1396};
t972 = ct{1397};
t977 = ct{1398};
t983 = ct{1399};
t991 = ct{1400};
t993 = ct{1401};
t994 = ct{1402};
t995 = ct{1403};
t6899 = t6476+t6515+t6521+t6825+t6862+t6865+t6874;
t6901 = t4861+t4870+t6848+t6876+t6878+t6887;
t6893 = t4876+t4958+t4959+t6801+t6811+t6814+t6818;
t6896 = t5373+t5375+t6809+t6831+t6838+t6843;
t6898 = t5729+t6597+t6600+t6829+t6860+t6868+t6870;
t6900 = t4756+t4790+t4793+t6846+t6872+t6880+t6885;
t6902 = t6020+t6632+t6633+t6851+t6883+t6889+t6892;
et107 = t3265.*9.52624335e-4+t3771.*9.52624335e-4-t4480.*9.52624335e-4-t4556.*9.52624335e-4;
et108 = t1505.*(-t724-t778+t1230+t1291+dphi2.*(t534-t546)).*9.52624335e-4+t4437.*(t534-t546).*9.52624335e-4;
et109 = t2823.*9.53094055e-4+t3235.*9.53094055e-4-t4374.*9.53094055e-4+t4399.*9.53094055e-4+t4484.*9.53094055e-4;
et110 = t4485.*(-9.53094055e-4);
et111 = t1661.*3.367829185e-3+t1976.*3.367829185e-3+t3791.*3.367829185e-3+t3811.*3.367829185e-3+t3814+t3983+t4023-t4027.*3.367829185e-3;
et112 = t4070.*3.367829185e-3+t4144+t4510+t4515+t4583+t4584+t4586+t4590+t4658+t4669;
et113 = t2821+t2823.*3.372786875e-3+t3207+t3235.*3.372786875e-3+t4023+t4137+t4144+t4152+t4271+t4282-t4374.*3.372786875e-3+t4399.*3.372786875e-3+t4484.*3.372786875e-3;
et114 = t4485.*(-3.372786875e-3)+t4583+t4584+t4658+t4669;
et115 = t1661.*8.56645e-6+t1976.*8.56645e-6+t3791.*8.56645e-6+t3811.*8.56645e-6;
et116 = t4027.*(-8.56645e-6)+t4070.*8.56645e-6;
et117 = -t1703+t2015+t3449-t3787+t3916+t3923+t3947-t4371-t4401+t4469+t4493+t5371+t5372+t5404+t5405+t5748+t5749+t5781+t5808+t5986+t5988+t5989+t6103-t6433-t6448-t6645+t6646+t6776+t6779+t6090.*(t867+t1059-t1646-t1705+t1938-t2002)+t4787.*(-t1129+t1139-t2082+t2110+t2123+t8.*t872.*(t534-t546));
et118 = t4454.*(t1970-t1971+t2487+t3161-t3236-t3794-t3817+t1240.*(t105-t465).*3.372786875e-3+t903.*(t534-t546).*3.372786875e-3)+t4551.*(t753+t991-t1771-t1957+t1181.*(t105-t465)+t11.*t381.*(t534-t546))+t6089.*(t753+t991-t1771-t1957+t1181.*(t105-t465)+t11.*t381.*(t534-t546));
et119 = t4476.*(t2215-t2237+t3424+t3427-t3439+t8.*t872.*(t534-t546).*9.52624335e-4)+t6091.*(t1176-t1366+t2434+t2435-t2899+t1430.*(t539+t641));
et120 = t4476.*(t1645+t1965+t2072+t2220-t2242-t2409-t2483-t2504-t3093+t3155+t3261+t3432+t3437-t3442+t1179.*(t103-t544).*3.36554e-3+t3.*t575.*(t105-t465).*3.36554e-3+t8.*t872.*(t534-t546).*3.372816795e-3);
et121 = t4454.*(-t1974+t1240.*(t105-t465).*9.53094055e-4+t903.*(t534-t546).*9.53094055e-4);
et122 = t3961.*(t1786+t1810+t1964+t2047+t2152-t2401-t2797-t2860-t3076+t3167-t3232-t3278+t3582+t3583-t3837+t1430.*(t539+t641).*3.36554e-3+t1181.*(t105-t465).*3.372786875e-3+t11.*t381.*(t534-t546).*3.372786875e-3);
et123 = t3961.*(t1784+t2057-t3080-t3287+t1181.*(t105-t465).*9.53094055e-4+t11.*t381.*(t534-t546).*9.53094055e-4)+t4936.*(-t947+t1240.*(t105-t465)+t903.*(t534-t546))+ITail.*t4490.*(-t947+t1240.*(t105-t465)+t903.*(t534-t546))+ITail.*t4454.*(-t1017+(t1240.*(t105-t465))./2.0+(t903.*(t534-t546))./2.0);
et124 = ITail.*t4522.*(-t1129+t1139-t2082+t2110+t2123+t8.*t872.*(t534-t546))+ITail.*t4476.*(-t1189+t1195-t2210+t2241+t2248+(t8.*t872.*(t534-t546))./2.0)+ITail.*t4071.*(t753+t991-t1771-t1957+t1181.*(t105-t465)+t11.*t381.*(t534-t546))+ITail.*t3961.*(t865+t1086-t1855-t2076+(t1181.*(t105-t465))./2.0+(t11.*t381.*(t534-t546))./2.0)+B_cg_H.*Mb.*t11.*t641.*t3206;
et125 = t1309+t1929+t2282-t2348+t3325+t3957+t3985+t4010+t4257+t4268+t4502+t4503-t5274+t5280-t5294+t5308-t5644+t5648-t5917+t5926+t6077-t6147+t6219-t6304-t6311-t6658+t4476.*(t2591-t3773+t1430.*(t197-t537).*1.90524867e-3);
et126 = t4820.*(t1970-t1971+t2487+t3161-t3236-t3794-t3817+t1240.*(t105-t465).*3.372786875e-3+t903.*(t534-t546).*3.372786875e-3);
et127 = t4820.*(-t1974+t1240.*(t105-t465).*9.53094055e-4+t903.*(t534-t546).*9.53094055e-4)+t6611.*(t1332+t2368+t1512.*(t105-t465))+t5394.*(t820+t1121-t1435+t1997+t2000+t11.*t420.*(t214-t541))+t4787.*(t1396-t2573+t1430.*(t197-t537).*2.0)+t5548.*(-t947+t1240.*(t105-t465)+t903.*(t534-t546))+t6129.*(-t947+t1240.*(t105-t465)+t903.*(t534-t546));
et128 = ITail.*t4476.*(t1368-t2524+t1430.*(t197-t537))+ITail.*t4522.*(t1396-t2573+t1430.*(t197-t537).*2.0)+ITail.*t4867.*(-t947+t1240.*(t105-t465)+t903.*(t534-t546))+ITail.*t4820.*(-t1017+(t1240.*(t105-t465))./2.0+(t903.*(t534-t546))./2.0);
et129 = -t5373-t5375+t6808+t6842+dth2.*(et125+et126+et127+et128);
et130 = dth1.*(t2206+t2293+t3526+t3530+t4005+t4009+t4143+t4171+t4449+t4451+t4529+t4532+t5099+t5136+t5370+t5402-t5421-t5435+t5502+t5509+t5733-t5771+t5975-t5985-t6076-t6167-t6233+t6255+t6314+t6319+t6434-t6681+t5394.*(t995+t1064-t1506+t1598-t1763-t1774)+t4672.*(-t2389+t3634+t1512.*(t105-t465).*9.53094055e-4)+t5304.*(t1332+t2368+t1512.*(t105-t465))+t6620.*(t1332+t2368+t1512.*(t105-t465))+ITail.*t4712.*(t1332+t2368+t1512.*(t105-t465))+ITail.*t4672.*(t1386+t2501+(t1512.*(t105-t465))./2.0));
et131 = t1149.*2.0-t1898.*2.0-t1942.*2.0+t2978.*2.0-t4169.*2.0+t4184.*2.0+t4197.*2.0+t4545.*2.0-t4553.*2.0+t4681.*(t995+t1064-t1506+t1598-t1763-t1774).*2.0-t4277.*(t1867-t1907-t2067+t2190+t2489+t2547+t2568+t2632+t2787+t2845+t2918+t2965+t3086+t3087+t3391+t3412+t3414+t3445).*2.0+t4476.*(t1867-t1907-t1915+t2007+t2568+t2576+t2632+t2715+t2743+t2759+t2918+t2930+t2942+t2965+t3516+t3529+t3541+t3553).*2.0;
et132 = t4672.*(t1970-t1971+t2487+t3161-t3236-t3794-t3817+t1240.*(t105-t465).*3.372786875e-3+t903.*(t534-t546).*3.372786875e-3).*-2.0+t4787.*t4922.*2.0-t4277.*(-t2141+t2259+t2825+t2944+t3121+t3131).*2.0+t4476.*(t2706-t2712+t3512+t3528+t3534+t3552).*2.0;
et133 = t4672.*(-t1974+t1240.*(t105-t465).*9.53094055e-4+t903.*(t534-t546).*9.53094055e-4).*-2.0;
et134 = (t995+t1064-t1506+t1598-t1763-t1774).*(-t1865+t2158+t2487+t3302-t3390-t3794-t3817+t1240.*(t105-t465).*3.36554e-3+t903.*(t534-t546).*3.36554e-3).*2.0;
et135 = t4922.*(-t1865+t1970+t2708+t3161-t3236-t3845-t3870+t1240.*(t105-t465).*3.36554e-3+t903.*(t534-t546).*3.36554e-3).*-2.0-t5304.*(-t947+t1240.*(t105-t465)+t903.*(t534-t546)).*2.0-t6620.*(-t947+t1240.*(t105-t465)+t903.*(t534-t546)).*2.0-ITail.*t4712.*(-t947+t1240.*(t105-t465)+t903.*(t534-t546)).*2.0;
et136 = ITail.*t4672.*(-t1017+(t1240.*(t105-t465))./2.0+(t903.*(t534-t546))./2.0).*-2.0+ITail.*t4310.*(t995+t1064-t1506+t1598-t1763-t1774).*2.0+ITail.*t4277.*(t1088+t1147-t1609+t1652-t1853-t1858).*2.0+ITail.*t4476.*t4960.*2.0+ITail.*t4522.*t4922.*2.0;
et137 = t1703.*-2.0+t3449.*2.0-t3787.*2.0-t3834.*2.0-t4371.*2.0-t4401.*2.0+t4686.*(t1970-t1971+t2487+t3161-t3236-t3794-t3817+t1240.*(t105-t465).*3.372786875e-3+t903.*(t534-t546).*3.372786875e-3).*2.0+t4787.*t4821.*2.0-t4277.*t5392.*2.0+t4476.*t5556.*2.0-t4277.*t6612.*2.0+t4476.*t6613.*2.0;
et138 = (t820+t1121-t1435+t1997+t2000+t11.*t420.*(t214-t541)).*(-t1865+t2158+t2487+t3302-t3390-t3794-t3817+t1240.*(t105-t465).*3.36554e-3+t903.*(t534-t546).*3.36554e-3).*2.0;
et139 = t4686.*(-t1974+t1240.*(t105-t465).*9.53094055e-4+t903.*(t534-t546).*9.53094055e-4).*2.0+t4681.*(t820+t1121-t1435+t1997+t2000+t11.*t420.*(t214-t541)).*2.0;
et140 = t4821.*(-t1865+t1970+t2708+t3161-t3236-t3845-t3870+t1240.*(t105-t465).*3.36554e-3+t903.*(t534-t546).*3.36554e-3).*-2.0-t6611.*(-t947+t1240.*(t105-t465)+t903.*(t534-t546)).*2.0+(-t947+t1240.*(t105-t465)+t903.*(t534-t546)).*(-t1806+t2096+t2605+t2717+t3289+t3438).*2.0+ITail.*t4310.*(t820+t1121-t1435+t1997+t2000+t11.*t420.*(t214-t541)).*2.0;
et141 = ITail.*t4277.*(t907+t1157-t1544+t2086+t2137+(t11.*t420.*(t214-t541))./2.0).*2.0+ITail.*t4686.*(-t1017+(t1240.*(t105-t465))./2.0+(t903.*(t534-t546))./2.0).*2.0-ITail.*(-t947+t1240.*(t105-t465)+t903.*(t534-t546)).*(t853+t1084-t1466-t2032-t2247+(t11.*t542.*(t105-t465))./2.0).*2.0+ITail.*t4522.*t4821.*2.0+ITail.*t4476.*t4874.*2.0;
et142 = t2020.*2.0-t3962.*2.0-t4048.*2.0-t4065.*2.0-t4538.*2.0-t4546.*2.0-t4787.*(t1365-t1443+t2829-t2831-t2833+t1505.*(t534-t546)).*2.0+t4237.*(t1970-t1971+t2487+t3161-t3236-t3794-t3817+t1240.*(t105-t465).*3.372786875e-3+t903.*(t534-t546).*3.372786875e-3).*2.0+t4255.*t4681.*2.0+t4277.*t4668.*2.0+t4476.*t5853.*2.0+t4277.*t6410.*2.0-t4476.*t6422.*2.0;
et143 = t4237.*(-t1974+t1240.*(t105-t465).*9.53094055e-4+t903.*(t534-t546).*9.53094055e-4).*2.0;
et144 = (t1365-t1443+t2829-t2831-t2833+t1505.*(t534-t546)).*(-t1865+t1970+t2708+t3161-t3236-t3845-t3870+t1240.*(t105-t465).*3.36554e-3+t903.*(t534-t546).*3.36554e-3).*2.0;
et145 = t4255.*(-t1865+t2158+t2487+t3302-t3390-t3794-t3817+t1240.*(t105-t465).*3.36554e-3+t903.*(t534-t546).*3.36554e-3).*2.0+t4649.*(-t947+t1240.*(t105-t465)+t903.*(t534-t546)).*2.0+t6409.*(-t947+t1240.*(t105-t465)+t903.*(t534-t546)).*2.0+ITail.*t4286.*(-t947+t1240.*(t105-t465)+t903.*(t534-t546)).*2.0;
et146 = ITail.*t4237.*(-t1017+(t1240.*(t105-t465))./2.0+(t903.*(t534-t546))./2.0).*2.0-ITail.*t4522.*(t1365-t1443+t2829-t2831-t2833+t1505.*(t534-t546)).*2.0+ITail.*t4255.*t4310.*2.0+ITail.*t4277.*t4296.*2.0+ITail.*t4476.*t5175.*2.0;
et147 = (t753+t991-t1771-t1957+t1181.*(t105-t465)+t11.*t381.*(t534-t546)).*(t1970-t1971+t2487+t3161-t3236-t3794-t3817+t1240.*(t105-t465).*3.372786875e-3+t903.*(t534-t546).*3.372786875e-3).*2.0+t4681.*(t867+t1059-t1646-t1705+t1938-t2002).*2.0;
et148 = (-t947+t1240.*(t105-t465)+t903.*(t534-t546)).*(t1786+t1810+t1964+t2047+t2152-t2401-t2797-t2860-t3076+t3167-t3232-t3278+t3582+t3583-t3837+t1430.*(t539+t641).*3.36554e-3+t1181.*(t105-t465).*3.372786875e-3+t11.*t381.*(t534-t546).*3.372786875e-3).*2.0;
et149 = t4277.*(t1692+t1899+t1910+t2152+t2155-t2401-t2936-t2962-t3031-t3147+t3307-t3387+t3582+t3583-t3837+t1430.*(t539+t641).*3.36554e-3+t1181.*(t105-t465).*3.36554e-3+t11.*t381.*(t534-t546).*3.36554e-3).*2.0+t4476.*t5793.*2.0-t4277.*(-t1928+t2254+t2994+t3064+t3407+t3431).*2.0-t4787.*(t1176-t1366+t2434+t2435-t2899+t1430.*(t539+t641)).*2.0;
et150 = (-t1974+t1240.*(t105-t465).*9.53094055e-4+t903.*(t534-t546).*9.53094055e-4).*(t753+t991-t1771-t1957+t1181.*(t105-t465)+t11.*t381.*(t534-t546)).*2.0;
et151 = (-t947+t1240.*(t105-t465)+t903.*(t534-t546)).*(t1784+t2057-t3080-t3287+t1181.*(t105-t465).*9.53094055e-4+t11.*t381.*(t534-t546).*9.53094055e-4).*2.0;
et152 = t4476.*(t1692+t1786+t1910+t1964+t2305-t2600-t2797-t2860-t2936-t3147+t3167-t3232+t3720+t3721-t3903+t1430.*(t539+t641).*3.372816795e-3+t1181.*(t105-t465).*3.36554e-3+t11.*t381.*(t534-t546).*3.36554e-3).*-2.0;
et153 = (t867+t1059-t1646-t1705+t1938-t2002).*(-t1865+t2158+t2487+t3302-t3390-t3794-t3817+t1240.*(t105-t465).*3.36554e-3+t903.*(t534-t546).*3.36554e-3).*2.0;
et154 = (t1176-t1366+t2434+t2435-t2899+t1430.*(t539+t641)).*(-t1865+t1970+t2708+t3161-t3236-t3845-t3870+t1240.*(t105-t465).*3.36554e-3+t903.*(t534-t546).*3.36554e-3).*2.0+ITail.*(-t1017+(t1240.*(t105-t465))./2.0+(t903.*(t534-t546))./2.0).*(t753+t991-t1771-t1957+t1181.*(t105-t465)+t11.*t381.*(t534-t546)).*2.0;
et155 = ITail.*(-t947+t1240.*(t105-t465)+t903.*(t534-t546)).*(t865+t1086-t1855-t2076+(t1181.*(t105-t465))./2.0+(t11.*t381.*(t534-t546))./2.0).*2.0+ITail.*t4310.*(t867+t1059-t1646-t1705+t1938-t2002).*2.0+ITail.*t4277.*(t949+t1142-t1730-t1792+t2049-t2139).*2.0-Mm.*t1169.*(t530+t736).*2.0-Mt.*t2360.*(-t44+t390+t430-t524+t587).*2.0+Mb.*t1382.*t1456.*2.0-Mb.*t3138.*t3139.*2.0-Mb.*t3082.*t3206.*2.0+Mm.*t524.*t595.*2.0+Mm.*t1170.*t1221.*2.0-Mt.*t4112.*t4115.*2.0-Mt.*t4100.*t4132.*2.0-ITail.*t4522.*(t1176-t1366+t2434+t2435-t2899+t1430.*(t539+t641)).*2.0;
et156 = ITail.*t4476.*(t1255-t1465+t2578+t2579-t2997+(t1430.*(t539+t641))./2.0).*-2.0;
et157 = t2821+t3207-t3265.*3.372816795e-3-t3771.*3.372816795e-3+t3814+t3983+t4137+t4152+t4271+t4282+t4480.*3.372816795e-3+t4510+t4515+t4556.*3.372816795e-3+t4586+t4590;
et158 = t1505.*(-t724-t778+t1230+t1291+dphi2.*(t534-t546)).*(-3.372816795e-3)-t4437.*(t534-t546).*3.372816795e-3;
et159 = -t5782.*(et107+et108)+t55.*(t24.*(-1.8563e-7)+t26.*2.3495e-8+t54.*2.3495e-8+t61.*1.8563e-7);
et160 = -t6252.*(-t4087+t4644+t4422.*(t105-t465).*9.53094055e-4)-dpsi1.*t6898-dth1.*t6902-dx.*t6791+dy.*t6795+dz.*t6796-(-t3471+t4531+t4422.*(t105-t465)).*(et109+et110)+(-t2274+t4111+t1510.*(-t488+t603+dpsi1.*(t105-t465)+dth2.*(t103-t544))).*(et111+et112)-(-t3471+t4531+t4422.*(t105-t465)).*(et113+et114)+t304.*t4603-t383.*t4597+t5778.*t6783+t6252.*t6782;
et161 = -t5997.*(t3265+t3771-t4480-t4556+t1505.*(-t724-t778+t1230+t1291+dphi2.*(t534-t546))+t4437.*(t534-t546))-t6784.*(t3265+t3771-t4480-t4556+t1505.*(-t724-t778+t1230+t1291+dphi2.*(t534-t546))+t4437.*(t534-t546))+(-t2274+t4111+t1510.*(-t488+t603+dpsi1.*(t105-t465)+dth2.*(t103-t544))).*(et115+et116);
et162 = t383.*(t26.*3.949132625e-3+t54.*3.949132625e-3+t1301-t1338)-dth2.*(t4850-t6848-t6876-t6878+dphi1.*(et117+et118+et119+et120+et121+et122+et123+et124)+dz.*(t838-t1413+t1672-t2921+Mt.*t420.*(t433-t828+T_cg_H.*(t197-t537))+B_cg_H.*Mb.*t420.*(t197-t537)))+dphi2.*(et129+et130);
et163 = t5778.*(-t3614+t4341+t1510.*(-t488+t603+dpsi1.*(t105-t465)+dth2.*(t103-t544)).*8.56645e-6)-dphi1.*(dth1.*(et131+et132+et133+et134+et135+et136)-dz.*(t757.*2.0+t1586.*2.0-t1735.*2.0-t2669.*2.0+t3617.*2.0+t3756.*2.0+t4225.*2.0+t4258.*2.0+Mm.*t381.*(t530+t736).*2.0)+dth2.*(et137+et138+et139+et140+et141)+dphi2.*(et142+et143+et144+et145+et146)-dphi1.*(et147+et148+et149+et150+et151+et152+et153+et154+et155+et156)+dy.*(t755.*-2.0-t1578.*2.0-t1681.*2.0+t1802.*2.0+t2665.*2.0+t3682.*2.0+t3684.*2.0+t4245.*2.0+t4247.*2.0));
et164 = -t304.*(t24.*1.19846373e-3-t61.*1.19846373e-3+t1305+t1337)+t5782.*(et157+et158)+Mb.*t4346.*(t56+t65+B_cg_H.*t260+B_cg_H.*t803+dphi1.*t1456-dth1.*t1362)+ITail.*t5778.*(-t2361+t4138+(t1510.*(-t488+t603+dpsi1.*(t105-t465)+dth2.*(t103-t544)))./2.0)-Mb.*t5071.*(t412+t573+B_cg_H.*t1229-dphi1.*t3139+dpsi1.*t3206+dth1.*t1660+B_cg_H.*dth2.*t11.*t459)+Mb.*t5070.*(t411+t574-B_cg_H.*t1228+dphi1.*t3082+dpsi1.*t3138+dth1.*t1676+B_cg_H.*dth2.*t11.*t641);
et165 = -ITail.*(-t3471+t4531+t4422.*(t105-t465)).*(t2823./2.0+t3235./2.0-t4374./2.0+t4399./2.0+t4484./2.0-t4485./2.0)+Mt.*t4796.*(t56+t65+dth1.*(-t51+t394+t445-t527+t614)-dphi2.*t1618+dphi1.*t2360+dth2.*t876)-ITail.*t6252.*(-t3548+t4540+(t4422.*(t105-t465))./2.0)-Mt.*t5950.*(t412+t573-dth1.*(-t120+t425+t519-t651+t765)+dphi2.*t2915-dphi1.*t4115+dpsi1.*t4132+dth2.*t1381)+Mt.*t5952.*(t411+t574-dth1.*(-t130+t436+t523-t657+t769)-dphi2.*t2914+dphi1.*t4100+dpsi1.*t4112-dth2.*t1528)+Mm.*t4274.*(-t412+t502+dphi1.*t1169+dpsi1.*t1221-dth1.*t651);
et166 = -ITail.*t5782.*(t3265./2.0+t3771./2.0-t4480./2.0-t4556./2.0+(t1505.*(-t724-t778+t1230+t1291+dphi2.*(t534-t546)))./2.0+(t4437.*(t534-t546))./2.0)-ITail.*t5816.*(t3265+t3771-t4480-t4556+t1505.*(-t724-t778+t1230+t1291+dphi2.*(t534-t546))+t4437.*(t534-t546))+Mm.*t2062.*(t56+t65+dphi1.*t595-dth1.*t527)-Mm.*t4276.*(t411+t574+dpsi1.*(t530+t736)+dphi1.*t1170+dth1.*t657);
et167 = ITail.*(-t2274+t4111+t1510.*(-t488+t603+dpsi1.*(t105-t465)+dth2.*(t103-t544))).*(t1661./2.0+t1976./2.0+t3791./2.0+t3811./2.0-t4027./2.0+t4070./2.0);
et168 = t3906.*9.52624335e-4+t3930.*9.52624335e-4+t4393.*9.52624335e-4-t4395.*9.52624335e-4-t4536.*9.52624335e-4;
et169 = t4550.*9.52624335e-4;
et170 = t4704.*t4770.*2.0+t4753.*t4923.*2.0+t4313.*t5514.*2.0+t4770.*t6105.*2.0+t4313.*t6636.*2.0+t4923.*t6106.*2.0+t4447.*t6637.*2.0-t5351.*(-t1262+t1701+t9.*t868.*(t105-t465)).*2.0-t6635.*(-t1262+t1701+t9.*t868.*(t105-t465)).*2.0-t6104.*(t1260-t1328-t1427-t1441+t1706+t9.*t870.*(t105-t465)).*2.0+t4447.*(t2883+t2956-t3186-t3199+t3602+t3661).*2.0+(-t2388+t3008+t9.*t868.*(t105-t465).*9.53094055e-4).*(t1260-t1328-t1427-t1441+t1706+t9.*t870.*(t105-t465)).*2.0+ITail.*t4350.*t4770.*2.0+ITail.*t4313.*t4816.*2.0;
et171 = ITail.*t4459.*t4923.*2.0+ITail.*t4447.*t4961.*2.0-Mb.*t1918.*t1981.*2.0+Mb.*t2527.*t2638.*2.0+Mb.*t2563.*t2627.*2.0-Mm.*t852.*t855.*2.0+Mm.*t1007.*t1009.*2.0+Mm.*t1013.*t1016.*2.0-Mt.*t3483.*t3531.*2.0+Mt.*t3937.*t3969.*2.0+Mt.*t3940.*t3971.*2.0-ITail.*t4735.*(-t1262+t1701+t9.*t868.*(t105-t465)).*2.0+ITail.*(-t1355+t1789+(t9.*t868.*(t105-t465))./2.0).*(t1260-t1328-t1427-t1441+t1706+t9.*t870.*(t105-t465)).*2.0;
et172 = t1384.*2.0-t1664.*2.0-t1693.*2.0+t3657.*2.0-t4047.*2.0-t4059.*2.0-t4355.*2.0+t4479.*2.0+t4481.*2.0+t4704.*(t1064+t1137-t1694+t1698-t1763-t1774).*2.0+t6105.*(t1064+t1137-t1694+t1698-t1763-t1774).*2.0+t7.*t2597.*2.0-t2.*t2617.*2.0-t7.*t2660.*2.0+t4753.*t4897.*2.0-t4581.*t6104.*2.0-t4313.*t6616.*2.0+t4897.*t6106.*2.0-t4447.*t6617.*2.0-t4447.*(-t2503+t2754+t3433-t3460+t3506+t4.*t871.*(t534-t546).*9.52624335e-4).*2.0-t4313.*(-t2218+t2342+t3054+t3096+t3121+t3131).*2.0+t5208.*(-t1262+t1701+t9.*t868.*(t105-t465)).*2.0;
et173 = t6615.*(-t1262+t1701+t9.*t868.*(t105-t465)).*2.0+t2.*(t1223-t1252).*2.0+t4581.*(-t2388+t3008+t9.*t868.*(t105-t465).*9.53094055e-4).*2.0+ITail.*t4350.*(t1064+t1137-t1694+t1698-t1763-t1774).*2.0+ITail.*t4313.*(t1147+t1193-t1785+t1787-t1853-t1858).*2.0+ITail.*t4459.*t4897.*2.0+ITail.*t4447.*t4928.*2.0+ITail.*t4646.*(-t1262+t1701+t9.*t868.*(t105-t465)).*2.0+ITail.*t4581.*(-t1355+t1789+(t9.*t868.*(t105-t465))./2.0).*2.0;
et174 = t3034.*-2.0+t3739.*2.0+t3749.*2.0-t4323.*2.0+t4457.*2.0+t4458.*2.0-t4313.*t4701.*2.0-t4311.*t4704.*2.0+t4753.*t5022.*2.0+t4447.*t5799.*2.0-t4164.*t6104.*2.0-t4311.*t6105.*2.0-t4313.*t6389.*2.0-t4447.*t6399.*2.0+t5022.*t6106.*2.0+t4602.*(-t1262+t1701+t9.*t868.*(t105-t465)).*2.0+t6388.*(-t1262+t1701+t9.*t868.*(t105-t465)).*2.0+t4164.*(-t2388+t3008+t9.*t868.*(t105-t465).*9.53094055e-4).*2.0-ITail.*t4313.*t4343.*2.0-ITail.*t4311.*t4350.*2.0+ITail.*t4459.*t5022.*2.0+ITail.*t4447.*t5089.*2.0+ITail.*t4227.*(-t1262+t1701+t9.*t868.*(t105-t465)).*2.0;
et175 = ITail.*t4164.*(-t1355+t1789+(t9.*t868.*(t105-t465))./2.0).*2.0;
et176 = t2889.*2.0+t3403.*2.0+t3415.*2.0+t4236.*2.0+t4354.*2.0+t4356.*2.0-(-t1262+t1701+t9.*t868.*(t105-t465)).*(t1832.*3.372786875e-3+t1866.*3.36554e-3-t1962+t2131+t2287+t2339-t2463+t2495+t2571-t2679+t2692+t2945+t2981-t3252+t3311+t3326+t3344+t496.*(t214-t541).*3.36554e-3).*2.0;
et177 = t4313.*(t1832.*3.36554e-3+t1866.*3.36554e-3+t1983-t2150-t2322+t2339+t2430-t2472+t2479+t2495+t2785+t2803+t2981-t3252+t3311+t3482+t3485+t496.*(t214-t541).*3.367829185e-3).*2.0-t4704.*t4738.*2.0+t4753.*t4823.*2.0-t4313.*t5474.*2.0+t4447.*t5566.*2.0+t4695.*t6104.*2.0-t4738.*t6105.*2.0+t4823.*t6106.*2.0;
et178 = (-t1262+t1701+t9.*t868.*(t105-t465)).*(t2135-t2468+t2699+t2738+t2950+t3105).*-2.0-t4695.*(-t2388+t3008+t9.*t868.*(t105-t465).*9.53094055e-4).*2.0;
et179 = t4447.*(t1832.*3.36554e-3+t1866.*3.372816795e-3-t1962+t1983+t2287-t2322-t2472+t2479+t2512+t2571+t2722+t2803+t3122+t3326+t3344-t3357+t3423+t496.*(t214-t541).*3.36554e-3).*2.0-ITail.*t4350.*t4738.*2.0-ITail.*t4313.*t4783.*2.0+ITail.*t4459.*t4823.*2.0+ITail.*t4447.*t4882.*2.0-ITail.*t4722.*(-t1262+t1701+t9.*t868.*(t105-t465)).*2.0;
et180 = ITail.*t4695.*(-t1355+t1789+(t9.*t868.*(t105-t465))./2.0).*-2.0;
et181 = -t1939+t2390+t2843-t2877+t3263+t3931+t4054+t4273+t4301-t4324+t4945+t4964+t5300-t5354-t5382+t5627+t5665+t5705-t5738+t5891+t6049-t6286+t6325+t6381-t6445-t6640+t6668-t6734+t4753.*(-t1129+t1139-t2082+t2110+t2123+t8.*t872.*(t534-t546))+t6106.*(-t1129+t1139-t2082+t2110+t2123+t8.*t872.*(t534-t546))+t4313.*(t2208+t2312-t3315+t3347+t3475+t1179.*(t103-t544).*8.56645e-6);
et182 = t4447.*(t2215-t2237+t3424+t3427-t3439+t8.*t872.*(t534-t546).*9.52624335e-4)+t4704.*(t1060+t1138-t1883+t1932+t2088+t1179.*(t103-t544))+t6105.*(t1060+t1138-t1883+t1932+t2088+t1179.*(t103-t544))+t4936.*(-t1262+t1701+t9.*t868.*(t105-t465));
et183 = t4447.*(t1645+t1965+t2072+t2220-t2242-t2409-t2483-t2504-t3093+t3155+t3261+t3432+t3437-t3442+t1179.*(t103-t544).*3.36554e-3+t3.*t575.*(t105-t465).*3.36554e-3+t8.*t872.*(t534-t546).*3.372816795e-3);
et184 = t4454.*(-t2388+t3008+t9.*t868.*(t105-t465).*9.53094055e-4);
et185 = t4313.*(t1645+t2037-t2064+t2156+t2227-t2409-t2483-t2504-t3244+t3270-t3276+t3299+t3312+t3413+t1179.*(t103-t544).*3.367829185e-3+t3.*t575.*(t105-t465).*3.36554e-3+t8.*t872.*(t534-t546).*3.36554e-3)+t6616.*(-t1331+t2317+t1510.*(t103-t544));
et186 = (-t1331+t2317+t1510.*(t103-t544)).*(-t2218+t2342+t3054+t3096+t3121+t3131)+Mt.*(t433-t828+T_cg_H.*(t197-t537)).*(-t130+t436+t523-t657+t769)+ITail.*t4459.*(-t1129+t1139-t2082+t2110+t2123+t8.*t872.*(t534-t546))+ITail.*t4447.*(-t1189+t1195-t2210+t2241+t2248+(t8.*t872.*(t534-t546))./2.0)+ITail.*t4350.*(t1060+t1138-t1883+t1932+t2088+t1179.*(t103-t544))+ITail.*t4313.*(t1143+t1194-t1959+t2038+t2175+(t1179.*(t103-t544))./2.0)+ITail.*t4490.*(-t1262+t1701+t9.*t868.*(t105-t465))+ITail.*t4454.*(-t1355+t1789+(t9.*t868.*(t105-t465))./2.0)+B_cg_H.*Mb.*t11.*t641.*t2563;
et187 = t2104.*(-3.367829185e-3)+t2191.*3.367829185e-3-t3879.*3.367829185e-3-t3936.*3.367829185e-3+t3948.*3.367829185e-3+t4073+t4084+t4212+t4224+t4418+t4444+t4514;
et188 = t4521+t4585+t4596+t4640+t4652+t1037.*(-t488+t603+dpsi1.*(t105-t465)+dth2.*(t103-t544)).*3.367829185e-3;
et189 = t3521.*9.53094055e-4-t3524.*9.53094055e-4-t4300.*9.53094055e-4+t4483.*9.53094055e-4+t4498.*9.53094055e-4;
et190 = t4098.*(t105-t465).*(-9.53094055e-4);
et191 = t3341+t3392+t3521.*3.372786875e-3-t3524.*3.372786875e-3+t4208+t4212+t4217+t4224+t4233+t4256-t4300.*3.372786875e-3+t4483.*3.372786875e-3+t4498.*3.372786875e-3;
et192 = t4514+t4521+t4640+t4652-t4098.*(t105-t465).*3.372786875e-3;
et193 = t2104.*8.56645e-6-t2191.*8.56645e-6+t3879.*8.56645e-6+t3936.*8.56645e-6;
et194 = t3948.*(-8.56645e-6)-t1037.*(-t488+t603+dpsi1.*(t105-t465)+dth2.*(t103-t544)).*8.56645e-6;
et195 = t3341+t3392+t3906.*3.372816795e-3+t3930.*3.372816795e-3+t4073+t4084+t4208+t4217+t4233+t4256+t4393.*3.372816795e-3-t4395.*3.372816795e-3+t4418+t4444;
et196 = t4536.*(-3.372816795e-3)+t4550.*3.372816795e-3+t4585+t4596;
et197 = dphi1.*3.92433573e-3+t24.*2.3495e-8+t26.*1.8563e-7+t27.*3.92433573e-3;
et198 = t54.*1.8563e-7-t61.*2.3495e-8;
et199 = -t5782.*(et168+et169)+dth1.*(dth1.*(et170+et171)+dphi1.*(et172+et173)+dx.*(t952.*2.0+t1159.*2.0+t1173.*2.0+t2148.*2.0+t2799.*2.0+t2816.*2.0+t3644.*2.0+t4028.*2.0+t4036.*2.0)-dy.*(t1008.*-2.0+t1206.*2.0+t1247.*2.0-t2225.*2.0+t2849.*2.0+t2878.*2.0-t3704.*2.0+t4052.*2.0+t4058.*2.0)+dz.*(t1005.*-2.0+t1203.*2.0+t1245.*2.0-t2222.*2.0+t2847.*2.0+t2876.*2.0-t3701.*2.0+t4051.*2.0+t4056.*2.0)+dphi2.*(et174+et175)+dth2.*(et176+et177+et178+et179+et180))+t6239.*(-t4087+t4644+t4422.*(t105-t465).*9.53094055e-4);
et200 = -t55.*(dpsi1.*t5.*3.92433573e-3-t2.*t27.*1.8563e-7+t27.*t1374)+dphi2.*t6895-dphi1.*t6902-dpsi1.*t6899-dx.*t6792-dy.*t6797-dz.*t6798-t5997.*t6374+t5847.*t6783-t6239.*t6782-t6374.*t6784;
et201 = -dth2.*(t4786-t4790+t6845-t6880-t6885+dphi1.*(et181+et182+et183+et184+et185+et186)+dx.*(-t754+t1167-t1635+t2574+Mt.*t9.*t10.*(t433-t828+T_cg_H.*(t197-t537))+B_cg_H.*Mb.*t9.*t10.*(t197-t537)))+t304.*(dpsi1.*t5.*(-1.8563e-7)+t27.*t1215+t27.*t1253)-(-t2274+t4111+t1510.*(-t488+t603+dpsi1.*(t105-t465)+dth2.*(t103-t544))).*(et187+et188);
et202 = t5847.*(-t3614+t4341+t1510.*(-t488+t603+dpsi1.*(t105-t465)+dth2.*(t103-t544)).*8.56645e-6)+(-t3471+t4531+t4422.*(t105-t465)).*(et189+et190)+(-t3471+t4531+t4422.*(t105-t465)).*(et191+et192)+(-t2274+t4111+t1510.*(-t488+t603+dpsi1.*(t105-t465)+dth2.*(t103-t544))).*(et193+et194)-t5782.*(et195+et196)-t383.*(dpsi1.*t1371+t27.*t1234+t27.*t1252)+ITail.*t5847.*(-t2361+t4138+(t1510.*(-t488+t603+dpsi1.*(t105-t465)+dth2.*(t103-t544)))./2.0);
et203 = Mb.*t5071.*(t68+t134+t276+B_cg_H.*t1097-dphi1.*t1660-dpsi1.*t2563+dth1.*t2638+B_cg_H.*dth2.*t675)-Mb.*t5070.*(t73+t144+t277+B_cg_H.*t1108-dphi1.*t1676+dpsi1.*t2527+dth1.*t2627+B_cg_H.*dth2.*t721)+ITail.*t6239.*(-t3548+t4540+(t4422.*(t105-t465))./2.0)-Mm.*t2062.*(t25+t71+t161+dphi1.*t527-dth1.*t852)+ITail.*(-t2274+t4111+t1510.*(-t488+t603+dpsi1.*(t105-t465)+dth2.*(t103-t544))).*(t2104./2.0-t2191./2.0+t3879./2.0+t3936./2.0-t3948./2.0-(t1037.*(-t488+t603+dpsi1.*(t105-t465)+dth2.*(t103-t544)))./2.0);
et204 = -ITail.*t5782.*(t3906./2.0+t3930./2.0+t4393./2.0-t4395./2.0-t4536./2.0+t4550./2.0)+Mm.*t4274.*(t68+t134+t276-dphi1.*t651-dpsi1.*t1013+dth1.*t1009)+Mm.*t4276.*(t73+t144+t277-dphi1.*t657+dpsi1.*t1007+dth1.*t1016)-ITail.*t5816.*t6374-Mt.*t4796.*(t25+t71+t161-dphi1.*(-t51+t394+t445-t527+t614)-dphi2.*t2087+dth2.*t1620-dth1.*t3483)+t2.*t27.*t4597-t7.*t27.*t4603-dpsi1.*t5.*(et197+et198)+ITail.*(-t3471+t4531+t4422.*(t105-t465)).*(t3521./2.0-t3524./2.0-t4300./2.0+t4483./2.0+t4498./2.0-(t4098.*(t105-t465))./2.0);
et205 = -Mb.*t4346.*(t25+t71+t161-B_cg_H.*t901+dphi1.*t1362-dth1.*t1918+B_cg_H.*dth2.*t558)+Mt.*t5950.*(t68+t134+t276+dphi1.*(-t120+t425+t519-t651+t765)+dphi2.*t2763-dpsi1.*t3937+dth2.*t1727+dth1.*t3971)-Mt.*t5952.*(t73+t144+t277+dphi1.*(-t130+t436+t523-t657+t769)+dphi2.*t2730+dpsi1.*t3940+dth2.*t1734+dth1.*t3969);
et206 = t4592.*(t2449.*3.36554e-3+t3490+t3648+t3649-t3934-t3966).*-2.0+t4785.*(t2449.*3.36554e-3+t3490+t3544+t3545-t4001-t4034).*2.0+t4575.*(t2449.*3.372786875e-3+t3544+t3545+t3598-t3934-t3966).*2.0+t10.*t3982.*2.0+t10.*t4014.*2.0+t4500.*t4575.*2.0-t4518.*t4592.*2.0+t4173.*t4949.*2.0-t4162.*t4980.*2.0-t4634.*t4785.*2.0-t4392.*t5216.*2.0+t4162.*t6457.*2.0+t4173.*t6458.*2.0;
et207 = t4392.*t6456.*-2.0-t10.*(t5.*3.92433573e-3-t2.*t10.*1.8563e-7+t10.*t1374).*2.0-t5.*(t10.*3.92433573e-3-t5.*t7.*2.3495e-8+t5.*t1343).*2.0+ITail.*t4214.*t4575.*2.0+ITail.*t4173.*t4617.*2.0;
et208 = ITail.*t4162.*t4629.*-2.0-ITail.*t4215.*t4592.*2.0-ITail.*t4409.*t4785.*2.0-ITail.*t4392.*t4814.*2.0+Mb.*t2527.*t3848.*2.0+Mb.*t2563.*t3836.*2.0+Mm.*t1007.*t1394.*2.0-Mm.*t1013.*t1470.*2.0+Mt.*t3937.*t4344.*2.0+Mt.*t3940.*t4357.*2.0+t2.*t5.*t3944.*2.0+t5.*t7.*t3955.*2.0;
et209 = t2927+t3062-t3494+t3584+t3597-t3652+t964.*(t105-t465).*3.372786875e-3+t977.*(t105-t465).*3.36554e-3+t1430.*(t103-t544).*3.372786875e-3+t1512.*(t103-t544).*3.36554e-3;
et210 = t1510.*(t197-t537).*3.36554e-3+t1505.*(t214-t541).*3.36554e-3;
et211 = t2920+t2927+t3489-t3494+t3722-t3784+t964.*(t105-t465).*3.36554e-3+t977.*(t105-t465).*3.36554e-3+t1430.*(t103-t544).*3.36554e-3+t1512.*(t103-t544).*3.36554e-3;
et212 = t1510.*(t197-t537).*3.372816795e-3+t1505.*(t214-t541).*3.372816795e-3;
et213 = t2920+t3084+t3489-t3578+t3584-t3652+t964.*(t105-t465).*3.36554e-3+t977.*(t105-t465).*3.367829185e-3+t1430.*(t103-t544).*3.36554e-3+t1512.*(t103-t544).*3.367829185e-3;
et214 = t1510.*(t197-t537).*3.36554e-3+t1505.*(t214-t541).*3.36554e-3;
et215 = t4173.*(et209+et210).*-2.0-t4500.*(t1751+t2308+t964.*(t105-t465)+t1430.*(t103-t544)).*2.0+t4645.*(t2449.*3.36554e-3+t3490+t3648+t3649-t3934-t3966).*2.0+t4392.*(et211+et212).*2.0-(t2436-t2536+t1510.*(t197-t537)+t1505.*(t214-t541)).*(t2449.*3.36554e-3+t3490+t3544+t3545-t4001-t4034).*2.0+t4518.*t4645.*2.0+t4162.*t5023.*2.0+t4634.*(t2436-t2536+t1510.*(t197-t537)+t1505.*(t214-t541)).*2.0;
et216 = t4173.*(t3070+t3563+t964.*(t105-t465).*9.53094055e-4+t1430.*(t103-t544).*9.53094055e-4).*-2.0+t4392.*(t3716-t3777+t1510.*(t197-t537).*9.52624335e-4+t1505.*(t214-t541).*9.52624335e-4).*2.0-t4162.*(et213+et214).*2.0;
et217 = (t1751+t2308+t964.*(t105-t465)+t1430.*(t103-t544)).*(t2449.*3.372786875e-3+t3544+t3545+t3598-t3934-t3966).*-2.0+Mt.*t4344.*(t433-t828+T_cg_H.*(t197-t537)).*2.0-ITail.*t4214.*(t1751+t2308+t964.*(t105-t465)+t1430.*(t103-t544)).*2.0-ITail.*t4173.*(t1846+t2413+(t964.*(t105-t465))./2.0+(t1430.*(t103-t544))./2.0).*2.0+ITail.*t4162.*t4675.*2.0+ITail.*t4215.*t4645.*2.0+Mt.*t2319.*t4357.*2.0+ITail.*t4409.*(t2436-t2536+t1510.*(t197-t537)+t1505.*(t214-t541)).*2.0;
et218 = ITail.*t4392.*(t2582-t2684+(t1510.*(t197-t537))./2.0+(t1505.*(t214-t541))./2.0).*2.0+B_cg_H.*Mb.*t3836.*(t197-t537).*2.0+B_cg_H.*Mb.*t964.*t3848.*2.0;
et219 = t4173.*(t2449.*3.36554e-3+t3490+t3648+t3649-t3934-t3966).*-2.0+t4162.*(t2449.*3.372786875e-3+t3544+t3545+t3598-t3934-t3966).*2.0+t4162.*t4500.*2.0+t4173.*t4505.*2.0-t4162.*t4517.*2.0-t4173.*t4518.*2.0+t4392.*(t2449.*3.36554e-3+t3490+t3556+t3557).*2.0;
et220 = t4162.*(t2449.*3.367829185e-3+t3556+t3557+t3576).*-2.0-t4173.*(t2449.*3.36554e-3+t3490-t3632+t1510.*(t105-t465).*3.372786875e-3).*2.0+Mt.*t3780.*t4344.*2.0+Mt.*t3774.*t4357.*2.0+B_cg_H.*Mb.*t1512.*t3836.*2.0+B_cg_H.*Mb.*t1510.*t3848.*2.0;
et221 = t4618.*(t2449.*3.36554e-3+t3490+t3648+t3649-t3934-t3966).*2.0+t4830.*(t2449.*3.36554e-3+t3490+t3544+t3545-t4001-t4034).*2.0+t4638.*(t2449.*3.372786875e-3+t3544+t3545+t3598-t3934-t3966).*2.0+t4518.*t4618.*2.0+t4500.*t4638.*2.0+t4173.*t4989.*2.0+t4162.*t5006.*2.0-t4634.*t4830.*2.0-t4392.*t5313.*2.0+t4162.*t6485.*2.0+t4173.*t6486.*2.0-t4392.*t6487.*2.0;
et222 = t10.*(t7.*t1345+t5.*t1370).*-2.0+t5.*t7.*(t1283+t5.*t1268).*2.0+Mm.*t1394.*(t530+t736).*2.0+t2.*t5.*(t1322-t5.*t7.*1.19846373e-3).*2.0+ITail.*t4162.*t4657.*2.0+ITail.*t4215.*t4618.*2.0+ITail.*t4173.*t4667.*2.0+ITail.*t4214.*t4638.*2.0-ITail.*t4409.*t4830.*2.0-ITail.*t4392.*t4881.*2.0+Mb.*t3138.*t3848.*2.0-Mb.*t3206.*t3836.*2.0-Mm.*t1221.*t1470.*2.0+Mt.*t4112.*t4357.*2.0-Mt.*t4132.*t4344.*2.0-t5.*t7.*t3932.*2.0+t2.*t5.*t3965.*2.0;
et223 = t3862.*9.52624335e-4+t3907.*9.52624335e-4-t4576.*9.52624335e-4-t4577.*9.52624335e-4+t4588.*9.52624335e-4;
et224 = t4591.*9.52624335e-4;
et225 = t1593.*2.0-t2970.*2.0+t2972.*2.0+t3902.*2.0-t4439.*2.0+t4440.*2.0+t3938.*(t2587-t3868+t1505.*(t534-t546).*1.90524867e-3).*2.0+t3938.*t6124.*2.0-(-t2389+t3634+t1512.*(t105-t465).*9.53094055e-4).*(t1079+t1956-t4277-t1178.*(t105-t465)).*2.0+t5442.*(t1079+t1956-t4277-t1178.*(t105-t465)).*2.0-t6137.*(t1332+t2368+t1512.*(t105-t465)).*2.0;
et226 = (t1332+t2368+t1512.*(t105-t465)).*(t2134-t2147+t3286+t3329+t3378-t1178.*(t105-t465).*9.53094055e-4).*-2.0+t4555.*(t1395-t2868+t1505.*(t534-t546).*2.0).*2.0+t5434.*(t1395-t2868+t1505.*(t534-t546).*2.0).*2.0+ITail.*t3938.*(t1365-t2831+t1505.*(t534-t546)).*2.0+ITail.*t4077.*(t1395-t2868+t1505.*(t534-t546).*2.0).*2.0-ITail.*(t1386+t2501+(t1512.*(t105-t465))./2.0).*(t1079+t1956-t4277-t1178.*(t105-t465)).*2.0;
et227 = ITail.*(t1332+t2368+t1512.*(t105-t465)).*(t1153+t2075-t4310-(t1178.*(t105-t465))./2.0).*-2.0;
et228 = t1718.*-2.0+t2796.*2.0+t2811.*2.0-t4090.*2.0+t4412.*2.0+t4414.*2.0+t3938.*t4775.*2.0+t4471.*t4555.*2.0+t4471.*t5434.*2.0+t3938.*t6125.*2.0+(-t2389+t3634+t1512.*(t105-t465).*9.53094055e-4).*(t1185+t1813-t4313+t1047.*(t105-t465)).*2.0-t5442.*(t1185+t1813-t4313+t1047.*(t105-t465)).*2.0-t5519.*(t1332+t2368+t1512.*(t105-t465)).*2.0-t6138.*(t1332+t2368+t1512.*(t105-t465)).*2.0+ITail.*t3938.*t4461.*2.0+ITail.*t4077.*t4471.*2.0+ITail.*(t1332+t2368+t1512.*(t105-t465)).*(t1264+t1882-t4350+(t1047.*(t105-t465))./2.0).*2.0;
et229 = ITail.*(t1386+t2501+(t1512.*(t105-t465))./2.0).*(t1185+t1813-t4313+t1047.*(t105-t465)).*2.0;
et230 = t3938.*t4858.*2.0+t4555.*t4578.*2.0+t3938.*t5829.*2.0+t4578.*t5434.*2.0+(t2387-t3667+t1430.*(t105-t465).*9.53094055e-4).*(t1332+t2368+t1512.*(t105-t465)).*2.0-t5823.*(t1332+t2368+t1512.*(t105-t465)).*2.0+(t1260-t2364+t1430.*(t105-t465)).*(-t2389+t3634+t1512.*(t105-t465).*9.53094055e-4).*2.0-t5442.*(t1260-t2364+t1430.*(t105-t465)).*2.0;
et231 = ITail.*(t1260-t2364+t1430.*(t105-t465)).*(t1386+t2501+(t1512.*(t105-t465))./2.0).*2.0+ITail.*(t1352-t2496+(t1430.*(t105-t465))./2.0).*(t1332+t2368+t1512.*(t105-t465)).*2.0+ITail.*t3938.*t4573.*2.0+ITail.*t4077.*t4578.*2.0-Mb.*t15.*t1654.*2.0+Mb.*t15.*t3169-Mb.*t15.*t3192.*2.0-Mt.*t2203.*t2240.*2.0+Mt.*t3679.*t3780.*2.0-Mt.*t3770.*t3774.*2.0;
et232 = t1521.*-2.0+t2737.*2.0-t3858.*2.0+t4379.*2.0+t3938.*(t2591-t3773+t1430.*(t197-t537).*1.90524867e-3).*2.0+t4820.*(-t2389+t3634+t1512.*(t105-t465).*9.53094055e-4).*2.0-t3938.*t6117.*2.0-t4820.*t5442.*2.0+t5548.*(t1332+t2368+t1512.*(t105-t465)).*2.0+t6129.*(t1332+t2368+t1512.*(t105-t465)).*2.0+t4555.*(t1396-t2573+t1430.*(t197-t537).*2.0).*2.0+t5434.*(t1396-t2573+t1430.*(t197-t537).*2.0).*2.0;
et233 = Mt.*t3780.*(t451-t831+T_cg_H.*(t214-t541)).*2.0+ITail.*t3938.*(t1368-t2524+t1430.*(t197-t537)).*2.0+ITail.*t4077.*(t1396-t2573+t1430.*(t197-t537).*2.0).*2.0+ITail.*t4867.*(t1332+t2368+t1512.*(t105-t465)).*2.0+ITail.*t4820.*(t1386+t2501+(t1512.*(t105-t465))./2.0).*2.0+Mb.*t15.*t1512.*(t214-t541).*2.0;
et234 = t3448+t3862.*3.372816795e-3+t3907.*3.372816795e-3+t4083+t4309+t4326-t4576.*3.372816795e-3-t4577.*3.372816795e-3+t4588.*3.372816795e-3;
et235 = t4591.*3.372816795e-3+t4606+t4623;
et236 = t1309+t1929+t2282-t2348+t3325+t3957+t3985+t4010+t4257+t4268+t4502+t4503-t5274+t5280-t5294+t5308-t5644+t5648-t5917+t5926+t6077-t6147+t6219-t6304-t6311-t6658+t4476.*(t2591-t3773+t1430.*(t197-t537).*1.90524867e-3);
et237 = t4820.*(t1970-t1971+t2487+t3161-t3236-t3794-t3817+t1240.*(t105-t465).*3.372786875e-3+t903.*(t534-t546).*3.372786875e-3);
et238 = t4820.*(-t1974+t1240.*(t105-t465).*9.53094055e-4+t903.*(t534-t546).*9.53094055e-4)+t6611.*(t1332+t2368+t1512.*(t105-t465))+t5394.*(t820+t1121-t1435+t1997+t2000+t11.*t420.*(t214-t541))+t4787.*(t1396-t2573+t1430.*(t197-t537).*2.0)+t5548.*(-t947+t1240.*(t105-t465)+t903.*(t534-t546))+t6129.*(-t947+t1240.*(t105-t465)+t903.*(t534-t546));
